simulink model "object_frame_impedance"  (R2025a)
(part 3 of 6)

  + (x1z + (-1) .* x3z) .^ 2) .^ (-1 / 2) .* (x1z + (-1) .* x3z) + ( ...
  (x2x + (-1) .* x4x) .^ 2 + (x2y + (-1) .* x4y) .^ 2 + (x2z + (-1)  ...
  .* x4z) .^ 2) .^ (-1 / 2) .* (x2z + (-1) .* x4z)) + (-1 / 2) .* (( ...
  ((-1) .* x1y + x3y) .* (x2x + (-1) .* x4x) + (x1x + (-1) .* x3x)  ...
  .* (x2y + (-1) .* x4y)) .^ 2 + ((x1z + (-1) .* x3z) .* (x2x + (-1) ...
   .* x4x) + (-1) .* (x1x + (-1) .* x3x) .* (x2z + (-1) .* x4z)) .^  ...
  2 + (((-1) .* x1z + x3z) .* (x2y + (-1) .* x4y) + (x1y + (-1) .*  ...
  x3y) .* (x2z + (-1) .* x4z)) .^ 2) .^ (-1 / 2) .* (((x1x + (-1) .* ...
   x3x) .* ((x1x + (-1) .* x3x) .^ 2 + (x1y + (-1) .* x3y) .^ 2 + ( ...
  x1z + (-1) .* x3z) .^ 2) .^ (-1 / 2) + (x2x + (-1) .* x4x) .* (( ...
  x2x + (-1) .* x4x) .^ 2 + (x2y + (-1) .* x4y) .^ 2 + (x2z + (-1)  ...
  .* x4z) .^ 2) .^ (-1 / 2)) .^ 2 + ((x1y + (-1) .* x3y) .* ((x1x +  ...
  (-1) .* x3x) .^ 2 + (x1y + (-1) .* x3y) .^ 2 + (x1z + (-1) .* x3z) ...
   .^ 2) .^ (-1 / 2) + (x2y + (-1) .* x4y) .* ((x2x + (-1) .* x4x)  ...
  .^ 2 + (x2y + (-1) .* x4y) .^ 2 + (x2z + (-1) .* x4z) .^ 2) .^ ( ...
  -1 / 2)) .^ 2 + (((x1x + (-1) .* x3x) .^ 2 + (x1y + (-1) .* x3y)  ...
  .^ 2 + (x1z + (-1) .* x3z) .^ 2) .^ (-1 / 2) .* (x1z + (-1) .*  ...
  x3z) + ((x2x + (-1) .* x4x) .^ 2 + (x2y + (-1) .* x4y) .^ 2 + ( ...
  x2z + (-1) .* x4z) .^ 2) .^ (-1 / 2) .* (x2z + (-1) .* x4z)) .^ 2) ...
   .^ (-3 / 2) .* ((x1z + (-1) .* x3z) .* (x2x + (-1) .* x4x) + (-1) ...
   .* (x1x + (-1) .* x3x) .* (x2z + (-1) .* x4z)) .* (2 .* ((x2x + ( ...
  -1) .* x4x) .^ 2 .* ((x2x + (-1) .* x4x) .^ 2 + (x2y + (-1) .*  ...
  x4y) .^ 2 + (x2z + (-1) .* x4z) .^ 2) .^ (-3 / 2) + (-1) .* ((x2x  ...
  + (-1) .* x4x) .^ 2 + (x2y + (-1) .* x4y) .^ 2 + (x2z + (-1) .*  ...
  x4z) .^ 2) .^ (-1 / 2)) .* ((x1x + (-1) .* x3x) .* ((x1x + (-1) .* ...
   x3x) .^ 2 + (x1y + (-1) .* x3y) .^ 2 + (x1z + (-1) .* x3z) .^ 2)  ...
  .^ (-1 / 2) + (x2x + (-1) .* x4x) .* ((x2x + (-1) .* x4x) .^ 2 + ( ...
  x2y + (-1) .* x4y) .^ 2 + (x2z + (-1) .* x4z) .^ 2) .^ (-1 / 2)) + ...
   2 .* (x2x + (-1) .* x4x) .* (x2y + (-1) .* x4y) .* ((x1y + (-1)  ...
  .* x3y) .* ((x1x + (-1) .* x3x) .^ 2 + (x1y + (-1) .* x3y) .^ 2 +  ...
  (x1z + (-1) .* x3z) .^ 2) .^ (-1 / 2) + (x2y + (-1) .* x4y) .* (( ...
  x2x + (-1) .* x4x) .^ 2 + (x2y + (-1) .* x4y) .^ 2 + (x2z + (-1)  ...
  .* x4z) .^ 2) .^ (-1 / 2)) .* ((x2x + (-1) .* x4x) .^ 2 + (x2y + ( ...
  -1) .* x4y) .^ 2 + (x2z + (-1) .* x4z) .^ 2) .^ (-3 / 2) + 2 .* ( ...
  x2x + (-1) .* x4x) .* (((x1x + (-1) .* x3x) .^ 2 + (x1y + (-1) .*  ...
  x3y) .^ 2 + (x1z + (-1) .* x3z) .^ 2) .^ (-1 / 2) .* (x1z + (-1)  ...
  .* x3z) + ((x2x + (-1) .* x4x) .^ 2 + (x2y + (-1) .* x4y) .^ 2 + ( ...
  x2z + (-1) .* x4z) .^ 2) .^ (-1 / 2) .* (x2z + (-1) .* x4z)) .* (( ...
  x2x + (-1) .* x4x) .^ 2 + (x2y + (-1) .* x4y) .^ 2 + (x2z + (-1)  ...
  .* x4z) .^ 2) .^ (-3 / 2) .* (x2z + (-1) .* x4z)) .* (((x1x + (-1) ...
   .* x3x) .^ 2 + (x1y + (-1) .* x3y) .^ 2 + (x1z + (-1) .* x3z) .^  ...
  2) .^ (-1 / 2) .* (x1z + (-1) .* x3z) + ((x2x + (-1) .* x4x) .^ 2  ...
  + (x2y + (-1) .* x4y) .^ 2 + (x2z + (-1) .* x4z) .^ 2) .^ (-1 / 2) ...
   .* (x2z + (-1) .* x4z)) + (-1) .* (x2x + (-1) .* x4x) .* (((-1)  ...
  .* x1y + x3y) .* (x2x + (-1) .* x4x) + (x1x + (-1) .* x3x) .* ( ...
  x2y + (-1) .* x4y)) .* (x2y + (-1) .* x4y) .* ((((-1) .* x1y +  ...
  x3y) .* (x2x + (-1) .* x4x) + (x1x + (-1) .* x3x) .* (x2y + (-1)  ...
  .* x4y)) .^ 2 + ((x1z + (-1) .* x3z) .* (x2x + (-1) .* x4x) + (-1) ...
   .* (x1x + (-1) .* x3x) .* (x2z + (-1) .* x4z)) .^ 2 + (((-1) .*  ...
  x1z + x3z) .* (x2y + (-1) .* x4y) + (x1y + (-1) .* x3y) .* (x2z +  ...
  (-1) .* x4z)) .^ 2) .^ (-1 / 2) .* (((x1x + (-1) .* x3x) .* ((x1x  ...
  + (-1) .* x3x) .^ 2 + (x1y + (-1) .* x3y) .^ 2 + (x1z + (-1) .*  ...
  x3z) .^ 2) .^ (-1 / 2) + (x2x + (-1) .* x4x) .* ((x2x + (-1) .*  ...
  x4x) .^ 2 + (x2y + (-1) .* x4y) .^ 2 + (x2z + (-1) .* x4z) .^ 2)  ...
  .^ (-1 / 2)) .^ 2 + ((x1y + (-1) .* x3y) .* ((x1x + (-1) .* x3x)  ...
  .^ 2 + (x1y + (-1) .* x3y) .^ 2 + (x1z + (-1) .* x3z) .^ 2) .^ ( ...
  -1 / 2) + (x2y + (-1) .* x4y) .* ((x2x + (-1) .* x4x) .^ 2 + (x2y  ...
  + (-1) .* x4y) .^ 2 + (x2z + (-1) .* x4z) .^ 2) .^ (-1 / 2)) .^ 2  ...
  + (((x1x + (-1) .* x3x) .^ 2 + (x1y + (-1) .* x3y) .^ 2 + (x1z + ( ...
  -1) .* x3z) .^ 2) .^ (-1 / 2) .* (x1z + (-1) .* x3z) + ((x2x + ( ...
  -1) .* x4x) .^ 2 + (x2y + (-1) .* x4y) .^ 2 + (x2z + (-1) .* x4z)  ...
  .^ 2) .^ (-1 / 2) .* (x2z + (-1) .* x4z)) .^ 2) .^ (-1 / 2) .* (( ...
  x2x + (-1) .* x4x) .^ 2 + (x2y + (-1) .* x4y) .^ 2 + (x2z + (-1)  ...
  .* x4z) .^ 2) .^ (-3 / 2) + (x2x + (-1) .* x4x) .* ((((-1) .* x1y  ...
  + x3y) .* (x2x + (-1) .* x4x) + (x1x + (-1) .* x3x) .* (x2y + (-1) ...
   .* x4y)) .^ 2 + ((x1z + (-1) .* x3z) .* (x2x + (-1) .* x4x) + ( ...
  -1) .* (x1x + (-1) .* x3x) .* (x2z + (-1) .* x4z)) .^ 2 + (((-1)  ...
  .* x1z + x3z) .* (x2y + (-1) .* x4y) + (x1y + (-1) .* x3y) .* ( ...
  x2z + (-1) .* x4z)) .^ 2) .^ (-1 / 2) .* (((x1x + (-1) .* x3x) .*  ...
  ((x1x + (-1) .* x3x) .^ 2 + (x1y + (-1) .* x3y) .^ 2 + (x1z + (-1) ...
   .* x3z) .^ 2) .^ (-1 / 2) + (x2x + (-1) .* x4x) .* ((x2x + (-1)  ...
  .* x4x) .^ 2 + (x2y + (-1) .* x4y) .^ 2 + (x2z + (-1) .* x4z) .^  ...
  2) .^ (-1 / 2)) .^ 2 + ((x1y + (-1) .* x3y) .* ((x1x + (-1) .*  ...
  x3x) .^ 2 + (x1y + (-1) .* x3y) .^ 2 + (x1z + (-1) .* x3z) .^ 2)  ...
  .^ (-1 / 2) + (x2y + (-1) .* x4y) .* ((x2x + (-1) .* x4x) .^ 2 + ( ...
  x2y + (-1) .* x4y) .^ 2 + (x2z + (-1) .* x4z) .^ 2) .^ (-1 / 2))  ...
  .^ 2 + (((x1x + (-1) .* x3x) .^ 2 + (x1y + (-1) .* x3y) .^ 2 + ( ...
  x1z + (-1) .* x3z) .^ 2) .^ (-1 / 2) .* (x1z + (-1) .* x3z) + (( ...
  x2x + (-1) .* x4x) .^ 2 + (x2y + (-1) .* x4y) .^ 2 + (x2z + (-1)  ...
  .* x4z) .^ 2) .^ (-1 / 2) .* (x2z + (-1) .* x4z)) .^ 2) .^ (-1 /  ...
  2) .* ((x1z + (-1) .* x3z) .* (x2x + (-1) .* x4x) + (-1) .* (x1x + ...
   (-1) .* x3x) .* (x2z + (-1) .* x4z)) .* ((x2x + (-1) .* x4x) .^  ...
  2 + (x2y + (-1) .* x4y) .^ 2 + (x2z + (-1) .* x4z) .^ 2) .^ (-3 /  ...
  2) .* (x2z + (-1) .* x4z),(-1) .* (((-1) .* x1y + x3y) .* (x2x + ( ...
  -1) .* x4x) + (x1x + (-1) .* x3x) .* (x2y + (-1) .* x4y)) .* (((( ...
  -1) .* x1y + x3y) .* (x2x + (-1) .* x4x) + (x1x + (-1) .* x3x) .*  ...
  (x2y + (-1) .* x4y)) .^ 2 + ((x1z + (-1) .* x3z) .* (x2x + (-1) .* ...
   x4x) + (-1) .* (x1x + (-1) .* x3x) .* (x2z + (-1) .* x4z)) .^ 2 + ...
   (((-1) .* x1z + x3z) .* (x2y + (-1) .* x4y) + (x1y + (-1) .* x3y) ...
   .* (x2z + (-1) .* x4z)) .^ 2) .^ (-1 / 2) .* (((x1x + (-1) .*  ...
  x3x) .* ((x1x + (-1) .* x3x) .^ 2 + (x1y + (-1) .* x3y) .^ 2 + ( ...
  x1z + (-1) .* x3z) .^ 2) .^ (-1 / 2) + (x2x + (-1) .* x4x) .* (( ...
  x2x + (-1) .* x4x) .^ 2 + (x2y + (-1) .* x4y) .^ 2 + (x2z + (-1)  ...
  .* x4z) .^ 2) .^ (-1 / 2)) .^ 2 + ((x1y + (-1) .* x3y) .* ((x1x +  ...
  (-1) .* x3x) .^ 2 + (x1y + (-1) .* x3y) .^ 2 + (x1z + (-1) .* x3z) ...
   .^ 2) .^ (-1 / 2) + (x2y + (-1) .* x4y) .* ((x2x + (-1) .* x4x)  ...
  .^ 2 + (x2y + (-1) .* x4y) .^ 2 + (x2z + (-1) .* x4z) .^ 2) .^ ( ...
  -1 / 2)) .^ 2 + (((x1x + (-1) .* x3x) .^ 2 + (x1y + (-1) .* x3y)  ...
  .^ 2 + (x1z + (-1) .* x3z) .^ 2) .^ (-1 / 2) .* (x1z + (-1) .*  ...
  x3z) + ((x2x + (-1) .* x4x) .^ 2 + (x2y + (-1) .* x4y) .^ 2 + ( ...
  x2z + (-1) .* x4z) .^ 2) .^ (-1 / 2) .* (x2z + (-1) .* x4z)) .^ 2) ...
   .^ (-1 / 2) .* ((x2y + (-1) .* x4y) .^ 2 .* ((x2x + (-1) .* x4x)  ...
  .^ 2 + (x2y + (-1) .* x4y) .^ 2 + (x2z + (-1) .* x4z) .^ 2) .^ ( ...
  -3 / 2) + (-1) .* ((x2x + (-1) .* x4x) .^ 2 + (x2y + (-1) .* x4y)  ...
  .^ 2 + (x2z + (-1) .* x4z) .^ 2) .^ (-1 / 2)) + (1 / 2) .* (((-1)  ...
  .* x1y + x3y) .* (x2x + (-1) .* x4x) + (x1x + (-1) .* x3x) .* ( ...
  x2y + (-1) .* x4y)) .* (2 .* ((-1) .* x1x + x3x) .* (((-1) .* x1y  ...
  + x3y) .* (x2x + (-1) .* x4x) + (x1x + (-1) .* x3x) .* (x2y + (-1) ...
   .* x4y)) + 2 .* (x1z + (-1) .* x3z) .* (((-1) .* x1z + x3z) .* ( ...
  x2y + (-1) .* x4y) + (x1y + (-1) .* x3y) .* (x2z + (-1) .* x4z)))  ...
  .* ((((-1) .* x1y + x3y) .* (x2x + (-1) .* x4x) + (x1x + (-1) .*  ...
  x3x) .* (x2y + (-1) .* x4y)) .^ 2 + ((x1z + (-1) .* x3z) .* (x2x + ...
   (-1) .* x4x) + (-1) .* (x1x + (-1) .* x3x) .* (x2z + (-1) .* x4z) ...
  ) .^ 2 + (((-1) .* x1z + x3z) .* (x2y + (-1) .* x4y) + (x1y + (-1) ...
   .* x3y) .* (x2z + (-1) .* x4z)) .^ 2) .^ (-3 / 2) .* (((x1x + ( ...
  -1) .* x3x) .* ((x1x + (-1) .* x3x) .^ 2 + (x1y + (-1) .* x3y) .^  ...
  2 + (x1z + (-1) .* x3z) .^ 2) .^ (-1 / 2) + (x2x + (-1) .* x4x) .* ...
   ((x2x + (-1) .* x4x) .^ 2 + (x2y + (-1) .* x4y) .^ 2 + (x2z + ( ...
  -1) .* x4z) .^ 2) .^ (-1 / 2)) .^ 2 + ((x1y + (-1) .* x3y) .* (( ...
  x1x + (-1) .* x3x) .^ 2 + (x1y + (-1) .* x3y) .^ 2 + (x1z + (-1)  ...
  .* x3z) .^ 2) .^ (-1 / 2) + (x2y + (-1) .* x4y) .* ((x2x + (-1) .* ...
   x4x) .^ 2 + (x2y + (-1) .* x4y) .^ 2 + (x2z + (-1) .* x4z) .^ 2)  ...
  .^ (-1 / 2)) .^ 2 + (((x1x + (-1) .* x3x) .^ 2 + (x1y + (-1) .*  ...
  x3y) .^ 2 + (x1z + (-1) .* x3z) .^ 2) .^ (-1 / 2) .* (x1z + (-1)  ...
  .* x3z) + ((x2x + (-1) .* x4x) .^ 2 + (x2y + (-1) .* x4y) .^ 2 + ( ...
  x2z + (-1) .* x4z) .^ 2) .^ (-1 / 2) .* (x2z + (-1) .* x4z)) .^ 2) ...
   .^ (-1 / 2) .* ((x1y + (-1) .* x3y) .* ((x1x + (-1) .* x3x) .^ 2  ...
  + (x1y + (-1) .* x3y) .^ 2 + (x1z + (-1) .* x3z) .^ 2) .^ (-1 / 2) ...
   + (x2y + (-1) .* x4y) .* ((x2x + (-1) .* x4x) .^ 2 + (x2y + (-1)  ...
  .* x4y) .^ 2 + (x2z + (-1) .* x4z) .^ 2) .^ (-1 / 2)) + (-1) .* (( ...
  -1) .* x1x + x3x) .* ((((-1) .* x1y + x3y) .* (x2x + (-1) .* x4x)  ...
  + (x1x + (-1) .* x3x) .* (x2y + (-1) .* x4y)) .^ 2 + ((x1z + (-1)  ...
  .* x3z) .* (x2x + (-1) .* x4x) + (-1) .* (x1x + (-1) .* x3x) .* ( ...
  x2z + (-1) .* x4z)) .^ 2 + (((-1) .* x1z + x3z) .* (x2y + (-1) .*  ...
  x4y) + (x1y + (-1) .* x3y) .* (x2z + (-1) .* x4z)) .^ 2) .^ (-1 /  ...
  2) .* (((x1x + (-1) .* x3x) .* ((x1x + (-1) .* x3x) .^ 2 + (x1y +  ...
  (-1) .* x3y) .^ 2 + (x1z + (-1) .* x3z) .^ 2) .^ (-1 / 2) + (x2x + ...
   (-1) .* x4x) .* ((x2x + (-1) .* x4x) .^ 2 + (x2y + (-1) .* x4y)  ...
  .^ 2 + (x2z + (-1) .* x4z) .^ 2) .^ (-1 / 2)) .^ 2 + ((x1y + (-1)  ...
  .* x3y) .* ((x1x + (-1) .* x3x) .^ 2 + (x1y + (-1) .* x3y) .^ 2 +  ...
  (x1z + (-1) .* x3z) .^ 2) .^ (-1 / 2) + (x2y + (-1) .* x4y) .* (( ...
  x2x + (-1) .* x4x) .^ 2 + (x2y + (-1) .* x4y) .^ 2 + (x2z + (-1)  ...
  .* x4z) .^ 2) .^ (-1 / 2)) .^ 2 + (((x1x + (-1) .* x3x) .^ 2 + ( ...
  x1y + (-1) .* x3y) .^ 2 + (x1z + (-1) .* x3z) .^ 2) .^ (-1 / 2) .* ...
   (x1z + (-1) .* x3z) + ((x2x + (-1) .* x4x) .^ 2 + (x2y + (-1) .*  ...
  x4y) .^ 2 + (x2z + (-1) .* x4z) .^ 2) .^ (-1 / 2) .* (x2z + (-1)  ...
  .* x4z)) .^ 2) .^ (-1 / 2) .* ((x1y + (-1) .* x3y) .* ((x1x + (-1) ...
   .* x3x) .^ 2 + (x1y + (-1) .* x3y) .^ 2 + (x1z + (-1) .* x3z) .^  ...
  2) .^ (-1 / 2) + (x2y + (-1) .* x4y) .* ((x2x + (-1) .* x4x) .^ 2  ...
  + (x2y + (-1) .* x4y) .^ 2 + (x2z + (-1) .* x4z) .^ 2) .^ (-1 / 2) ...
  ) + (1 / 2) .* (((-1) .* x1y + x3y) .* (x2x + (-1) .* x4x) + (x1x  ...
  + (-1) .* x3x) .* (x2y + (-1) .* x4y)) .* ((((-1) .* x1y + x3y) .* ...
   (x2x + (-1) .* x4x) + (x1x + (-1) .* x3x) .* (x2y + (-1) .* x4y)) ...
   .^ 2 + ((x1z + (-1) .* x3z) .* (x2x + (-1) .* x4x) + (-1) .* ( ...
  x1x + (-1) .* x3x) .* (x2z + (-1) .* x4z)) .^ 2 + (((-1) .* x1z +  ...
  x3z) .* (x2y + (-1) .* x4y) + (x1y + (-1) .* x3y) .* (x2z + (-1)  ...
  .* x4z)) .^ 2) .^ (-1 / 2) .* (((x1x + (-1) .* x3x) .* ((x1x + ( ...
  -1) .* x3x) .^ 2 + (x1y + (-1) .* x3y) .^ 2 + (x1z + (-1) .* x3z)  ...
  .^ 2) .^ (-1 / 2) + (x2x + (-1) .* x4x) .* ((x2x + (-1) .* x4x)  ...
  .^ 2 + (x2y + (-1) .* x4y) .^ 2 + (x2z + (-1) .* x4z) .^ 2) .^ ( ...
  -1 / 2)) .^ 2 + ((x1y + (-1) .* x3y) .* ((x1x + (-1) .* x3x) .^ 2  ...
  + (x1y + (-1) .* x3y) .^ 2 + (x1z + (-1) .* x3z) .^ 2) .^ (-1 / 2) ...
   + (x2y + (-1) .* x4y) .* ((x2x + (-1) .* x4x) .^ 2 + (x2y + (-1)  ...
  .* x4y) .^ 2 + (x2z + (-1) .* x4z) .^ 2) .^ (-1 / 2)) .^ 2 + ((( ...
  x1x + (-1) .* x3x) .^ 2 + (x1y + (-1) .* x3y) .^ 2 + (x1z + (-1)  ...
  .* x3z) .^ 2) .^ (-1 / 2) .* (x1z + (-1) .* x3z) + ((x2x + (-1) .* ...
   x4x) .^ 2 + (x2y + (-1) .* x4y) .^ 2 + (x2z + (-1) .* x4z) .^ 2)  ...
  .^ (-1 / 2) .* (x2z + (-1) .* x4z)) .^ 2) .^ (-3 / 2) .* ((x1y + ( ...
  -1) .* x3y) .* ((x1x + (-1) .* x3x) .^ 2 + (x1y + (-1) .* x3y) .^  ...
  2 + (x1z + (-1) .* x3z) .^ 2) .^ (-1 / 2) + (x2y + (-1) .* x4y) .* ...
   ((x2x + (-1) .* x4x) .^ 2 + (x2y + (-1) .* x4y) .^ 2 + (x2z + ( ...
  -1) .* x4z) .^ 2) .^ (-1 / 2)) .* (2 .* ((x2y + (-1) .* x4y) .^ 2  ...
  .* ((x2x + (-1) .* x4x) .^ 2 + (x2y + (-1) .* x4y) .^ 2 + (x2z + ( ...
  -1) .* x4z) .^ 2) .^ (-3 / 2) + (-1) .* ((x2x + (-1) .* x4x) .^ 2  ...
  + (x2y + (-1) .* x4y) .^ 2 + (x2z + (-1) .* x4z) .^ 2) .^ (-1 / 2) ...
  ) .* ((x1y + (-1) .* x3y) .* ((x1x + (-1) .* x3x) .^ 2 + (x1y + ( ...
  -1) .* x3y) .^ 2 + (x1z + (-1) .* x3z) .^ 2) .^ (-1 / 2) + (x2y +  ...
  (-1) .* x4y) .* ((x2x + (-1) .* x4x) .^ 2 + (x2y + (-1) .* x4y)  ...
  .^ 2 + (x2z + (-1) .* x4z) .^ 2) .^ (-1 / 2)) + 2 .* (x2x + (-1)  ...
  .* x4x) .* (x2y + (-1) .* x4y) .* ((x1x + (-1) .* x3x) .* ((x1x +  ...
  (-1) .* x3x) .^ 2 + (x1y + (-1) .* x3y) .^ 2 + (x1z + (-1) .* x3z) ...
   .^ 2) .^ (-1 / 2) + (x2x + (-1) .* x4x) .* ((x2x + (-1) .* x4x)  ...
  .^ 2 + (x2y + (-1) .* x4y) .^ 2 + (x2z + (-1) .* x4z) .^ 2) .^ ( ...
  -1 / 2)) .* ((x2x + (-1) .* x4x) .^ 2 + (x2y + (-1) .* x4y) .^ 2 + ...
   (x2z + (-1) .* x4z) .^ 2) .^ (-3 / 2) + 2 .* (x2y + (-1) .* x4y)  ...
  .* (((x1x + (-1) .* x3x) .^ 2 + (x1y + (-1) .* x3y) .^ 2 + (x1z +  ...
  (-1) .* x3z) .^ 2) .^ (-1 / 2) .* (x1z + (-1) .* x3z) + ((x2x + ( ...
  -1) .* x4x) .^ 2 + (x2y + (-1) .* x4y) .^ 2 + (x2z + (-1) .* x4z)  ...
  .^ 2) .^ (-1 / 2) .* (x2z + (-1) .* x4z)) .* ((x2x + (-1) .* x4x)  ...
  .^ 2 + (x2y + (-1) .* x4y) .^ 2 + (x2z + (-1) .* x4z) .^ 2) .^ ( ...
  -3 / 2) .* (x2z + (-1) .* x4z)) + (-1 / 2) .* (2 .* ((-1) .* x1x + ...
   x3x) .* (((-1) .* x1y + x3y) .* (x2x + (-1) .* x4x) + (x1x + (-1) ...
   .* x3x) .* (x2y + (-1) .* x4y)) + 2 .* (x1z + (-1) .* x3z) .* ((( ...
  -1) .* x1z + x3z) .* (x2y + (-1) .* x4y) + (x1y + (-1) .* x3y) .*  ...
  (x2z + (-1) .* x4z))) .* ((((-1) .* x1y + x3y) .* (x2x + (-1) .*  ...
  x4x) + (x1x + (-1) .* x3x) .* (x2y + (-1) .* x4y)) .^ 2 + ((x1z +  ...
  (-1) .* x3z) .* (x2x + (-1) .* x4x) + (-1) .* (x1x + (-1) .* x3x)  ...
  .* (x2z + (-1) .* x4z)) .^ 2 + (((-1) .* x1z + x3z) .* (x2y + (-1) ...
   .* x4y) + (x1y + (-1) .* x3y) .* (x2z + (-1) .* x4z)) .^ 2) .^ ( ...
  -3 / 2) .* (((x1x + (-1) .* x3x) .* ((x1x + (-1) .* x3x) .^ 2 + ( ...
  x1y + (-1) .* x3y) .^ 2 + (x1z + (-1) .* x3z) .^ 2) .^ (-1 / 2) +  ...
  (x2x + (-1) .* x4x) .* ((x2x + (-1) .* x4x) .^ 2 + (x2y + (-1) .*  ...
  x4y) .^ 2 + (x2z + (-1) .* x4z) .^ 2) .^ (-1 / 2)) .^ 2 + ((x1y +  ...
  (-1) .* x3y) .* ((x1x + (-1) .* x3x) .^ 2 + (x1y + (-1) .* x3y)  ...
  .^ 2 + (x1z + (-1) .* x3z) .^ 2) .^ (-1 / 2) + (x2y + (-1) .* x4y) ...
   .* ((x2x + (-1) .* x4x) .^ 2 + (x2y + (-1) .* x4y) .^ 2 + (x2z +  ...
  (-1) .* x4z) .^ 2) .^ (-1 / 2)) .^ 2 + (((x1x + (-1) .* x3x) .^ 2  ...
  + (x1y + (-1) .* x3y) .^ 2 + (x1z + (-1) .* x3z) .^ 2) .^ (-1 / 2) ...
   .* (x1z + (-1) .* x3z) + ((x2x + (-1) .* x4x) .^ 2 + (x2y + (-1)  ...
  .* x4y) .^ 2 + (x2z + (-1) .* x4z) .^ 2) .^ (-1 / 2) .* (x2z + ( ...
  -1) .* x4z)) .^ 2) .^ (-1 / 2) .* ((x1z + (-1) .* x3z) .* (x2x + ( ...
  -1) .* x4x) + (-1) .* (x1x + (-1) .* x3x) .* (x2z + (-1) .* x4z))  ...
  .* (((x1x + (-1) .* x3x) .^ 2 + (x1y + (-1) .* x3y) .^ 2 + (x1z +  ...
  (-1) .* x3z) .^ 2) .^ (-1 / 2) .* (x1z + (-1) .* x3z) + ((x2x + ( ...
  -1) .* x4x) .^ 2 + (x2y + (-1) .* x4y) .^ 2 + (x2z + (-1) .* x4z)  ...
  .^ 2) .^ (-1 / 2) .* (x2z + (-1) .* x4z)) + (-1 / 2) .* ((((-1) .* ...
   x1y + x3y) .* (x2x + (-1) .* x4x) + (x1x + (-1) .* x3x) .* (x2y + ...
   (-1) .* x4y)) .^ 2 + ((x1z + (-1) .* x3z) .* (x2x + (-1) .* x4x)  ...
  + (-1) .* (x1x + (-1) .* x3x) .* (x2z + (-1) .* x4z)) .^ 2 + ((( ...
  -1) .* x1z + x3z) .* (x2y + (-1) .* x4y) + (x1y + (-1) .* x3y) .*  ...
  (x2z + (-1) .* x4z)) .^ 2) .^ (-1 / 2) .* (((x1x + (-1) .* x3x) .* ...
   ((x1x + (-1) .* x3x) .^ 2 + (x1y + (-1) .* x3y) .^ 2 + (x1z + ( ...
  -1) .* x3z) .^ 2) .^ (-1 / 2) + (x2x + (-1) .* x4x) .* ((x2x + ( ...
  -1) .* x4x) .^ 2 + (x2y + (-1) .* x4y) .^ 2 + (x2z + (-1) .* x4z)  ...
  .^ 2) .^ (-1 / 2)) .^ 2 + ((x1y + (-1) .* x3y) .* ((x1x + (-1) .*  ...
  x3x) .^ 2 + (x1y + (-1) .* x3y) .^ 2 + (x1z + (-1) .* x3z) .^ 2)  ...
  .^ (-1 / 2) + (x2y + (-1) .* x4y) .* ((x2x + (-1) .* x4x) .^ 2 + ( ...
  x2y + (-1) .* x4y) .^ 2 + (x2z + (-1) .* x4z) .^ 2) .^ (-1 / 2))  ...
  .^ 2 + (((x1x + (-1) .* x3x) .^ 2 + (x1y + (-1) .* x3y) .^ 2 + ( ...
  x1z + (-1) .* x3z) .^ 2) .^ (-1 / 2) .* (x1z + (-1) .* x3z) + (( ...
  x2x + (-1) .* x4x) .^ 2 + (x2y + (-1) .* x4y) .^ 2 + (x2z + (-1)  ...
  .* x4z) .^ 2) .^ (-1 / 2) .* (x2z + (-1) .* x4z)) .^ 2) .^ (-3 /  ...
  2) .* ((x1z + (-1) .* x3z) .* (x2x + (-1) .* x4x) + (-1) .* (x1x + ...
   (-1) .* x3x) .* (x2z + (-1) .* x4z)) .* (2 .* ((x2y + (-1) .*  ...
  x4y) .^ 2 .* ((x2x + (-1) .* x4x) .^ 2 + (x2y + (-1) .* x4y) .^ 2  ...
  + (x2z + (-1) .* x4z) .^ 2) .^ (-3 / 2) + (-1) .* ((x2x + (-1) .*  ...
  x4x) .^ 2 + (x2y + (-1) .* x4y) .^ 2 + (x2z + (-1) .* x4z) .^ 2)  ...
  .^ (-1 / 2)) .* ((x1y + (-1) .* x3y) .* ((x1x + (-1) .* x3x) .^ 2  ...
  + (x1y + (-1) .* x3y) .^ 2 + (x1z + (-1) .* x3z) .^ 2) .^ (-1 / 2) ...
   + (x2y + (-1) .* x4y) .* ((x2x + (-1) .* x4x) .^ 2 + (x2y + (-1)  ...
  .* x4y) .^ 2 + (x2z + (-1) .* x4z) .^ 2) .^ (-1 / 2)) + 2 .* (x2x  ...
  + (-1) .* x4x) .* (x2y + (-1) .* x4y) .* ((x1x + (-1) .* x3x) .* ( ...
  (x1x + (-1) .* x3x) .^ 2 + (x1y + (-1) .* x3y) .^ 2 + (x1z + (-1)  ...
  .* x3z) .^ 2) .^ (-1 / 2) + (x2x + (-1) .* x4x) .* ((x2x + (-1) .* ...
   x4x) .^ 2 + (x2y + (-1) .* x4y) .^ 2 + (x2z + (-1) .* x4z) .^ 2)  ...
  .^ (-1 / 2)) .* ((x2x + (-1) .* x4x) .^ 2 + (x2y + (-1) .* x4y)  ...
  .^ 2 + (x2z + (-1) .* x4z) .^ 2) .^ (-3 / 2) + 2 .* (x2y + (-1) .* ...
   x4y) .* (((x1x + (-1) .* x3x) .^ 2 + (x1y + (-1) .* x3y) .^ 2 + ( ...
  x1z + (-1) .* x3z) .^ 2) .^ (-1 / 2) .* (x1z + (-1) .* x3z) + (( ...
  x2x + (-1) .* x4x) .^ 2 + (x2y + (-1) .* x4y) .^ 2 + (x2z + (-1)  ...
  .* x4z) .^ 2) .^ (-1 / 2) .* (x2z + (-1) .* x4z)) .* ((x2x + (-1)  ...
  .* x4x) .^ 2 + (x2y + (-1) .* x4y) .^ 2 + (x2z + (-1) .* x4z) .^  ...
  2) .^ (-3 / 2) .* (x2z + (-1) .* x4z)) .* (((x1x + (-1) .* x3x)  ...
  .^ 2 + (x1y + (-1) .* x3y) .^ 2 + (x1z + (-1) .* x3z) .^ 2) .^ ( ...
  -1 / 2) .* (x1z + (-1) .* x3z) + ((x2x + (-1) .* x4x) .^ 2 + (x2y  ...
  + (-1) .* x4y) .^ 2 + (x2z + (-1) .* x4z) .^ 2) .^ (-1 / 2) .* ( ...
  x2z + (-1) .* x4z)) + (x2y + (-1) .* x4y) .* ((((-1) .* x1y + x3y) ...
   .* (x2x + (-1) .* x4x) + (x1x + (-1) .* x3x) .* (x2y + (-1) .*  ...
  x4y)) .^ 2 + ((x1z + (-1) .* x3z) .* (x2x + (-1) .* x4x) + (-1) .* ...
   (x1x + (-1) .* x3x) .* (x2z + (-1) .* x4z)) .^ 2 + (((-1) .* x1z  ...
  + x3z) .* (x2y + (-1) .* x4y) + (x1y + (-1) .* x3y) .* (x2z + (-1) ...
   .* x4z)) .^ 2) .^ (-1 / 2) .* (((x1x + (-1) .* x3x) .* ((x1x + ( ...
  -1) .* x3x) .^ 2 + (x1y + (-1) .* x3y) .^ 2 + (x1z + (-1) .* x3z)  ...
  .^ 2) .^ (-1 / 2) + (x2x + (-1) .* x4x) .* ((x2x + (-1) .* x4x)  ...
  .^ 2 + (x2y + (-1) .* x4y) .^ 2 + (x2z + (-1) .* x4z) .^ 2) .^ ( ...
  -1 / 2)) .^ 2 + ((x1y + (-1) .* x3y) .* ((x1x + (-1) .* x3x) .^ 2  ...
  + (x1y + (-1) .* x3y) .^ 2 + (x1z + (-1) .* x3z) .^ 2) .^ (-1 / 2) ...
   + (x2y + (-1) .* x4y) .* ((x2x + (-1) .* x4x) .^ 2 + (x2y + (-1)  ...
  .* x4y) .^ 2 + (x2z + (-1) .* x4z) .^ 2) .^ (-1 / 2)) .^ 2 + ((( ...
  x1x + (-1) .* x3x) .^ 2 + (x1y + (-1) .* x3y) .^ 2 + (x1z + (-1)  ...
  .* x3z) .^ 2) .^ (-1 / 2) .* (x1z + (-1) .* x3z) + ((x2x + (-1) .* ...
   x4x) .^ 2 + (x2y + (-1) .* x4y) .^ 2 + (x2z + (-1) .* x4z) .^ 2)  ...
  .^ (-1 / 2) .* (x2z + (-1) .* x4z)) .^ 2) .^ (-1 / 2) .* ((x1z + ( ...
  -1) .* x3z) .* (x2x + (-1) .* x4x) + (-1) .* (x1x + (-1) .* x3x)  ...
  .* (x2z + (-1) .* x4z)) .* ((x2x + (-1) .* x4x) .^ 2 + (x2y + (-1) ...
   .* x4y) .^ 2 + (x2z + (-1) .* x4z) .^ 2) .^ (-3 / 2) .* (x2z + ( ...
  -1) .* x4z),(1 / 2) .* (((-1) .* x1y + x3y) .* (x2x + (-1) .* x4x) ...
   + (x1x + (-1) .* x3x) .* (x2y + (-1) .* x4y)) .* (2 .* (x1x + ( ...
  -1) .* x3x) .* ((x1z + (-1) .* x3z) .* (x2x + (-1) .* x4x) + (-1)  ...
  .* (x1x + (-1) .* x3x) .* (x2z + (-1) .* x4z)) + 2 .* ((-1) .*  ...
  x1y + x3y) .* (((-1) .* x1z + x3z) .* (x2y + (-1) .* x4y) + (x1y + ...
   (-1) .* x3y) .* (x2z + (-1) .* x4z))) .* ((((-1) .* x1y + x3y) .* ...
   (x2x + (-1) .* x4x) + (x1x + (-1) .* x3x) .* (x2y + (-1) .* x4y)) ...
   .^ 2 + ((x1z + (-1) .* x3z) .* (x2x + (-1) .* x4x) + (-1) .* ( ...
  x1x + (-1) .* x3x) .* (x2z + (-1) .* x4z)) .^ 2 + (((-1) .* x1z +  ...
  x3z) .* (x2y + (-1) .* x4y) + (x1y + (-1) .* x3y) .* (x2z + (-1)  ...
  .* x4z)) .^ 2) .^ (-3 / 2) .* (((x1x + (-1) .* x3x) .* ((x1x + ( ...
  -1) .* x3x) .^ 2 + (x1y + (-1) .* x3y) .^ 2 + (x1z + (-1) .* x3z)  ...
  .^ 2) .^ (-1 / 2) + (x2x + (-1) .* x4x) .* ((x2x + (-1) .* x4x)  ...
  .^ 2 + (x2y + (-1) .* x4y) .^ 2 + (x2z + (-1) .* x4z) .^ 2) .^ ( ...
  -1 / 2)) .^ 2 + ((x1y + (-1) .* x3y) .* ((x1x + (-1) .* x3x) .^ 2  ...
  + (x1y + (-1) .* x3y) .^ 2 + (x1z + (-1) .* x3z) .^ 2) .^ (-1 / 2) ...
   + (x2y + (-1) .* x4y) .* ((x2x + (-1) .* x4x) .^ 2 + (x2y + (-1)  ...
  .* x4y) .^ 2 + (x2z + (-1) .* x4z) .^ 2) .^ (-1 / 2)) .^ 2 + ((( ...
  x1x + (-1) .* x3x) .^ 2 + (x1y + (-1) .* x3y) .^ 2 + (x1z + (-1)  ...
  .* x3z) .^ 2) .^ (-1 / 2) .* (x1z + (-1) .* x3z) + ((x2x + (-1) .* ...
   x4x) .^ 2 + (x2y + (-1) .* x4y) .^ 2 + (x2z + (-1) .* x4z) .^ 2)  ...
  .^ (-1 / 2) .* (x2z + (-1) .* x4z)) .^ 2) .^ (-1 / 2) .* ((x1y + ( ...
  -1) .* x3y) .* ((x1x + (-1) .* x3x) .^ 2 + (x1y + (-1) .* x3y) .^  ...
  2 + (x1z + (-1) .* x3z) .^ 2) .^ (-1 / 2) + (x2y + (-1) .* x4y) .* ...
   ((x2x + (-1) .* x4x) .^ 2 + (x2y + (-1) .* x4y) .^ 2 + (x2z + ( ...
  -1) .* x4z) .^ 2) .^ (-1 / 2)) + (1 / 2) .* (((-1) .* x1y + x3y)  ...
  .* (x2x + (-1) .* x4x) + (x1x + (-1) .* x3x) .* (x2y + (-1) .*  ...
  x4y)) .* ((((-1) .* x1y + x3y) .* (x2x + (-1) .* x4x) + (x1x + ( ...
  -1) .* x3x) .* (x2y + (-1) .* x4y)) .^ 2 + ((x1z + (-1) .* x3z) .* ...
   (x2x + (-1) .* x4x) + (-1) .* (x1x + (-1) .* x3x) .* (x2z + (-1)  ...
  .* x4z)) .^ 2 + (((-1) .* x1z + x3z) .* (x2y + (-1) .* x4y) + ( ...
  x1y + (-1) .* x3y) .* (x2z + (-1) .* x4z)) .^ 2) .^ (-1 / 2) .* (( ...
  (x1x + (-1) .* x3x) .* ((x1x + (-1) .* x3x) .^ 2 + (x1y + (-1) .*  ...
  x3y) .^ 2 + (x1z + (-1) .* x3z) .^ 2) .^ (-1 / 2) + (x2x + (-1) .* ...
   x4x) .* ((x2x + (-1) .* x4x) .^ 2 + (x2y + (-1) .* x4y) .^ 2 + ( ...
  x2z + (-1) .* x4z) .^ 2) .^ (-1 / 2)) .^ 2 + ((x1y + (-1) .* x3y)  ...
  .* ((x1x + (-1) .* x3x) .^ 2 + (x1y + (-1) .* x3y) .^ 2 + (x1z + ( ...
  -1) .* x3z) .^ 2) .^ (-1 / 2) + (x2y + (-1) .* x4y) .* ((x2x + ( ...
  -1) .* x4x) .^ 2 + (x2y + (-1) .* x4y) .^ 2 + (x2z + (-1) .* x4z)  ...
  .^ 2) .^ (-1 / 2)) .^ 2 + (((x1x + (-1) .* x3x) .^ 2 + (x1y + (-1) ...
   .* x3y) .^ 2 + (x1z + (-1) .* x3z) .^ 2) .^ (-1 / 2) .* (x1z + ( ...
  -1) .* x3z) + ((x2x + (-1) .* x4x) .^ 2 + (x2y + (-1) .* x4y) .^  ...
  2 + (x2z + (-1) .* x4z) .^ 2) .^ (-1 / 2) .* (x2z + (-1) .* x4z))  ...
  .^ 2) .^ (-3 / 2) .* ((x1y + (-1) .* x3y) .* ((x1x + (-1) .* x3x)  ...
  .^ 2 + (x1y + (-1) .* x3y) .^ 2 + (x1z + (-1) .* x3z) .^ 2) .^ ( ...
  -1 / 2) + (x2y + (-1) .* x4y) .* ((x2x + (-1) .* x4x) .^ 2 + (x2y  ...
  + (-1) .* x4y) .^ 2 + (x2z + (-1) .* x4z) .^ 2) .^ (-1 / 2)) .* ( ...
  2 .* (((x1x + (-1) .* x3x) .^ 2 + (x1y + (-1) .* x3y) .^ 2 + (x1z  ...
  + (-1) .* x3z) .^ 2) .^ (-1 / 2) .* (x1z + (-1) .* x3z) + ((x2x +  ...
  (-1) .* x4x) .^ 2 + (x2y + (-1) .* x4y) .^ 2 + (x2z + (-1) .* x4z) ...
   .^ 2) .^ (-1 / 2) .* (x2z + (-1) .* x4z)) .* ((-1) .* ((x2x + ( ...
  -1) .* x4x) .^ 2 + (x2y + (-1) .* x4y) .^ 2 + (x2z + (-1) .* x4z)  ...
  .^ 2) .^ (-1 / 2) + ((x2x + (-1) .* x4x) .^ 2 + (x2y + (-1) .*  ...
  x4y) .^ 2 + (x2z + (-1) .* x4z) .^ 2) .^ (-3 / 2) .* (x2z + (-1)  ...
  .* x4z) .^ 2) + 2 .* (x2x + (-1) .* x4x) .* ((x1x + (-1) .* x3x)  ...
  .* ((x1x + (-1) .* x3x) .^ 2 + (x1y + (-1) .* x3y) .^ 2 + (x1z + ( ...
  -1) .* x3z) .^ 2) .^ (-1 / 2) + (x2x + (-1) .* x4x) .* ((x2x + ( ...
  -1) .* x4x) .^ 2 + (x2y + (-1) .* x4y) .^ 2 + (x2z + (-1) .* x4z)  ...
  .^ 2) .^ (-1 / 2)) .* ((x2x + (-1) .* x4x) .^ 2 + (x2y + (-1) .*  ...
  x4y) .^ 2 + (x2z + (-1) .* x4z) .^ 2) .^ (-3 / 2) .* (x2z + (-1)  ...
  .* x4z) + 2 .* (x2y + (-1) .* x4y) .* ((x1y + (-1) .* x3y) .* (( ...
  x1x + (-1) .* x3x) .^ 2 + (x1y + (-1) .* x3y) .^ 2 + (x1z + (-1)  ...
  .* x3z) .^ 2) .^ (-1 / 2) + (x2y + (-1) .* x4y) .* ((x2x + (-1) .* ...
   x4x) .^ 2 + (x2y + (-1) .* x4y) .^ 2 + (x2z + (-1) .* x4z) .^ 2)  ...
  .^ (-1 / 2)) .* ((x2x + (-1) .* x4x) .^ 2 + (x2y + (-1) .* x4y)  ...
  .^ 2 + (x2z + (-1) .* x4z) .^ 2) .^ (-3 / 2) .* (x2z + (-1) .*  ...
  x4z)) + (x1x + (-1) .* x3x) .* ((((-1) .* x1y + x3y) .* (x2x + ( ...
  -1) .* x4x) + (x1x + (-1) .* x3x) .* (x2y + (-1) .* x4y)) .^ 2 + ( ...
  (x1z + (-1) .* x3z) .* (x2x + (-1) .* x4x) + (-1) .* (x1x + (-1)  ...
  .* x3x) .* (x2z + (-1) .* x4z)) .^ 2 + (((-1) .* x1z + x3z) .* ( ...
  x2y + (-1) .* x4y) + (x1y + (-1) .* x3y) .* (x2z + (-1) .* x4z))  ...
  .^ 2) .^ (-1 / 2) .* (((x1x + (-1) .* x3x) .* ((x1x + (-1) .* x3x) ...
   .^ 2 + (x1y + (-1) .* x3y) .^ 2 + (x1z + (-1) .* x3z) .^ 2) .^ ( ...
  -1 / 2) + (x2x + (-1) .* x4x) .* ((x2x + (-1) .* x4x) .^ 2 + (x2y  ...
  + (-1) .* x4y) .^ 2 + (x2z + (-1) .* x4z) .^ 2) .^ (-1 / 2)) .^ 2  ...
  + ((x1y + (-1) .* x3y) .* ((x1x + (-1) .* x3x) .^ 2 + (x1y + (-1)  ...
  .* x3y) .^ 2 + (x1z + (-1) .* x3z) .^ 2) .^ (-1 / 2) + (x2y + (-1) ...
   .* x4y) .* ((x2x + (-1) .* x4x) .^ 2 + (x2y + (-1) .* x4y) .^ 2 + ...
   (x2z + (-1) .* x4z) .^ 2) .^ (-1 / 2)) .^ 2 + (((x1x + (-1) .*  ...
  x3x) .^ 2 + (x1y + (-1) .* x3y) .^ 2 + (x1z + (-1) .* x3z) .^ 2)  ...
  .^ (-1 / 2) .* (x1z + (-1) .* x3z) + ((x2x + (-1) .* x4x) .^ 2 + ( ...
  x2y + (-1) .* x4y) .^ 2 + (x2z + (-1) .* x4z) .^ 2) .^ (-1 / 2) .* ...
   (x2z + (-1) .* x4z)) .^ 2) .^ (-1 / 2) .* (((x1x + (-1) .* x3x)  ...
  .^ 2 + (x1y + (-1) .* x3y) .^ 2 + (x1z + (-1) .* x3z) .^ 2) .^ ( ...
  -1 / 2) .* (x1z + (-1) .* x3z) + ((x2x + (-1) .* x4x) .^ 2 + (x2y  ...
  + (-1) .* x4y) .^ 2 + (x2z + (-1) .* x4z) .^ 2) .^ (-1 / 2) .* ( ...
  x2z + (-1) .* x4z)) + (-1 / 2) .* (2 .* (x1x + (-1) .* x3x) .* (( ...
  x1z + (-1) .* x3z) .* (x2x + (-1) .* x4x) + (-1) .* (x1x + (-1) .* ...
   x3x) .* (x2z + (-1) .* x4z)) + 2 .* ((-1) .* x1y + x3y) .* (((-1) ...
   .* x1z + x3z) .* (x2y + (-1) .* x4y) + (x1y + (-1) .* x3y) .* ( ...
  x2z + (-1) .* x4z))) .* ((((-1) .* x1y + x3y) .* (x2x + (-1) .*  ...
  x4x) + (x1x + (-1) .* x3x) .* (x2y + (-1) .* x4y)) .^ 2 + ((x1z +  ...
  (-1) .* x3z) .* (x2x + (-1) .* x4x) + (-1) .* (x1x + (-1) .* x3x)  ...
  .* (x2z + (-1) .* x4z)) .^ 2 + (((-1) .* x1z + x3z) .* (x2y + (-1) ...
   .* x4y) + (x1y + (-1) .* x3y) .* (x2z + (-1) .* x4z)) .^ 2) .^ ( ...
  -3 / 2) .* (((x1x + (-1) .* x3x) .* ((x1x + (-1) .* x3x) .^ 2 + ( ...
  x1y + (-1) .* x3y) .^ 2 + (x1z + (-1) .* x3z) .^ 2) .^ (-1 / 2) +  ...
  (x2x + (-1) .* x4x) .* ((x2x + (-1) .* x4x) .^ 2 + (x2y + (-1) .*  ...
  x4y) .^ 2 + (x2z + (-1) .* x4z) .^ 2) .^ (-1 / 2)) .^ 2 + ((x1y +  ...
  (-1) .* x3y) .* ((x1x + (-1) .* x3x) .^ 2 + (x1y + (-1) .* x3y)  ...
  .^ 2 + (x1z + (-1) .* x3z) .^ 2) .^ (-1 / 2) + (x2y + (-1) .* x4y) ...
   .* ((x2x + (-1) .* x4x) .^ 2 + (x2y + (-1) .* x4y) .^ 2 + (x2z +  ...
  (-1) .* x4z) .^ 2) .^ (-1 / 2)) .^ 2 + (((x1x + (-1) .* x3x) .^ 2  ...
  + (x1y + (-1) .* x3y) .^ 2 + (x1z + (-1) .* x3z) .^ 2) .^ (-1 / 2) ...
   .* (x1z + (-1) .* x3z) + ((x2x + (-1) .* x4x) .^ 2 + (x2y + (-1)  ...
  .* x4y) .^ 2 + (x2z + (-1) .* x4z) .^ 2) .^ (-1 / 2) .* (x2z + ( ...
  -1) .* x4z)) .^ 2) .^ (-1 / 2) .* ((x1z + (-1) .* x3z) .* (x2x + ( ...
  -1) .* x4x) + (-1) .* (x1x + (-1) .* x3x) .* (x2z + (-1) .* x4z))  ...
  .* (((x1x + (-1) .* x3x) .^ 2 + (x1y + (-1) .* x3y) .^ 2 + (x1z +  ...
  (-1) .* x3z) .^ 2) .^ (-1 / 2) .* (x1z + (-1) .* x3z) + ((x2x + ( ...
  -1) .* x4x) .^ 2 + (x2y + (-1) .* x4y) .^ 2 + (x2z + (-1) .* x4z)  ...
  .^ 2) .^ (-1 / 2) .* (x2z + (-1) .* x4z)) + (-1 / 2) .* ((((-1) .* ...
   x1y + x3y) .* (x2x + (-1) .* x4x) + (x1x + (-1) .* x3x) .* (x2y + ...
   (-1) .* x4y)) .^ 2 + ((x1z + (-1) .* x3z) .* (x2x + (-1) .* x4x)  ...
  + (-1) .* (x1x + (-1) .* x3x) .* (x2z + (-1) .* x4z)) .^ 2 + ((( ...
  -1) .* x1z + x3z) .* (x2y + (-1) .* x4y) + (x1y + (-1) .* x3y) .*  ...
  (x2z + (-1) .* x4z)) .^ 2) .^ (-1 / 2) .* (((x1x + (-1) .* x3x) .* ...
   ((x1x + (-1) .* x3x) .^ 2 + (x1y + (-1) .* x3y) .^ 2 + (x1z + ( ...
  -1) .* x3z) .^ 2) .^ (-1 / 2) + (x2x + (-1) .* x4x) .* ((x2x + ( ...
  -1) .* x4x) .^ 2 + (x2y + (-1) .* x4y) .^ 2 + (x2z + (-1) .* x4z)  ...
  .^ 2) .^ (-1 / 2)) .^ 2 + ((x1y + (-1) .* x3y) .* ((x1x + (-1) .*  ...
  x3x) .^ 2 + (x1y + (-1) .* x3y) .^ 2 + (x1z + (-1) .* x3z) .^ 2)  ...
  .^ (-1 / 2) + (x2y + (-1) .* x4y) .* ((x2x + (-1) .* x4x) .^ 2 + ( ...
  x2y + (-1) .* x4y) .^ 2 + (x2z + (-1) .* x4z) .^ 2) .^ (-1 / 2))  ...
  .^ 2 + (((x1x + (-1) .* x3x) .^ 2 + (x1y + (-1) .* x3y) .^ 2 + ( ...
  x1z + (-1) .* x3z) .^ 2) .^ (-1 / 2) .* (x1z + (-1) .* x3z) + (( ...
  x2x + (-1) .* x4x) .^ 2 + (x2y + (-1) .* x4y) .^ 2 + (x2z + (-1)  ...
  .* x4z) .^ 2) .^ (-1 / 2) .* (x2z + (-1) .* x4z)) .^ 2) .^ (-3 /  ...
  2) .* ((x1z + (-1) .* x3z) .* (x2x + (-1) .* x4x) + (-1) .* (x1x + ...
   (-1) .* x3x) .* (x2z + (-1) .* x4z)) .* (2 .* (((x1x + (-1) .*  ...
  x3x) .^ 2 + (x1y + (-1) .* x3y) .^ 2 + (x1z + (-1) .* x3z) .^ 2)  ...
  .^ (-1 / 2) .* (x1z + (-1) .* x3z) + ((x2x + (-1) .* x4x) .^ 2 + ( ...
  x2y + (-1) .* x4y) .^ 2 + (x2z + (-1) .* x4z) .^ 2) .^ (-1 / 2) .* ...
   (x2z + (-1) .* x4z)) .* ((-1) .* ((x2x + (-1) .* x4x) .^ 2 + ( ...
  x2y + (-1) .* x4y) .^ 2 + (x2z + (-1) .* x4z) .^ 2) .^ (-1 / 2) +  ...
  ((x2x + (-1) .* x4x) .^ 2 + (x2y + (-1) .* x4y) .^ 2 + (x2z + (-1) ...
   .* x4z) .^ 2) .^ (-3 / 2) .* (x2z + (-1) .* x4z) .^ 2) + 2 .* ( ...
  x2x + (-1) .* x4x) .* ((x1x + (-1) .* x3x) .* ((x1x + (-1) .* x3x) ...
   .^ 2 + (x1y + (-1) .* x3y) .^ 2 + (x1z + (-1) .* x3z) .^ 2) .^ ( ...
  -1 / 2) + (x2x + (-1) .* x4x) .* ((x2x + (-1) .* x4x) .^ 2 + (x2y  ...
  + (-1) .* x4y) .^ 2 + (x2z + (-1) .* x4z) .^ 2) .^ (-1 / 2)) .* (( ...
  x2x + (-1) .* x4x) .^ 2 + (x2y + (-1) .* x4y) .^ 2 + (x2z + (-1)  ...
  .* x4z) .^ 2) .^ (-3 / 2) .* (x2z + (-1) .* x4z) + 2 .* (x2y + ( ...
  -1) .* x4y) .* ((x1y + (-1) .* x3y) .* ((x1x + (-1) .* x3x) .^ 2 + ...
   (x1y + (-1) .* x3y) .^ 2 + (x1z + (-1) .* x3z) .^ 2) .^ (-1 / 2)  ...
  + (x2y + (-1) .* x4y) .* ((x2x + (-1) .* x4x) .^ 2 + (x2y + (-1)  ...
  .* x4y) .^ 2 + (x2z + (-1) .* x4z) .^ 2) .^ (-1 / 2)) .* ((x2x + ( ...
  -1) .* x4x) .^ 2 + (x2y + (-1) .* x4y) .^ 2 + (x2z + (-1) .* x4z)  ...
  .^ 2) .^ (-3 / 2) .* (x2z + (-1) .* x4z)) .* (((x1x + (-1) .* x3x) ...
   .^ 2 + (x1y + (-1) .* x3y) .^ 2 + (x1z + (-1) .* x3z) .^ 2) .^ ( ...
  -1 / 2) .* (x1z + (-1) .* x3z) + ((x2x + (-1) .* x4x) .^ 2 + (x2y  ...
  + (-1) .* x4y) .^ 2 + (x2z + (-1) .* x4z) .^ 2) .^ (-1 / 2) .* ( ...
  x2z + (-1) .* x4z)) + ((((-1) .* x1y + x3y) .* (x2x + (-1) .* x4x) ...
   + (x1x + (-1) .* x3x) .* (x2y + (-1) .* x4y)) .^ 2 + ((x1z + (-1) ...
   .* x3z) .* (x2x + (-1) .* x4x) + (-1) .* (x1x + (-1) .* x3x) .* ( ...
  x2z + (-1) .* x4z)) .^ 2 + (((-1) .* x1z + x3z) .* (x2y + (-1) .*  ...
  x4y) + (x1y + (-1) .* x3y) .* (x2z + (-1) .* x4z)) .^ 2) .^ (-1 /  ...
  2) .* (((x1x + (-1) .* x3x) .* ((x1x + (-1) .* x3x) .^ 2 + (x1y +  ...
  (-1) .* x3y) .^ 2 + (x1z + (-1) .* x3z) .^ 2) .^ (-1 / 2) + (x2x + ...
   (-1) .* x4x) .* ((x2x + (-1) .* x4x) .^ 2 + (x2y + (-1) .* x4y)  ...
  .^ 2 + (x2z + (-1) .* x4z) .^ 2) .^ (-1 / 2)) .^ 2 + ((x1y + (-1)  ...
  .* x3y) .* ((x1x + (-1) .* x3x) .^ 2 + (x1y + (-1) .* x3y) .^ 2 +  ...
  (x1z + (-1) .* x3z) .^ 2) .^ (-1 / 2) + (x2y + (-1) .* x4y) .* (( ...
  x2x + (-1) .* x4x) .^ 2 + (x2y + (-1) .* x4y) .^ 2 + (x2z + (-1)  ...
  .* x4z) .^ 2) .^ (-1 / 2)) .^ 2 + (((x1x + (-1) .* x3x) .^ 2 + ( ...
  x1y + (-1) .* x3y) .^ 2 + (x1z + (-1) .* x3z) .^ 2) .^ (-1 / 2) .* ...
   (x1z + (-1) .* x3z) + ((x2x + (-1) .* x4x) .^ 2 + (x2y + (-1) .*  ...
  x4y) .^ 2 + (x2z + (-1) .* x4z) .^ 2) .^ (-1 / 2) .* (x2z + (-1)  ...
  .* x4z)) .^ 2) .^ (-1 / 2) .* ((x1z + (-1) .* x3z) .* (x2x + (-1)  ...
  .* x4x) + (-1) .* (x1x + (-1) .* x3x) .* (x2z + (-1) .* x4z)) .* ( ...
  (-1) .* ((x2x + (-1) .* x4x) .^ 2 + (x2y + (-1) .* x4y) .^ 2 + ( ...
  x2z + (-1) .* x4z) .^ 2) .^ (-1 / 2) + ((x2x + (-1) .* x4x) .^ 2 + ...
   (x2y + (-1) .* x4y) .^ 2 + (x2z + (-1) .* x4z) .^ 2) .^ (-3 / 2)  ...
  .* (x2z + (-1) .* x4z) .^ 2) + (-1) .* (((-1) .* x1y + x3y) .* ( ...
  x2x + (-1) .* x4x) + (x1x + (-1) .* x3x) .* (x2y + (-1) .* x4y))  ...
  .* (x2y + (-1) .* x4y) .* ((((-1) .* x1y + x3y) .* (x2x + (-1) .*  ...
  x4x) + (x1x + (-1) .* x3x) .* (x2y + (-1) .* x4y)) .^ 2 + ((x1z +  ...
  (-1) .* x3z) .* (x2x + (-1) .* x4x) + (-1) .* (x1x + (-1) .* x3x)  ...
  .* (x2z + (-1) .* x4z)) .^ 2 + (((-1) .* x1z + x3z) .* (x2y + (-1) ...
   .* x4y) + (x1y + (-1) .* x3y) .* (x2z + (-1) .* x4z)) .^ 2) .^ ( ...
  -1 / 2) .* (((x1x + (-1) .* x3x) .* ((x1x + (-1) .* x3x) .^ 2 + ( ...
  x1y + (-1) .* x3y) .^ 2 + (x1z + (-1) .* x3z) .^ 2) .^ (-1 / 2) +  ...
  (x2x + (-1) .* x4x) .* ((x2x + (-1) .* x4x) .^ 2 + (x2y + (-1) .*  ...
  x4y) .^ 2 + (x2z + (-1) .* x4z) .^ 2) .^ (-1 / 2)) .^ 2 + ((x1y +  ...
  (-1) .* x3y) .* ((x1x + (-1) .* x3x) .^ 2 + (x1y + (-1) .* x3y)  ...
  .^ 2 + (x1z + (-1) .* x3z) .^ 2) .^ (-1 / 2) + (x2y + (-1) .* x4y) ...
   .* ((x2x + (-1) .* x4x) .^ 2 + (x2y + (-1) .* x4y) .^ 2 + (x2z +  ...
  (-1) .* x4z) .^ 2) .^ (-1 / 2)) .^ 2 + (((x1x + (-1) .* x3x) .^ 2  ...
  + (x1y + (-1) .* x3y) .^ 2 + (x1z + (-1) .* x3z) .^ 2) .^ (-1 / 2) ...
   .* (x1z + (-1) .* x3z) + ((x2x + (-1) .* x4x) .^ 2 + (x2y + (-1)  ...
  .* x4y) .^ 2 + (x2z + (-1) .* x4z) .^ 2) .^ (-1 / 2) .* (x2z + ( ...
  -1) .* x4z)) .^ 2) .^ (-1 / 2) .* ((x2x + (-1) .* x4x) .^ 2 + ( ...
  x2y + (-1) .* x4y) .^ 2 + (x2z + (-1) .* x4z) .^ 2) .^ (-3 / 2) .* ...
   (x2z + (-1) .* x4z);((-1) .* (x1x + (-1) .* x3x) .^ 2 .* ((x1x +  ...
  (-1) .* x3x) .^ 2 + (x1y + (-1) .* x3y) .^ 2 + (x1z + (-1) .* x3z) ...
   .^ 2) .^ (-3 / 2) + ((x1x + (-1) .* x3x) .^ 2 + (x1y + (-1) .*  ...
  x3y) .^ 2 + (x1z + (-1) .* x3z) .^ 2) .^ (-1 / 2)) .* (((-1) .*  ...
  x1y + x3y) .* (x2x + (-1) .* x4x) + (x1x + (-1) .* x3x) .* (x2y +  ...
  (-1) .* x4y)) .* ((((-1) .* x1y + x3y) .* (x2x + (-1) .* x4x) + ( ...
  x1x + (-1) .* x3x) .* (x2y + (-1) .* x4y)) .^ 2 + ((x1z + (-1) .*  ...
  x3z) .* (x2x + (-1) .* x4x) + (-1) .* (x1x + (-1) .* x3x) .* (x2z  ...
  + (-1) .* x4z)) .^ 2 + (((-1) .* x1z + x3z) .* (x2y + (-1) .* x4y) ...
   + (x1y + (-1) .* x3y) .* (x2z + (-1) .* x4z)) .^ 2) .^ (-1 / 2)  ...
  .* (((x1x + (-1) .* x3x) .* ((x1x + (-1) .* x3x) .^ 2 + (x1y + ( ...
  -1) .* x3y) .^ 2 + (x1z + (-1) .* x3z) .^ 2) .^ (-1 / 2) + (x2x +  ...
  (-1) .* x4x) .* ((x2x + (-1) .* x4x) .^ 2 + (x2y + (-1) .* x4y)  ...
  .^ 2 + (x2z + (-1) .* x4z) .^ 2) .^ (-1 / 2)) .^ 2 + ((x1y + (-1)  ...
  .* x3y) .* ((x1x + (-1) .* x3x) .^ 2 + (x1y + (-1) .* x3y) .^ 2 +  ...
  (x1z + (-1) .* x3z) .^ 2) .^ (-1 / 2) + (x2y + (-1) .* x4y) .* (( ...
  x2x + (-1) .* x4x) .^ 2 + (x2y + (-1) .* x4y) .^ 2 + (x2z + (-1)  ...
  .* x4z) .^ 2) .^ (-1 / 2)) .^ 2 + (((x1x + (-1) .* x3x) .^ 2 + ( ...
  x1y + (-1) .* x3y) .^ 2 + (x1z + (-1) .* x3z) .^ 2) .^ (-1 / 2) .* ...
   (x1z + (-1) .* x3z) + ((x2x + (-1) .* x4x) .^ 2 + (x2y + (-1) .*  ...
  x4y) .^ 2 + (x2z + (-1) .* x4z) .^ 2) .^ (-1 / 2) .* (x2z + (-1)  ...
  .* x4z)) .^ 2) .^ (-1 / 2) + (-1 / 2) .* (((-1) .* x1y + x3y) .* ( ...
  x2x + (-1) .* x4x) + (x1x + (-1) .* x3x) .* (x2y + (-1) .* x4y))  ...
  .* ((((-1) .* x1y + x3y) .* (x2x + (-1) .* x4x) + (x1x + (-1) .*  ...
  x3x) .* (x2y + (-1) .* x4y)) .^ 2 + ((x1z + (-1) .* x3z) .* (x2x + ...
   (-1) .* x4x) + (-1) .* (x1x + (-1) .* x3x) .* (x2z + (-1) .* x4z) ...
  ) .^ 2 + (((-1) .* x1z + x3z) .* (x2y + (-1) .* x4y) + (x1y + (-1) ...
   .* x3y) .* (x2z + (-1) .* x4z)) .^ 2) .^ (-1 / 2) .* (2 .* ((-1)  ...
  .* (x1x + (-1) .* x3x) .^ 2 .* ((x1x + (-1) .* x3x) .^ 2 + (x1y +  ...
  (-1) .* x3y) .^ 2 + (x1z + (-1) .* x3z) .^ 2) .^ (-3 / 2) + ((x1x  ...
  + (-1) .* x3x) .^ 2 + (x1y + (-1) .* x3y) .^ 2 + (x1z + (-1) .*  ...
  x3z) .^ 2) .^ (-1 / 2)) .* ((x1x + (-1) .* x3x) .* ((x1x + (-1) .* ...
   x3x) .^ 2 + (x1y + (-1) .* x3y) .^ 2 + (x1z + (-1) .* x3z) .^ 2)  ...
  .^ (-1 / 2) + (x2x + (-1) .* x4x) .* ((x2x + (-1) .* x4x) .^ 2 + ( ...
  x2y + (-1) .* x4y) .^ 2 + (x2z + (-1) .* x4z) .^ 2) .^ (-1 / 2)) + ...
   (-2) .* (x1x + (-1) .* x3x) .* (x1y + (-1) .* x3y) .* ((x1x + ( ...
  -1) .* x3x) .^ 2 + (x1y + (-1) .* x3y) .^ 2 + (x1z + (-1) .* x3z)  ...
  .^ 2) .^ (-3 / 2) .* ((x1y + (-1) .* x3y) .* ((x1x + (-1) .* x3x)  ...
  .^ 2 + (x1y + (-1) .* x3y) .^ 2 + (x1z + (-1) .* x3z) .^ 2) .^ ( ...
  -1 / 2) + (x2y + (-1) .* x4y) .* ((x2x + (-1) .* x4x) .^ 2 + (x2y  ...
  + (-1) .* x4y) .^ 2 + (x2z + (-1) .* x4z) .^ 2) .^ (-1 / 2)) + ( ...
  -2) .* (x1x + (-1) .* x3x) .* ((x1x + (-1) .* x3x) .^ 2 + (x1y + ( ...
  -1) .* x3y) .^ 2 + (x1z + (-1) .* x3z) .^ 2) .^ (-3 / 2) .* (x1z + ...
   (-1) .* x3z) .* (((x1x + (-1) .* x3x) .^ 2 + (x1y + (-1) .* x3y)  ...
  .^ 2 + (x1z + (-1) .* x3z) .^ 2) .^ (-1 / 2) .* (x1z + (-1) .*  ...
  x3z) + ((x2x + (-1) .* x4x) .^ 2 + (x2y + (-1) .* x4y) .^ 2 + ( ...
  x2z + (-1) .* x4z) .^ 2) .^ (-1 / 2) .* (x2z + (-1) .* x4z))) .* ( ...
  ((x1x + (-1) .* x3x) .* ((x1x + (-1) .* x3x) .^ 2 + (x1y + (-1) .* ...
   x3y) .^ 2 + (x1z + (-1) .* x3z) .^ 2) .^ (-1 / 2) + (x2x + (-1)  ...
  .* x4x) .* ((x2x + (-1) .* x4x) .^ 2 + (x2y + (-1) .* x4y) .^ 2 +  ...
  (x2z + (-1) .* x4z) .^ 2) .^ (-1 / 2)) .^ 2 + ((x1y + (-1) .* x3y) ...
   .* ((x1x + (-1) .* x3x) .^ 2 + (x1y + (-1) .* x3y) .^ 2 + (x1z +  ...
  (-1) .* x3z) .^ 2) .^ (-1 / 2) + (x2y + (-1) .* x4y) .* ((x2x + ( ...
  -1) .* x4x) .^ 2 + (x2y + (-1) .* x4y) .^ 2 + (x2z + (-1) .* x4z)  ...
  .^ 2) .^ (-1 / 2)) .^ 2 + (((x1x + (-1) .* x3x) .^ 2 + (x1y + (-1) ...
   .* x3y) .^ 2 + (x1z + (-1) .* x3z) .^ 2) .^ (-1 / 2) .* (x1z + ( ...
  -1) .* x3z) + ((x2x + (-1) .* x4x) .^ 2 + (x2y + (-1) .* x4y) .^  ...
  2 + (x2z + (-1) .* x4z) .^ 2) .^ (-1 / 2) .* (x2z + (-1) .* x4z))  ...
  .^ 2) .^ (-3 / 2) .* ((x1x + (-1) .* x3x) .* ((x1x + (-1) .* x3x)  ...
  .^ 2 + (x1y + (-1) .* x3y) .^ 2 + (x1z + (-1) .* x3z) .^ 2) .^ ( ...
  -1 / 2) + (x2x + (-1) .* x4x) .* ((x2x + (-1) .* x4x) .^ 2 + (x2y  ...
  + (-1) .* x4y) .^ 2 + (x2z + (-1) .* x4z) .^ 2) .^ (-1 / 2)) + ( ...
  x2y + (-1) .* x4y) .* ((((-1) .* x1y + x3y) .* (x2x + (-1) .* x4x) ...
   + (x1x + (-1) .* x3x) .* (x2y + (-1) .* x4y)) .^ 2 + ((x1z + (-1) ...
   .* x3z) .* (x2x + (-1) .* x4x) + (-1) .* (x1x + (-1) .* x3x) .* ( ...
  x2z + (-1) .* x4z)) .^ 2 + (((-1) .* x1z + x3z) .* (x2y + (-1) .*  ...
  x4y) + (x1y + (-1) .* x3y) .* (x2z + (-1) .* x4z)) .^ 2) .^ (-1 /  ...
  2) .* (((x1x + (-1) .* x3x) .* ((x1x + (-1) .* x3x) .^ 2 + (x1y +  ...
  (-1) .* x3y) .^ 2 + (x1z + (-1) .* x3z) .^ 2) .^ (-1 / 2) + (x2x + ...
   (-1) .* x4x) .* ((x2x + (-1) .* x4x) .^ 2 + (x2y + (-1) .* x4y)  ...
  .^ 2 + (x2z + (-1) .* x4z) .^ 2) .^ (-1 / 2)) .^ 2 + ((x1y + (-1)  ...
  .* x3y) .* ((x1x + (-1) .* x3x) .^ 2 + (x1y + (-1) .* x3y) .^ 2 +  ...
  (x1z + (-1) .* x3z) .^ 2) .^ (-1 / 2) + (x2y + (-1) .* x4y) .* (( ...
  x2x + (-1) .* x4x) .^ 2 + (x2y + (-1) .* x4y) .^ 2 + (x2z + (-1)  ...
  .* x4z) .^ 2) .^ (-1 / 2)) .^ 2 + (((x1x + (-1) .* x3x) .^ 2 + ( ...
  x1y + (-1) .* x3y) .^ 2 + (x1z + (-1) .* x3z) .^ 2) .^ (-1 / 2) .* ...
   (x1z + (-1) .* x3z) + ((x2x + (-1) .* x4x) .^ 2 + (x2y + (-1) .*  ...
  x4y) .^ 2 + (x2z + (-1) .* x4z) .^ 2) .^ (-1 / 2) .* (x2z + (-1)  ...
  .* x4z)) .^ 2) .^ (-1 / 2) .* ((x1x + (-1) .* x3x) .* ((x1x + (-1) ...
   .* x3x) .^ 2 + (x1y + (-1) .* x3y) .^ 2 + (x1z + (-1) .* x3z) .^  ...
  2) .^ (-1 / 2) + (x2x + (-1) .* x4x) .* ((x2x + (-1) .* x4x) .^ 2  ...
  + (x2y + (-1) .* x4y) .^ 2 + (x2z + (-1) .* x4z) .^ 2) .^ (-1 / 2) ...
  ) + (x1x + (-1) .* x3x) .* ((x1x + (-1) .* x3x) .^ 2 + (x1y + (-1) ...
   .* x3y) .^ 2 + (x1z + (-1) .* x3z) .^ 2) .^ (-3 / 2) .* (x1z + ( ...
  -1) .* x3z) .* ((((-1) .* x1y + x3y) .* (x2x + (-1) .* x4x) + ( ...
  x1x + (-1) .* x3x) .* (x2y + (-1) .* x4y)) .^ 2 + ((x1z + (-1) .*  ...
  x3z) .* (x2x + (-1) .* x4x) + (-1) .* (x1x + (-1) .* x3x) .* (x2z  ...
  + (-1) .* x4z)) .^ 2 + (((-1) .* x1z + x3z) .* (x2y + (-1) .* x4y) ...
   + (x1y + (-1) .* x3y) .* (x2z + (-1) .* x4z)) .^ 2) .^ (-1 / 2)  ...
  .* (((x1x + (-1) .* x3x) .* ((x1x + (-1) .* x3x) .^ 2 + (x1y + ( ...
  -1) .* x3y) .^ 2 + (x1z + (-1) .* x3z) .^ 2) .^ (-1 / 2) + (x2x +  ...
  (-1) .* x4x) .* ((x2x + (-1) .* x4x) .^ 2 + (x2y + (-1) .* x4y)  ...
  .^ 2 + (x2z + (-1) .* x4z) .^ 2) .^ (-1 / 2)) .^ 2 + ((x1y + (-1)  ...
  .* x3y) .* ((x1x + (-1) .* x3x) .^ 2 + (x1y + (-1) .* x3y) .^ 2 +  ...
  (x1z + (-1) .* x3z) .^ 2) .^ (-1 / 2) + (x2y + (-1) .* x4y) .* (( ...
  x2x + (-1) .* x4x) .^ 2 + (x2y + (-1) .* x4y) .^ 2 + (x2z + (-1)  ...
  .* x4z) .^ 2) .^ (-1 / 2)) .^ 2 + (((x1x + (-1) .* x3x) .^ 2 + ( ...
  x1y + (-1) .* x3y) .^ 2 + (x1z + (-1) .* x3z) .^ 2) .^ (-1 / 2) .* ...
   (x1z + (-1) .* x3z) + ((x2x + (-1) .* x4x) .^ 2 + (x2y + (-1) .*  ...
  x4y) .^ 2 + (x2z + (-1) .* x4z) .^ 2) .^ (-1 / 2) .* (x2z + (-1)  ...
  .* x4z)) .^ 2) .^ (-1 / 2) .* (((-1) .* x1z + x3z) .* (x2y + (-1)  ...
  .* x4y) + (x1y + (-1) .* x3y) .* (x2z + (-1) .* x4z)) + (1 / 2) .* ...
   ((((-1) .* x1y + x3y) .* (x2x + (-1) .* x4x) + (x1x + (-1) .*  ...
  x3x) .* (x2y + (-1) .* x4y)) .^ 2 + ((x1z + (-1) .* x3z) .* (x2x + ...
   (-1) .* x4x) + (-1) .* (x1x + (-1) .* x3x) .* (x2z + (-1) .* x4z) ...
  ) .^ 2 + (((-1) .* x1z + x3z) .* (x2y + (-1) .* x4y) + (x1y + (-1) ...
   .* x3y) .* (x2z + (-1) .* x4z)) .^ 2) .^ (-1 / 2) .* (2 .* ((-1)  ...
  .* (x1x + (-1) .* x3x) .^ 2 .* ((x1x + (-1) .* x3x) .^ 2 + (x1y +  ...
  (-1) .* x3y) .^ 2 + (x1z + (-1) .* x3z) .^ 2) .^ (-3 / 2) + ((x1x  ...
  + (-1) .* x3x) .^ 2 + (x1y + (-1) .* x3y) .^ 2 + (x1z + (-1) .*  ...
  x3z) .^ 2) .^ (-1 / 2)) .* ((x1x + (-1) .* x3x) .* ((x1x + (-1) .* ...
   x3x) .^ 2 + (x1y + (-1) .* x3y) .^ 2 + (x1z + (-1) .* x3z) .^ 2)  ...
  .^ (-1 / 2) + (x2x + (-1) .* x4x) .* ((x2x + (-1) .* x4x) .^ 2 + ( ...
  x2y + (-1) .* x4y) .^ 2 + (x2z + (-1) .* x4z) .^ 2) .^ (-1 / 2)) + ...
   (-2) .* (x1x + (-1) .* x3x) .* (x1y + (-1) .* x3y) .* ((x1x + ( ...
  -1) .* x3x) .^ 2 + (x1y + (-1) .* x3y) .^ 2 + (x1z + (-1) .* x3z)  ...
  .^ 2) .^ (-3 / 2) .* ((x1y + (-1) .* x3y) .* ((x1x + (-1) .* x3x)  ...
  .^ 2 + (x1y + (-1) .* x3y) .^ 2 + (x1z + (-1) .* x3z) .^ 2) .^ ( ...
  -1 / 2) + (x2y + (-1) .* x4y) .* ((x2x + (-1) .* x4x) .^ 2 + (x2y  ...
  + (-1) .* x4y) .^ 2 + (x2z + (-1) .* x4z) .^ 2) .^ (-1 / 2)) + ( ...
  -2) .* (x1x + (-1) .* x3x) .* ((x1x + (-1) .* x3x) .^ 2 + (x1y + ( ...
  -1) .* x3y) .^ 2 + (x1z + (-1) .* x3z) .^ 2) .^ (-3 / 2) .* (x1z + ...
   (-1) .* x3z) .* (((x1x + (-1) .* x3x) .^ 2 + (x1y + (-1) .* x3y)  ...
  .^ 2 + (x1z + (-1) .* x3z) .^ 2) .^ (-1 / 2) .* (x1z + (-1) .*  ...
  x3z) + ((x2x + (-1) .* x4x) .^ 2 + (x2y + (-1) .* x4y) .^ 2 + ( ...
  x2z + (-1) .* x4z) .^ 2) .^ (-1 / 2) .* (x2z + (-1) .* x4z))) .* ( ...
  ((x1x + (-1) .* x3x) .* ((x1x + (-1) .* x3x) .^ 2 + (x1y + (-1) .* ...
   x3y) .^ 2 + (x1z + (-1) .* x3z) .^ 2) .^ (-1 / 2) + (x2x + (-1)  ...
  .* x4x) .* ((x2x + (-1) .* x4x) .^ 2 + (x2y + (-1) .* x4y) .^ 2 +  ...
  (x2z + (-1) .* x4z) .^ 2) .^ (-1 / 2)) .^ 2 + ((x1y + (-1) .* x3y) ...
   .* ((x1x + (-1) .* x3x) .^ 2 + (x1y + (-1) .* x3y) .^ 2 + (x1z +  ...
  (-1) .* x3z) .^ 2) .^ (-1 / 2) + (x2y + (-1) .* x4y) .* ((x2x + ( ...
  -1) .* x4x) .^ 2 + (x2y + (-1) .* x4y) .^ 2 + (x2z + (-1) .* x4z)  ...
  .^ 2) .^ (-1 / 2)) .^ 2 + (((x1x + (-1) .* x3x) .^ 2 + (x1y + (-1) ...
   .* x3y) .^ 2 + (x1z + (-1) .* x3z) .^ 2) .^ (-1 / 2) .* (x1z + ( ...
  -1) .* x3z) + ((x2x + (-1) .* x4x) .^ 2 + (x2y + (-1) .* x4y) .^  ...
  2 + (x2z + (-1) .* x4z) .^ 2) .^ (-1 / 2) .* (x2z + (-1) .* x4z))  ...
  .^ 2) .^ (-3 / 2) .* (((-1) .* x1z + x3z) .* (x2y + (-1) .* x4y) + ...
   (x1y + (-1) .* x3y) .* (x2z + (-1) .* x4z)) .* (((x1x + (-1) .*  ...
  x3x) .^ 2 + (x1y + (-1) .* x3y) .^ 2 + (x1z + (-1) .* x3z) .^ 2)  ...
  .^ (-1 / 2) .* (x1z + (-1) .* x3z) + ((x2x + (-1) .* x4x) .^ 2 + ( ...
  x2y + (-1) .* x4y) .^ 2 + (x2z + (-1) .* x4z) .^ 2) .^ (-1 / 2) .* ...
   (x2z + (-1) .* x4z)) + (-1 / 2) .* (((-1) .* x1y + x3y) .* (x2x + ...
   (-1) .* x4x) + (x1x + (-1) .* x3x) .* (x2y + (-1) .* x4y)) .* ((( ...
  (-1) .* x1y + x3y) .* (x2x + (-1) .* x4x) + (x1x + (-1) .* x3x) .* ...
   (x2y + (-1) .* x4y)) .^ 2 + ((x1z + (-1) .* x3z) .* (x2x + (-1)  ...
  .* x4x) + (-1) .* (x1x + (-1) .* x3x) .* (x2z + (-1) .* x4z)) .^  ...
  2 + (((-1) .* x1z + x3z) .* (x2y + (-1) .* x4y) + (x1y + (-1) .*  ...
  x3y) .* (x2z + (-1) .* x4z)) .^ 2) .^ (-3 / 2) .* (((x1x + (-1) .* ...
   x3x) .* ((x1x + (-1) .* x3x) .^ 2 + (x1y + (-1) .* x3y) .^ 2 + ( ...
  x1z + (-1) .* x3z) .^ 2) .^ (-1 / 2) + (x2x + (-1) .* x4x) .* (( ...
  x2x + (-1) .* x4x) .^ 2 + (x2y + (-1) .* x4y) .^ 2 + (x2z + (-1)  ...
  .* x4z) .^ 2) .^ (-1 / 2)) .^ 2 + ((x1y + (-1) .* x3y) .* ((x1x +  ...
  (-1) .* x3x) .^ 2 + (x1y + (-1) .* x3y) .^ 2 + (x1z + (-1) .* x3z) ...
   .^ 2) .^ (-1 / 2) + (x2y + (-1) .* x4y) .* ((x2x + (-1) .* x4x)  ...
  .^ 2 + (x2y + (-1) .* x4y) .^ 2 + (x2z + (-1) .* x4z) .^ 2) .^ ( ...
  -1 / 2)) .^ 2 + (((x1x + (-1) .* x3x) .^ 2 + (x1y + (-1) .* x3y)  ...
  .^ 2 + (x1z + (-1) .* x3z) .^ 2) .^ (-1 / 2) .* (x1z + (-1) .*  ...
  x3z) + ((x2x + (-1) .* x4x) .^ 2 + (x2y + (-1) .* x4y) .^ 2 + ( ...
  x2z + (-1) .* x4z) .^ 2) .^ (-1 / 2) .* (x2z + (-1) .* x4z)) .^ 2) ...
   .^ (-1 / 2) .* ((x1x + (-1) .* x3x) .* ((x1x + (-1) .* x3x) .^ 2  ...
  + (x1y + (-1) .* x3y) .^ 2 + (x1z + (-1) .* x3z) .^ 2) .^ (-1 / 2) ...
   + (x2x + (-1) .* x4x) .* ((x2x + (-1) .* x4x) .^ 2 + (x2y + (-1)  ...
  .* x4y) .^ 2 + (x2z + (-1) .* x4z) .^ 2) .^ (-1 / 2)) .* (2 .* ((( ...
  -1) .* x1y + x3y) .* (x2x + (-1) .* x4x) + (x1x + (-1) .* x3x) .*  ...
  (x2y + (-1) .* x4y)) .* (x2y + (-1) .* x4y) + 2 .* ((x1z + (-1) .* ...
   x3z) .* (x2x + (-1) .* x4x) + (-1) .* (x1x + (-1) .* x3x) .* ( ...
  x2z + (-1) .* x4z)) .* ((-1) .* x2z + x4z)) + (1 / 2) .* ((((-1)  ...
  .* x1y + x3y) .* (x2x + (-1) .* x4x) + (x1x + (-1) .* x3x) .* ( ...
  x2y + (-1) .* x4y)) .^ 2 + ((x1z + (-1) .* x3z) .* (x2x + (-1) .*  ...
  x4x) + (-1) .* (x1x + (-1) .* x3x) .* (x2z + (-1) .* x4z)) .^ 2 +  ...
  (((-1) .* x1z + x3z) .* (x2y + (-1) .* x4y) + (x1y + (-1) .* x3y)  ...
  .* (x2z + (-1) .* x4z)) .^ 2) .^ (-3 / 2) .* (((x1x + (-1) .* x3x) ...
   .* ((x1x + (-1) .* x3x) .^ 2 + (x1y + (-1) .* x3y) .^ 2 + (x1z +  ...
  (-1) .* x3z) .^ 2) .^ (-1 / 2) + (x2x + (-1) .* x4x) .* ((x2x + ( ...
  -1) .* x4x) .^ 2 + (x2y + (-1) .* x4y) .^ 2 + (x2z + (-1) .* x4z)  ...
  .^ 2) .^ (-1 / 2)) .^ 2 + ((x1y + (-1) .* x3y) .* ((x1x + (-1) .*  ...
  x3x) .^ 2 + (x1y + (-1) .* x3y) .^ 2 + (x1z + (-1) .* x3z) .^ 2)  ...
  .^ (-1 / 2) + (x2y + (-1) .* x4y) .* ((x2x + (-1) .* x4x) .^ 2 + ( ...
  x2y + (-1) .* x4y) .^ 2 + (x2z + (-1) .* x4z) .^ 2) .^ (-1 / 2))  ...
  .^ 2 + (((x1x + (-1) .* x3x) .^ 2 + (x1y + (-1) .* x3y) .^ 2 + ( ...
  x1z + (-1) .* x3z) .^ 2) .^ (-1 / 2) .* (x1z + (-1) .* x3z) + (( ...
  x2x + (-1) .* x4x) .^ 2 + (x2y + (-1) .* x4y) .^ 2 + (x2z + (-1)  ...
  .* x4z) .^ 2) .^ (-1 / 2) .* (x2z + (-1) .* x4z)) .^ 2) .^ (-1 /  ...
  2) .* (((-1) .* x1z + x3z) .* (x2y + (-1) .* x4y) + (x1y + (-1) .* ...
   x3y) .* (x2z + (-1) .* x4z)) .* (((x1x + (-1) .* x3x) .^ 2 + ( ...
  x1y + (-1) .* x3y) .^ 2 + (x1z + (-1) .* x3z) .^ 2) .^ (-1 / 2) .* ...
   (x1z + (-1) .* x3z) + ((x2x + (-1) .* x4x) .^ 2 + (x2y + (-1) .*  ...
  x4y) .^ 2 + (x2z + (-1) .* x4z) .^ 2) .^ (-1 / 2) .* (x2z + (-1)  ...
  .* x4z)) .* (2 .* (((-1) .* x1y + x3y) .* (x2x + (-1) .* x4x) + ( ...
  x1x + (-1) .* x3x) .* (x2y + (-1) .* x4y)) .* (x2y + (-1) .* x4y)  ...
  + 2 .* ((x1z + (-1) .* x3z) .* (x2x + (-1) .* x4x) + (-1) .* (x1x  ...
  + (-1) .* x3x) .* (x2z + (-1) .* x4z)) .* ((-1) .* x2z + x4z)),( ...
  -1) .* (x1x + (-1) .* x3x) .* (x1y + (-1) .* x3y) .* ((x1x + (-1)  ...
  .* x3x) .^ 2 + (x1y + (-1) .* x3y) .^ 2 + (x1z + (-1) .* x3z) .^  ...
  2) .^ (-3 / 2) .* (((-1) .* x1y + x3y) .* (x2x + (-1) .* x4x) + ( ...
  x1x + (-1) .* x3x) .* (x2y + (-1) .* x4y)) .* ((((-1) .* x1y +  ...
  x3y) .* (x2x + (-1) .* x4x) + (x1x + (-1) .* x3x) .* (x2y + (-1)  ...
  .* x4y)) .^ 2 + ((x1z + (-1) .* x3z) .* (x2x + (-1) .* x4x) + (-1) ...
   .* (x1x + (-1) .* x3x) .* (x2z + (-1) .* x4z)) .^ 2 + (((-1) .*  ...
  x1z + x3z) .* (x2y + (-1) .* x4y) + (x1y + (-1) .* x3y) .* (x2z +  ...
  (-1) .* x4z)) .^ 2) .^ (-1 / 2) .* (((x1x + (-1) .* x3x) .* ((x1x  ...
  + (-1) .* x3x) .^ 2 + (x1y + (-1) .* x3y) .^ 2 + (x1z + (-1) .*  ...
  x3z) .^ 2) .^ (-1 / 2) + (x2x + (-1) .* x4x) .* ((x2x + (-1) .*  ...
  x4x) .^ 2 + (x2y + (-1) .* x4y) .^ 2 + (x2z + (-1) .* x4z) .^ 2)  ...
  .^ (-1 / 2)) .^ 2 + ((x1y + (-1) .* x3y) .* ((x1x + (-1) .* x3x)  ...
  .^ 2 + (x1y + (-1) .* x3y) .^ 2 + (x1z + (-1) .* x3z) .^ 2) .^ ( ...
  -1 / 2) + (x2y + (-1) .* x4y) .* ((x2x + (-1) .* x4x) .^ 2 + (x2y  ...
  + (-1) .* x4y) .^ 2 + (x2z + (-1) .* x4z) .^ 2) .^ (-1 / 2)) .^ 2  ...
  + (((x1x + (-1) .* x3x) .^ 2 + (x1y + (-1) .* x3y) .^ 2 + (x1z + ( ...
  -1) .* x3z) .^ 2) .^ (-1 / 2) .* (x1z + (-1) .* x3z) + ((x2x + ( ...
  -1) .* x4x) .^ 2 + (x2y + (-1) .* x4y) .^ 2 + (x2z + (-1) .* x4z)  ...
  .^ 2) .^ (-1 / 2) .* (x2z + (-1) .* x4z)) .^ 2) .^ (-1 / 2) + (-1  ...
  / 2) .* (((-1) .* x1y + x3y) .* (x2x + (-1) .* x4x) + (x1x + (-1)  ...
  .* x3x) .* (x2y + (-1) .* x4y)) .* ((((-1) .* x1y + x3y) .* (x2x + ...
   (-1) .* x4x) + (x1x + (-1) .* x3x) .* (x2y + (-1) .* x4y)) .^ 2 + ...
   ((x1z + (-1) .* x3z) .* (x2x + (-1) .* x4x) + (-1) .* (x1x + (-1) ...
   .* x3x) .* (x2z + (-1) .* x4z)) .^ 2 + (((-1) .* x1z + x3z) .* ( ...
  x2y + (-1) .* x4y) + (x1y + (-1) .* x3y) .* (x2z + (-1) .* x4z))  ...
  .^ 2) .^ (-1 / 2) .* ((-2) .* (x1x + (-1) .* x3x) .* (x1y + (-1)  ...
  .* x3y) .* ((x1x + (-1) .* x3x) .^ 2 + (x1y + (-1) .* x3y) .^ 2 +  ...
  (x1z + (-1) .* x3z) .^ 2) .^ (-3 / 2) .* ((x1x + (-1) .* x3x) .* ( ...
  (x1x + (-1) .* x3x) .^ 2 + (x1y + (-1) .* x3y) .^ 2 + (x1z + (-1)  ...
  .* x3z) .^ 2) .^ (-1 / 2) + (x2x + (-1) .* x4x) .* ((x2x + (-1) .* ...
   x4x) .^ 2 + (x2y + (-1) .* x4y) .^ 2 + (x2z + (-1) .* x4z) .^ 2)  ...
  .^ (-1 / 2)) + 2 .* ((-1) .* (x1y + (-1) .* x3y) .^ 2 .* ((x1x + ( ...
  -1) .* x3x) .^ 2 + (x1y + (-1) .* x3y) .^ 2 + (x1z + (-1) .* x3z)  ...
  .^ 2) .^ (-3 / 2) + ((x1x + (-1) .* x3x) .^ 2 + (x1y + (-1) .*  ...
  x3y) .^ 2 + (x1z + (-1) .* x3z) .^ 2) .^ (-1 / 2)) .* ((x1y + (-1) ...
   .* x3y) .* ((x1x + (-1) .* x3x) .^ 2 + (x1y + (-1) .* x3y) .^ 2 + ...
   (x1z + (-1) .* x3z) .^ 2) .^ (-1 / 2) + (x2y + (-1) .* x4y) .* (( ...
  x2x + (-1) .* x4x) .^ 2 + (x2y + (-1) .* x4y) .^ 2 + (x2z + (-1)  ...
  .* x4z) .^ 2) .^ (-1 / 2)) + (-2) .* (x1y + (-1) .* x3y) .* ((x1x  ...
  + (-1) .* x3x) .^ 2 + (x1y + (-1) .* x3y) .^ 2 + (x1z + (-1) .*  ...
  x3z) .^ 2) .^ (-3 / 2) .* (x1z + (-1) .* x3z) .* (((x1x + (-1) .*  ...
  x3x) .^ 2 + (x1y + (-1) .* x3y) .^ 2 + (x1z + (-1) .* x3z) .^ 2)  ...
  .^ (-1 / 2) .* (x1z + (-1) .* x3z) + ((x2x + (-1) .* x4x) .^ 2 + ( ...
  x2y + (-1) .* x4y) .^ 2 + (x2z + (-1) .* x4z) .^ 2) .^ (-1 / 2) .* ...
   (x2z + (-1) .* x4z))) .* (((x1x + (-1) .* x3x) .* ((x1x + (-1) .* ...
   x3x) .^ 2 + (x1y + (-1) .* x3y) .^ 2 + (x1z + (-1) .* x3z) .^ 2)  ...
  .^ (-1 / 2) + (x2x + (-1) .* x4x) .* ((x2x + (-1) .* x4x) .^ 2 + ( ...
  x2y + (-1) .* x4y) .^ 2 + (x2z + (-1) .* x4z) .^ 2) .^ (-1 / 2))  ...
  .^ 2 + ((x1y + (-1) .* x3y) .* ((x1x + (-1) .* x3x) .^ 2 + (x1y +  ...
  (-1) .* x3y) .^ 2 + (x1z + (-1) .* x3z) .^ 2) .^ (-1 / 2) + (x2y + ...
   (-1) .* x4y) .* ((x2x + (-1) .* x4x) .^ 2 + (x2y + (-1) .* x4y)  ...
  .^ 2 + (x2z + (-1) .* x4z) .^ 2) .^ (-1 / 2)) .^ 2 + (((x1x + (-1) ...
   .* x3x) .^ 2 + (x1y + (-1) .* x3y) .^ 2 + (x1z + (-1) .* x3z) .^  ...
  2) .^ (-1 / 2) .* (x1z + (-1) .* x3z) + ((x2x + (-1) .* x4x) .^ 2  ...
  + (x2y + (-1) .* x4y) .^ 2 + (x2z + (-1) .* x4z) .^ 2) .^ (-1 / 2) ...
   .* (x2z + (-1) .* x4z)) .^ 2) .^ (-3 / 2) .* ((x1x + (-1) .* x3x) ...
   .* ((x1x + (-1) .* x3x) .^ 2 + (x1y + (-1) .* x3y) .^ 2 + (x1z +  ...
  (-1) .* x3z) .^ 2) .^ (-1 / 2) + (x2x + (-1) .* x4x) .* ((x2x + ( ...
  -1) .* x4x) .^ 2 + (x2y + (-1) .* x4y) .^ 2 + (x2z + (-1) .* x4z)  ...
  .^ 2) .^ (-1 / 2)) + ((-1) .* x2x + x4x) .* ((((-1) .* x1y + x3y)  ...
  .* (x2x + (-1) .* x4x) + (x1x + (-1) .* x3x) .* (x2y + (-1) .*  ...
  x4y)) .^ 2 + ((x1z + (-1) .* x3z) .* (x2x + (-1) .* x4x) + (-1) .* ...
   (x1x + (-1) .* x3x) .* (x2z + (-1) .* x4z)) .^ 2 + (((-1) .* x1z  ...
  + x3z) .* (x2y + (-1) .* x4y) + (x1y + (-1) .* x3y) .* (x2z + (-1) ...
   .* x4z)) .^ 2) .^ (-1 / 2) .* (((x1x + (-1) .* x3x) .* ((x1x + ( ...
  -1) .* x3x) .^ 2 + (x1y + (-1) .* x3y) .^ 2 + (x1z + (-1) .* x3z)  ...
  .^ 2) .^ (-1 / 2) + (x2x + (-1) .* x4x) .* ((x2x + (-1) .* x4x)  ...
  .^ 2 + (x2y + (-1) .* x4y) .^ 2 + (x2z + (-1) .* x4z) .^ 2) .^ ( ...
  -1 / 2)) .^ 2 + ((x1y + (-1) .* x3y) .* ((x1x + (-1) .* x3x) .^ 2  ...
  + (x1y + (-1) .* x3y) .^ 2 + (x1z + (-1) .* x3z) .^ 2) .^ (-1 / 2) ...
   + (x2y + (-1) .* x4y) .* ((x2x + (-1) .* x4x) .^ 2 + (x2y + (-1)  ...
  .* x4y) .^ 2 + (x2z + (-1) .* x4z) .^ 2) .^ (-1 / 2)) .^ 2 + ((( ...
  x1x + (-1) .* x3x) .^ 2 + (x1y + (-1) .* x3y) .^ 2 + (x1z + (-1)  ...
  .* x3z) .^ 2) .^ (-1 / 2) .* (x1z + (-1) .* x3z) + ((x2x + (-1) .* ...
   x4x) .^ 2 + (x2y + (-1) .* x4y) .^ 2 + (x2z + (-1) .* x4z) .^ 2)  ...
  .^ (-1 / 2) .* (x2z + (-1) .* x4z)) .^ 2) .^ (-1 / 2) .* ((x1x + ( ...
  -1) .* x3x) .* ((x1x + (-1) .* x3x) .^ 2 + (x1y + (-1) .* x3y) .^  ...
  2 + (x1z + (-1) .* x3z) .^ 2) .^ (-1 / 2) + (x2x + (-1) .* x4x) .* ...
   ((x2x + (-1) .* x4x) .^ 2 + (x2y + (-1) .* x4y) .^ 2 + (x2z + ( ...
  -1) .* x4z) .^ 2) .^ (-1 / 2)) + (x1y + (-1) .* x3y) .* ((x1x + ( ...
  -1) .* x3x) .^ 2 + (x1y + (-1) .* x3y) .^ 2 + (x1z + (-1) .* x3z)  ...
  .^ 2) .^ (-3 / 2) .* (x1z + (-1) .* x3z) .* ((((-1) .* x1y + x3y)  ...
  .* (x2x + (-1) .* x4x) + (x1x + (-1) .* x3x) .* (x2y + (-1) .*  ...
  x4y)) .^ 2 + ((x1z + (-1) .* x3z) .* (x2x + (-1) .* x4x) + (-1) .* ...
   (x1x + (-1) .* x3x) .* (x2z + (-1) .* x4z)) .^ 2 + (((-1) .* x1z  ...
  + x3z) .* (x2y + (-1) .* x4y) + (x1y + (-1) .* x3y) .* (x2z + (-1) ...
   .* x4z)) .^ 2) .^ (-1 / 2) .* (((x1x + (-1) .* x3x) .* ((x1x + ( ...
  -1) .* x3x) .^ 2 + (x1y + (-1) .* x3y) .^ 2 + (x1z + (-1) .* x3z)  ...
  .^ 2) .^ (-1 / 2) + (x2x + (-1) .* x4x) .* ((x2x + (-1) .* x4x)  ...
  .^ 2 + (x2y + (-1) .* x4y) .^ 2 + (x2z + (-1) .* x4z) .^ 2) .^ ( ...
  -1 / 2)) .^ 2 + ((x1y + (-1) .* x3y) .* ((x1x + (-1) .* x3x) .^ 2  ...
  + (x1y + (-1) .* x3y) .^ 2 + (x1z + (-1) .* x3z) .^ 2) .^ (-1 / 2) ...
   + (x2y + (-1) .* x4y) .* ((x2x + (-1) .* x4x) .^ 2 + (x2y + (-1)  ...
  .* x4y) .^ 2 + (x2z + (-1) .* x4z) .^ 2) .^ (-1 / 2)) .^ 2 + ((( ...
  x1x + (-1) .* x3x) .^ 2 + (x1y + (-1) .* x3y) .^ 2 + (x1z + (-1)  ...
  .* x3z) .^ 2) .^ (-1 / 2) .* (x1z + (-1) .* x3z) + ((x2x + (-1) .* ...
   x4x) .^ 2 + (x2y + (-1) .* x4y) .^ 2 + (x2z + (-1) .* x4z) .^ 2)  ...
  .^ (-1 / 2) .* (x2z + (-1) .* x4z)) .^ 2) .^ (-1 / 2) .* (((-1) .* ...
   x1z + x3z) .* (x2y + (-1) .* x4y) + (x1y + (-1) .* x3y) .* (x2z + ...
   (-1) .* x4z)) + (-1 / 2) .* (((-1) .* x1y + x3y) .* (x2x + (-1)  ...
  .* x4x) + (x1x + (-1) .* x3x) .* (x2y + (-1) .* x4y)) .* ((((-1)  ...
  .* x1y + x3y) .* (x2x + (-1) .* x4x) + (x1x + (-1) .* x3x) .* ( ...
  x2y + (-1) .* x4y)) .^ 2 + ((x1z + (-1) .* x3z) .* (x2x + (-1) .*  ...
  x4x) + (-1) .* (x1x + (-1) .* x3x) .* (x2z + (-1) .* x4z)) .^ 2 +  ...
  (((-1) .* x1z + x3z) .* (x2y + (-1) .* x4y) + (x1y + (-1) .* x3y)  ...
  .* (x2z + (-1) .* x4z)) .^ 2) .^ (-3 / 2) .* (((x1x + (-1) .* x3x) ...
   .* ((x1x + (-1) .* x3x) .^ 2 + (x1y + (-1) .* x3y) .^ 2 + (x1z +  ...
  (-1) .* x3z) .^ 2) .^ (-1 / 2) + (x2x + (-1) .* x4x) .* ((x2x + ( ...
  -1) .* x4x) .^ 2 + (x2y + (-1) .* x4y) .^ 2 + (x2z + (-1) .* x4z)  ...
  .^ 2) .^ (-1 / 2)) .^ 2 + ((x1y + (-1) .* x3y) .* ((x1x + (-1) .*  ...
  x3x) .^ 2 + (x1y + (-1) .* x3y) .^ 2 + (x1z + (-1) .* x3z) .^ 2)  ...
  .^ (-1 / 2) + (x2y + (-1) .* x4y) .* ((x2x + (-1) .* x4x) .^ 2 + ( ...
  x2y + (-1) .* x4y) .^ 2 + (x2z + (-1) .* x4z) .^ 2) .^ (-1 / 2))  ...
  .^ 2 + (((x1x + (-1) .* x3x) .^ 2 + (x1y + (-1) .* x3y) .^ 2 + ( ...
  x1z + (-1) .* x3z) .^ 2) .^ (-1 / 2) .* (x1z + (-1) .* x3z) + (( ...
  x2x + (-1) .* x4x) .^ 2 + (x2y + (-1) .* x4y) .^ 2 + (x2z + (-1)  ...
  .* x4z) .^ 2) .^ (-1 / 2) .* (x2z + (-1) .* x4z)) .^ 2) .^ (-1 /  ...
  2) .* ((x1x + (-1) .* x3x) .* ((x1x + (-1) .* x3x) .^ 2 + (x1y + ( ...
  -1) .* x3y) .^ 2 + (x1z + (-1) .* x3z) .^ 2) .^ (-1 / 2) + (x2x +  ...
  (-1) .* x4x) .* ((x2x + (-1) .* x4x) .^ 2 + (x2y + (-1) .* x4y)  ...
  .^ 2 + (x2z + (-1) .* x4z) .^ 2) .^ (-1 / 2)) .* (2 .* ((-1) .*  ...
  x2x + x4x) .* (((-1) .* x1y + x3y) .* (x2x + (-1) .* x4x) + (x1x + ...
   (-1) .* x3x) .* (x2y + (-1) .* x4y)) + 2 .* (((-1) .* x1z + x3z)  ...
  .* (x2y + (-1) .* x4y) + (x1y + (-1) .* x3y) .* (x2z + (-1) .*  ...
  x4z)) .* (x2z + (-1) .* x4z)) + (1 / 2) .* ((((-1) .* x1y + x3y)  ...
  .* (x2x + (-1) .* x4x) + (x1x + (-1) .* x3x) .* (x2y + (-1) .*  ...
  x4y)) .^ 2 + ((x1z + (-1) .* x3z) .* (x2x + (-1) .* x4x) + (-1) .* ...
   (x1x + (-1) .* x3x) .* (x2z + (-1) .* x4z)) .^ 2 + (((-1) .* x1z  ...
  + x3z) .* (x2y + (-1) .* x4y) + (x1y + (-1) .* x3y) .* (x2z + (-1) ...
   .* x4z)) .^ 2) .^ (-1 / 2) .* ((-2) .* (x1x + (-1) .* x3x) .* ( ...
  x1y + (-1) .* x3y) .* ((x1x + (-1) .* x3x) .^ 2 + (x1y + (-1) .*  ...
  x3y) .^ 2 + (x1z + (-1) .* x3z) .^ 2) .^ (-3 / 2) .* ((x1x + (-1)  ...
  .* x3x) .* ((x1x + (-1) .* x3x) .^ 2 + (x1y + (-1) .* x3y) .^ 2 +  ...
  (x1z + (-1) .* x3z) .^ 2) .^ (-1 / 2) + (x2x + (-1) .* x4x) .* (( ...
  x2x + (-1) .* x4x) .^ 2 + (x2y + (-1) .* x4y) .^ 2 + (x2z + (-1)  ...
  .* x4z) .^ 2) .^ (-1 / 2)) + 2 .* ((-1) .* (x1y + (-1) .* x3y) .^  ...
  2 .* ((x1x + (-1) .* x3x) .^ 2 + (x1y + (-1) .* x3y) .^ 2 + (x1z + ...
   (-1) .* x3z) .^ 2) .^ (-3 / 2) + ((x1x + (-1) .* x3x) .^ 2 + ( ...
  x1y + (-1) .* x3y) .^ 2 + (x1z + (-1) .* x3z) .^ 2) .^ (-1 / 2))  ...
  .* ((x1y + (-1) .* x3y) .* ((x1x + (-1) .* x3x) .^ 2 + (x1y + (-1) ...
   .* x3y) .^ 2 + (x1z + (-1) .* x3z) .^ 2) .^ (-1 / 2) + (x2y + ( ...
  -1) .* x4y) .* ((x2x + (-1) .* x4x) .^ 2 + (x2y + (-1) .* x4y) .^  ...
  2 + (x2z + (-1) .* x4z) .^ 2) .^ (-1 / 2)) + (-2) .* (x1y + (-1)  ...
  .* x3y) .* ((x1x + (-1) .* x3x) .^ 2 + (x1y + (-1) .* x3y) .^ 2 +  ...
  (x1z + (-1) .* x3z) .^ 2) .^ (-3 / 2) .* (x1z + (-1) .* x3z) .* (( ...
  (x1x + (-1) .* x3x) .^ 2 + (x1y + (-1) .* x3y) .^ 2 + (x1z + (-1)  ...
  .* x3z) .^ 2) .^ (-1 / 2) .* (x1z + (-1) .* x3z) + ((x2x + (-1) .* ...
   x4x) .^ 2 + (x2y + (-1) .* x4y) .^ 2 + (x2z + (-1) .* x4z) .^ 2)  ...
  .^ (-1 / 2) .* (x2z + (-1) .* x4z))) .* (((x1x + (-1) .* x3x) .* ( ...
  (x1x + (-1) .* x3x) .^ 2 + (x1y + (-1) .* x3y) .^ 2 + (x1z + (-1)  ...
  .* x3z) .^ 2) .^ (-1 / 2) + (x2x + (-1) .* x4x) .* ((x2x + (-1) .* ...
   x4x) .^ 2 + (x2y + (-1) .* x4y) .^ 2 + (x2z + (-1) .* x4z) .^ 2)  ...
  .^ (-1 / 2)) .^ 2 + ((x1y + (-1) .* x3y) .* ((x1x + (-1) .* x3x)  ...
  .^ 2 + (x1y + (-1) .* x3y) .^ 2 + (x1z + (-1) .* x3z) .^ 2) .^ ( ...
  -1 / 2) + (x2y + (-1) .* x4y) .* ((x2x + (-1) .* x4x) .^ 2 + (x2y  ...
  + (-1) .* x4y) .^ 2 + (x2z + (-1) .* x4z) .^ 2) .^ (-1 / 2)) .^ 2  ...
  + (((x1x + (-1) .* x3x) .^ 2 + (x1y + (-1) .* x3y) .^ 2 + (x1z + ( ...
  -1) .* x3z) .^ 2) .^ (-1 / 2) .* (x1z + (-1) .* x3z) + ((x2x + ( ...
  -1) .* x4x) .^ 2 + (x2y + (-1) .* x4y) .^ 2 + (x2z + (-1) .* x4z)  ...
  .^ 2) .^ (-1 / 2) .* (x2z + (-1) .* x4z)) .^ 2) .^ (-3 / 2) .* ((( ...
  -1) .* x1z + x3z) .* (x2y + (-1) .* x4y) + (x1y + (-1) .* x3y) .*  ...
  (x2z + (-1) .* x4z)) .* (((x1x + (-1) .* x3x) .^ 2 + (x1y + (-1)  ...
  .* x3y) .^ 2 + (x1z + (-1) .* x3z) .^ 2) .^ (-1 / 2) .* (x1z + ( ...
  -1) .* x3z) + ((x2x + (-1) .* x4x) .^ 2 + (x2y + (-1) .* x4y) .^  ...
  2 + (x2z + (-1) .* x4z) .^ 2) .^ (-1 / 2) .* (x2z + (-1) .* x4z))  ...
  + (1 / 2) .* ((((-1) .* x1y + x3y) .* (x2x + (-1) .* x4x) + (x1x + ...
   (-1) .* x3x) .* (x2y + (-1) .* x4y)) .^ 2 + ((x1z + (-1) .* x3z)  ...
  .* (x2x + (-1) .* x4x) + (-1) .* (x1x + (-1) .* x3x) .* (x2z + ( ...
  -1) .* x4z)) .^ 2 + (((-1) .* x1z + x3z) .* (x2y + (-1) .* x4y) +  ...
  (x1y + (-1) .* x3y) .* (x2z + (-1) .* x4z)) .^ 2) .^ (-3 / 2) .* ( ...
  ((x1x + (-1) .* x3x) .* ((x1x + (-1) .* x3x) .^ 2 + (x1y + (-1) .* ...
   x3y) .^ 2 + (x1z + (-1) .* x3z) .^ 2) .^ (-1 / 2) + (x2x + (-1)  ...
  .* x4x) .* ((x2x + (-1) .* x4x) .^ 2 + (x2y + (-1) .* x4y) .^ 2 +  ...
  (x2z + (-1) .* x4z) .^ 2) .^ (-1 / 2)) .^ 2 + ((x1y + (-1) .* x3y) ...
   .* ((x1x + (-1) .* x3x) .^ 2 + (x1y + (-1) .* x3y) .^ 2 + (x1z +  ...
  (-1) .* x3z) .^ 2) .^ (-1 / 2) + (x2y + (-1) .* x4y) .* ((x2x + ( ...
  -1) .* x4x) .^ 2 + (x2y + (-1) .* x4y) .^ 2 + (x2z + (-1) .* x4z)  ...
  .^ 2) .^ (-1 / 2)) .^ 2 + (((x1x + (-1) .* x3x) .^ 2 + (x1y + (-1) ...
   .* x3y) .^ 2 + (x1z + (-1) .* x3z) .^ 2) .^ (-1 / 2) .* (x1z + ( ...
  -1) .* x3z) + ((x2x + (-1) .* x4x) .^ 2 + (x2y + (-1) .* x4y) .^  ...
  2 + (x2z + (-1) .* x4z) .^ 2) .^ (-1 / 2) .* (x2z + (-1) .* x4z))  ...
  .^ 2) .^ (-1 / 2) .* (((-1) .* x1z + x3z) .* (x2y + (-1) .* x4y) + ...
   (x1y + (-1) .* x3y) .* (x2z + (-1) .* x4z)) .* (2 .* ((-1) .*  ...
  x2x + x4x) .* (((-1) .* x1y + x3y) .* (x2x + (-1) .* x4x) + (x1x + ...
   (-1) .* x3x) .* (x2y + (-1) .* x4y)) + 2 .* (((-1) .* x1z + x3z)  ...
  .* (x2y + (-1) .* x4y) + (x1y + (-1) .* x3y) .* (x2z + (-1) .*  ...
  x4z)) .* (x2z + (-1) .* x4z)) .* (((x1x + (-1) .* x3x) .^ 2 + ( ...
  x1y + (-1) .* x3y) .^ 2 + (x1z + (-1) .* x3z) .^ 2) .^ (-1 / 2) .* ...
   (x1z + (-1) .* x3z) + ((x2x + (-1) .* x4x) .^ 2 + (x2y + (-1) .*  ...
  x4y) .^ 2 + (x2z + (-1) .* x4z) .^ 2) .^ (-1 / 2) .* (x2z + (-1)  ...
  .* x4z)) + (-1) .* ((((-1) .* x1y + x3y) .* (x2x + (-1) .* x4x) +  ...
  (x1x + (-1) .* x3x) .* (x2y + (-1) .* x4y)) .^ 2 + ((x1z + (-1) .* ...
   x3z) .* (x2x + (-1) .* x4x) + (-1) .* (x1x + (-1) .* x3x) .* ( ...
  x2z + (-1) .* x4z)) .^ 2 + (((-1) .* x1z + x3z) .* (x2y + (-1) .*  ...
  x4y) + (x1y + (-1) .* x3y) .* (x2z + (-1) .* x4z)) .^ 2) .^ (-1 /  ...
  2) .* (((x1x + (-1) .* x3x) .* ((x1x + (-1) .* x3x) .^ 2 + (x1y +  ...
  (-1) .* x3y) .^ 2 + (x1z + (-1) .* x3z) .^ 2) .^ (-1 / 2) + (x2x + ...
   (-1) .* x4x) .* ((x2x + (-1) .* x4x) .^ 2 + (x2y + (-1) .* x4y)  ...
  .^ 2 + (x2z + (-1) .* x4z) .^ 2) .^ (-1 / 2)) .^ 2 + ((x1y + (-1)  ...
  .* x3y) .* ((x1x + (-1) .* x3x) .^ 2 + (x1y + (-1) .* x3y) .^ 2 +  ...
  (x1z + (-1) .* x3z) .^ 2) .^ (-1 / 2) + (x2y + (-1) .* x4y) .* (( ...
  x2x + (-1) .* x4x) .^ 2 + (x2y + (-1) .* x4y) .^ 2 + (x2z + (-1)  ...
  .* x4z) .^ 2) .^ (-1 / 2)) .^ 2 + (((x1x + (-1) .* x3x) .^ 2 + ( ...
  x1y + (-1) .* x3y) .^ 2 + (x1z + (-1) .* x3z) .^ 2) .^ (-1 / 2) .* ...
   (x1z + (-1) .* x3z) + ((x2x + (-1) .* x4x) .^ 2 + (x2y + (-1) .*  ...
  x4y) .^ 2 + (x2z + (-1) .* x4z) .^ 2) .^ (-1 / 2) .* (x2z + (-1)  ...
  .* x4z)) .^ 2) .^ (-1 / 2) .* (((x1x + (-1) .* x3x) .^ 2 + (x1y +  ...
  (-1) .* x3y) .^ 2 + (x1z + (-1) .* x3z) .^ 2) .^ (-1 / 2) .* (x1z  ...
  + (-1) .* x3z) + ((x2x + (-1) .* x4x) .^ 2 + (x2y + (-1) .* x4y)  ...
  .^ 2 + (x2z + (-1) .* x4z) .^ 2) .^ (-1 / 2) .* (x2z + (-1) .*  ...
  x4z)) .* (x2z + (-1) .* x4z),(-1) .* (x1x + (-1) .* x3x) .* ((x1x  ...
  + (-1) .* x3x) .^ 2 + (x1y + (-1) .* x3y) .^ 2 + (x1z + (-1) .*  ...
  x3z) .^ 2) .^ (-3 / 2) .* (x1z + (-1) .* x3z) .* (((-1) .* x1y +  ...
  x3y) .* (x2x + (-1) .* x4x) + (x1x + (-1) .* x3x) .* (x2y + (-1)  ...
  .* x4y)) .* ((((-1) .* x1y + x3y) .* (x2x + (-1) .* x4x) + (x1x +  ...
  (-1) .* x3x) .* (x2y + (-1) .* x4y)) .^ 2 + ((x1z + (-1) .* x3z)  ...
  .* (x2x + (-1) .* x4x) + (-1) .* (x1x + (-1) .* x3x) .* (x2z + ( ...
  -1) .* x4z)) .^ 2 + (((-1) .* x1z + x3z) .* (x2y + (-1) .* x4y) +  ...
  (x1y + (-1) .* x3y) .* (x2z + (-1) .* x4z)) .^ 2) .^ (-1 / 2) .* ( ...
  ((x1x + (-1) .* x3x) .* ((x1x + (-1) .* x3x) .^ 2 + (x1y + (-1) .* ...
   x3y) .^ 2 + (x1z + (-1) .* x3z) .^ 2) .^ (-1 / 2) + (x2x + (-1)  ...
  .* x4x) .* ((x2x + (-1) .* x4x) .^ 2 + (x2y + (-1) .* x4y) .^ 2 +  ...
  (x2z + (-1) .* x4z) .^ 2) .^ (-1 / 2)) .^ 2 + ((x1y + (-1) .* x3y) ...
   .* ((x1x + (-1) .* x3x) .^ 2 + (x1y + (-1) .* x3y) .^ 2 + (x1z +  ...
  (-1) .* x3z) .^ 2) .^ (-1 / 2) + (x2y + (-1) .* x4y) .* ((x2x + ( ...
  -1) .* x4x) .^ 2 + (x2y + (-1) .* x4y) .^ 2 + (x2z + (-1) .* x4z)  ...
  .^ 2) .^ (-1 / 2)) .^ 2 + (((x1x + (-1) .* x3x) .^ 2 + (x1y + (-1) ...
   .* x3y) .^ 2 + (x1z + (-1) .* x3z) .^ 2) .^ (-1 / 2) .* (x1z + ( ...
  -1) .* x3z) + ((x2x + (-1) .* x4x) .^ 2 + (x2y + (-1) .* x4y) .^  ...
  2 + (x2z + (-1) .* x4z) .^ 2) .^ (-1 / 2) .* (x2z + (-1) .* x4z))  ...
  .^ 2) .^ (-1 / 2) + (-1 / 2) .* (((-1) .* x1y + x3y) .* (x2x + ( ...
  -1) .* x4x) + (x1x + (-1) .* x3x) .* (x2y + (-1) .* x4y)) .* (((( ...
  -1) .* x1y + x3y) .* (x2x + (-1) .* x4x) + (x1x + (-1) .* x3x) .*  ...
  (x2y + (-1) .* x4y)) .^ 2 + ((x1z + (-1) .* x3z) .* (x2x + (-1) .* ...
   x4x) + (-1) .* (x1x + (-1) .* x3x) .* (x2z + (-1) .* x4z)) .^ 2 + ...
   (((-1) .* x1z + x3z) .* (x2y + (-1) .* x4y) + (x1y + (-1) .* x3y) ...
   .* (x2z + (-1) .* x4z)) .^ 2) .^ (-1 / 2) .* ((-2) .* (x1x + (-1) ...
   .* x3x) .* ((x1x + (-1) .* x3x) .^ 2 + (x1y + (-1) .* x3y) .^ 2 + ...
   (x1z + (-1) .* x3z) .^ 2) .^ (-3 / 2) .* (x1z + (-1) .* x3z) .* ( ...
  (x1x + (-1) .* x3x) .* ((x1x + (-1) .* x3x) .^ 2 + (x1y + (-1) .*  ...
  x3y) .^ 2 + (x1z + (-1) .* x3z) .^ 2) .^ (-1 / 2) + (x2x + (-1) .* ...
   x4x) .* ((x2x + (-1) .* x4x) .^ 2 + (x2y + (-1) .* x4y) .^ 2 + ( ...
  x2z + (-1) .* x4z) .^ 2) .^ (-1 / 2)) + (-2) .* (x1y + (-1) .*  ...
  x3y) .* ((x1x + (-1) .* x3x) .^ 2 + (x1y + (-1) .* x3y) .^ 2 + ( ...
  x1z + (-1) .* x3z) .^ 2) .^ (-3 / 2) .* (x1z + (-1) .* x3z) .* (( ...
  x1y + (-1) .* x3y) .* ((x1x + (-1) .* x3x) .^ 2 + (x1y + (-1) .*  ...
  x3y) .^ 2 + (x1z + (-1) .* x3z) .^ 2) .^ (-1 / 2) + (x2y + (-1) .* ...
   x4y) .* ((x2x + (-1) .* x4x) .^ 2 + (x2y + (-1) .* x4y) .^ 2 + ( ...
  x2z + (-1) .* x4z) .^ 2) .^ (-1 / 2)) + 2 .* (((x1x + (-1) .* x3x) ...
   .^ 2 + (x1y + (-1) .* x3y) .^ 2 + (x1z + (-1) .* x3z) .^ 2) .^ ( ...
  -1 / 2) + (-1) .* ((x1x + (-1) .* x3x) .^ 2 + (x1y + (-1) .* x3y)  ...
  .^ 2 + (x1z + (-1) .* x3z) .^ 2) .^ (-3 / 2) .* (x1z + (-1) .*  ...
  x3z) .^ 2) .* (((x1x + (-1) .* x3x) .^ 2 + (x1y + (-1) .* x3y) .^  ...
  2 + (x1z + (-1) .* x3z) .^ 2) .^ (-1 / 2) .* (x1z + (-1) .* x3z) + ...
   ((x2x + (-1) .* x4x) .^ 2 + (x2y + (-1) .* x4y) .^ 2 + (x2z + ( ...
  -1) .* x4z) .^ 2) .^ (-1 / 2) .* (x2z + (-1) .* x4z))) .* (((x1x + ...
   (-1) .* x3x) .* ((x1x + (-1) .* x3x) .^ 2 + (x1y + (-1) .* x3y)  ...
  .^ 2 + (x1z + (-1) .* x3z) .^ 2) .^ (-1 / 2) + (x2x + (-1) .* x4x) ...
   .* ((x2x + (-1) .* x4x) .^ 2 + (x2y + (-1) .* x4y) .^ 2 + (x2z +  ...
  (-1) .* x4z) .^ 2) .^ (-1 / 2)) .^ 2 + ((x1y + (-1) .* x3y) .* (( ...
  x1x + (-1) .* x3x) .^ 2 + (x1y + (-1) .* x3y) .^ 2 + (x1z + (-1)  ...
  .* x3z) .^ 2) .^ (-1 / 2) + (x2y + (-1) .* x4y) .* ((x2x + (-1) .* ...
   x4x) .^ 2 + (x2y + (-1) .* x4y) .^ 2 + (x2z + (-1) .* x4z) .^ 2)  ...
  .^ (-1 / 2)) .^ 2 + (((x1x + (-1) .* x3x) .^ 2 + (x1y + (-1) .*  ...
  x3y) .^ 2 + (x1z + (-1) .* x3z) .^ 2) .^ (-1 / 2) .* (x1z + (-1)  ...
  .* x3z) + ((x2x + (-1) .* x4x) .^ 2 + (x2y + (-1) .* x4y) .^ 2 + ( ...
  x2z + (-1) .* x4z) .^ 2) .^ (-1 / 2) .* (x2z + (-1) .* x4z)) .^ 2) ...
   .^ (-3 / 2) .* ((x1x + (-1) .* x3x) .* ((x1x + (-1) .* x3x) .^ 2  ...
  + (x1y + (-1) .* x3y) .^ 2 + (x1z + (-1) .* x3z) .^ 2) .^ (-1 / 2) ...
   + (x2x + (-1) .* x4x) .* ((x2x + (-1) .* x4x) .^ 2 + (x2y + (-1)  ...
  .* x4y) .^ 2 + (x2z + (-1) .* x4z) .^ 2) .^ (-1 / 2)) + (-1 / 2)  ...
  .* (((-1) .* x1y + x3y) .* (x2x + (-1) .* x4x) + (x1x + (-1) .*  ...
  x3x) .* (x2y + (-1) .* x4y)) .* (2 .* (x2x + (-1) .* x4x) .* (( ...
  x1z + (-1) .* x3z) .* (x2x + (-1) .* x4x) + (-1) .* (x1x + (-1) .* ...
   x3x) .* (x2z + (-1) .* x4z)) + 2 .* ((-1) .* x2y + x4y) .* (((-1) ...
   .* x1z + x3z) .* (x2y + (-1) .* x4y) + (x1y + (-1) .* x3y) .* ( ...
  x2z + (-1) .* x4z))) .* ((((-1) .* x1y + x3y) .* (x2x + (-1) .*  ...
  x4x) + (x1x + (-1) .* x3x) .* (x2y + (-1) .* x4y)) .^ 2 + ((x1z +  ...
  (-1) .* x3z) .* (x2x + (-1) .* x4x) + (-1) .* (x1x + (-1) .* x3x)  ...
  .* (x2z + (-1) .* x4z)) .^ 2 + (((-1) .* x1z + x3z) .* (x2y + (-1) ...
   .* x4y) + (x1y + (-1) .* x3y) .* (x2z + (-1) .* x4z)) .^ 2) .^ ( ...
  -3 / 2) .* (((x1x + (-1) .* x3x) .* ((x1x + (-1) .* x3x) .^ 2 + ( ...
  x1y + (-1) .* x3y) .^ 2 + (x1z + (-1) .* x3z) .^ 2) .^ (-1 / 2) +  ...
  (x2x + (-1) .* x4x) .* ((x2x + (-1) .* x4x) .^ 2 + (x2y + (-1) .*  ...
  x4y) .^ 2 + (x2z + (-1) .* x4z) .^ 2) .^ (-1 / 2)) .^ 2 + ((x1y +  ...
  (-1) .* x3y) .* ((x1x + (-1) .* x3x) .^ 2 + (x1y + (-1) .* x3y)  ...
  .^ 2 + (x1z + (-1) .* x3z) .^ 2) .^ (-1 / 2) + (x2y + (-1) .* x4y) ...
   .* ((x2x + (-1) .* x4x) .^ 2 + (x2y + (-1) .* x4y) .^ 2 + (x2z +  ...
  (-1) .* x4z) .^ 2) .^ (-1 / 2)) .^ 2 + (((x1x + (-1) .* x3x) .^ 2  ...
  + (x1y + (-1) .* x3y) .^ 2 + (x1z + (-1) .* x3z) .^ 2) .^ (-1 / 2) ...
   .* (x1z + (-1) .* x3z) + ((x2x + (-1) .* x4x) .^ 2 + (x2y + (-1)  ...
  .* x4y) .^ 2 + (x2z + (-1) .* x4z) .^ 2) .^ (-1 / 2) .* (x2z + ( ...
  -1) .* x4z)) .^ 2) .^ (-1 / 2) .* ((x1x + (-1) .* x3x) .* ((x1x +  ...
  (-1) .* x3x) .^ 2 + (x1y + (-1) .* x3y) .^ 2 + (x1z + (-1) .* x3z) ...
   .^ 2) .^ (-1 / 2) + (x2x + (-1) .* x4x) .* ((x2x + (-1) .* x4x)  ...
  .^ 2 + (x2y + (-1) .* x4y) .^ 2 + (x2z + (-1) .* x4z) .^ 2) .^ ( ...
  -1 / 2)) + (-1) .* (((x1x + (-1) .* x3x) .^ 2 + (x1y + (-1) .*  ...
  x3y) .^ 2 + (x1z + (-1) .* x3z) .^ 2) .^ (-1 / 2) + (-1) .* ((x1x  ...
  + (-1) .* x3x) .^ 2 + (x1y + (-1) .* x3y) .^ 2 + (x1z + (-1) .*  ...
  x3z) .^ 2) .^ (-3 / 2) .* (x1z + (-1) .* x3z) .^ 2) .* ((((-1) .*  ...
  x1y + x3y) .* (x2x + (-1) .* x4x) + (x1x + (-1) .* x3x) .* (x2y +  ...
  (-1) .* x4y)) .^ 2 + ((x1z + (-1) .* x3z) .* (x2x + (-1) .* x4x) + ...
   (-1) .* (x1x + (-1) .* x3x) .* (x2z + (-1) .* x4z)) .^ 2 + (((-1) ...
   .* x1z + x3z) .* (x2y + (-1) .* x4y) + (x1y + (-1) .* x3y) .* ( ...
  x2z + (-1) .* x4z)) .^ 2) .^ (-1 / 2) .* (((x1x + (-1) .* x3x) .*  ...
  ((x1x + (-1) .* x3x) .^ 2 + (x1y + (-1) .* x3y) .^ 2 + (x1z + (-1) ...
   .* x3z) .^ 2) .^ (-1 / 2) + (x2x + (-1) .* x4x) .* ((x2x + (-1)  ...
  .* x4x) .^ 2 + (x2y + (-1) .* x4y) .^ 2 + (x2z + (-1) .* x4z) .^  ...
  2) .^ (-1 / 2)) .^ 2 + ((x1y + (-1) .* x3y) .* ((x1x + (-1) .*  ...
  x3x) .^ 2 + (x1y + (-1) .* x3y) .^ 2 + (x1z + (-1) .* x3z) .^ 2)  ...
  .^ (-1 / 2) + (x2y + (-1) .* x4y) .* ((x2x + (-1) .* x4x) .^ 2 + ( ...
  x2y + (-1) .* x4y) .^ 2 + (x2z + (-1) .* x4z) .^ 2) .^ (-1 / 2))  ...
  .^ 2 + (((x1x + (-1) .* x3x) .^ 2 + (x1y + (-1) .* x3y) .^ 2 + ( ...
  x1z + (-1) .* x3z) .^ 2) .^ (-1 / 2) .* (x1z + (-1) .* x3z) + (( ...
  x2x + (-1) .* x4x) .^ 2 + (x2y + (-1) .* x4y) .^ 2 + (x2z + (-1)  ...
  .* x4z) .^ 2) .^ (-1 / 2) .* (x2z + (-1) .* x4z)) .^ 2) .^ (-1 /  ...
  2) .* (((-1) .* x1z + x3z) .* (x2y + (-1) .* x4y) + (x1y + (-1) .* ...
   x3y) .* (x2z + (-1) .* x4z)) + (-1) .* ((-1) .* x2y + x4y) .* ((( ...
  (-1) .* x1y + x3y) .* (x2x + (-1) .* x4x) + (x1x + (-1) .* x3x) .* ...
   (x2y + (-1) .* x4y)) .^ 2 + ((x1z + (-1) .* x3z) .* (x2x + (-1)  ...
  .* x4x) + (-1) .* (x1x + (-1) .* x3x) .* (x2z + (-1) .* x4z)) .^  ...
  2 + (((-1) .* x1z + x3z) .* (x2y + (-1) .* x4y) + (x1y + (-1) .*  ...
  x3y) .* (x2z + (-1) .* x4z)) .^ 2) .^ (-1 / 2) .* (((x1x + (-1) .* ...
   x3x) .* ((x1x + (-1) .* x3x) .^ 2 + (x1y + (-1) .* x3y) .^ 2 + ( ...
  x1z + (-1) .* x3z) .^ 2) .^ (-1 / 2) + (x2x + (-1) .* x4x) .* (( ...
  x2x + (-1) .* x4x) .^ 2 + (x2y + (-1) .* x4y) .^ 2 + (x2z + (-1)  ...
  .* x4z) .^ 2) .^ (-1 / 2)) .^ 2 + ((x1y + (-1) .* x3y) .* ((x1x +  ...
  (-1) .* x3x) .^ 2 + (x1y + (-1) .* x3y) .^ 2 + (x1z + (-1) .* x3z) ...
   .^ 2) .^ (-1 / 2) + (x2y + (-1) .* x4y) .* ((x2x + (-1) .* x4x)  ...
  .^ 2 + (x2y + (-1) .* x4y) .^ 2 + (x2z + (-1) .* x4z) .^ 2) .^ ( ...
  -1 / 2)) .^ 2 + (((x1x + (-1) .* x3x) .^ 2 + (x1y + (-1) .* x3y)  ...
  .^ 2 + (x1z + (-1) .* x3z) .^ 2) .^ (-1 / 2) .* (x1z + (-1) .*  ...
  x3z) + ((x2x + (-1) .* x4x) .^ 2 + (x2y + (-1) .* x4y) .^ 2 + ( ...
  x2z + (-1) .* x4z) .^ 2) .^ (-1 / 2) .* (x2z + (-1) .* x4z)) .^ 2) ...
   .^ (-1 / 2) .* (((x1x + (-1) .* x3x) .^ 2 + (x1y + (-1) .* x3y)  ...
  .^ 2 + (x1z + (-1) .* x3z) .^ 2) .^ (-1 / 2) .* (x1z + (-1) .*  ...
  x3z) + ((x2x + (-1) .* x4x) .^ 2 + (x2y + (-1) .* x4y) .^ 2 + ( ...
  x2z + (-1) .* x4z) .^ 2) .^ (-1 / 2) .* (x2z + (-1) .* x4z)) + (1  ...
  / 2) .* ((((-1) .* x1y + x3y) .* (x2x + (-1) .* x4x) + (x1x + (-1) ...
   .* x3x) .* (x2y + (-1) .* x4y)) .^ 2 + ((x1z + (-1) .* x3z) .* ( ...
  x2x + (-1) .* x4x) + (-1) .* (x1x + (-1) .* x3x) .* (x2z + (-1) .* ...
   x4z)) .^ 2 + (((-1) .* x1z + x3z) .* (x2y + (-1) .* x4y) + (x1y + ...
   (-1) .* x3y) .* (x2z + (-1) .* x4z)) .^ 2) .^ (-1 / 2) .* ((-2)  ...
  .* (x1x + (-1) .* x3x) .* ((x1x + (-1) .* x3x) .^ 2 + (x1y + (-1)  ...
  .* x3y) .^ 2 + (x1z + (-1) .* x3z) .^ 2) .^ (-3 / 2) .* (x1z + ( ...
  -1) .* x3z) .* ((x1x + (-1) .* x3x) .* ((x1x + (-1) .* x3x) .^ 2 + ...
   (x1y + (-1) .* x3y) .^ 2 + (x1z + (-1) .* x3z) .^ 2) .^ (-1 / 2)  ...
  + (x2x + (-1) .* x4x) .* ((x2x + (-1) .* x4x) .^ 2 + (x2y + (-1)  ...
  .* x4y) .^ 2 + (x2z + (-1) .* x4z) .^ 2) .^ (-1 / 2)) + (-2) .* ( ...
  x1y + (-1) .* x3y) .* ((x1x + (-1) .* x3x) .^ 2 + (x1y + (-1) .*  ...
  x3y) .^ 2 + (x1z + (-1) .* x3z) .^ 2) .^ (-3 / 2) .* (x1z + (-1)  ...
  .* x3z) .* ((x1y + (-1) .* x3y) .* ((x1x + (-1) .* x3x) .^ 2 + ( ...
  x1y + (-1) .* x3y) .^ 2 + (x1z + (-1) .* x3z) .^ 2) .^ (-1 / 2) +  ...
  (x2y + (-1) .* x4y) .* ((x2x + (-1) .* x4x) .^ 2 + (x2y + (-1) .*  ...
  x4y) .^ 2 + (x2z + (-1) .* x4z) .^ 2) .^ (-1 / 2)) + 2 .* (((x1x + ...
   (-1) .* x3x) .^ 2 + (x1y + (-1) .* x3y) .^ 2 + (x1z + (-1) .*  ...
  x3z) .^ 2) .^ (-1 / 2) + (-1) .* ((x1x + (-1) .* x3x) .^ 2 + (x1y  ...
  + (-1) .* x3y) .^ 2 + (x1z + (-1) .* x3z) .^ 2) .^ (-3 / 2) .* ( ...
  x1z + (-1) .* x3z) .^ 2) .* (((x1x + (-1) .* x3x) .^ 2 + (x1y + ( ...
  -1) .* x3y) .^ 2 + (x1z + (-1) .* x3z) .^ 2) .^ (-1 / 2) .* (x1z + ...
   (-1) .* x3z) + ((x2x + (-1) .* x4x) .^ 2 + (x2y + (-1) .* x4y)  ...
  .^ 2 + (x2z + (-1) .* x4z) .^ 2) .^ (-1 / 2) .* (x2z + (-1) .*  ...
  x4z))) .* (((x1x + (-1) .* x3x) .* ((x1x + (-1) .* x3x) .^ 2 + ( ...
  x1y + (-1) .* x3y) .^ 2 + (x1z + (-1) .* x3z) .^ 2) .^ (-1 / 2) +  ...
  (x2x + (-1) .* x4x) .* ((x2x + (-1) .* x4x) .^ 2 + (x2y + (-1) .*  ...
  x4y) .^ 2 + (x2z + (-1) .* x4z) .^ 2) .^ (-1 / 2)) .^ 2 + ((x1y +  ...
  (-1) .* x3y) .* ((x1x + (-1) .* x3x) .^ 2 + (x1y + (-1) .* x3y)  ...
  .^ 2 + (x1z + (-1) .* x3z) .^ 2) .^ (-1 / 2) + (x2y + (-1) .* x4y) ...
   .* ((x2x + (-1) .* x4x) .^ 2 + (x2y + (-1) .* x4y) .^ 2 + (x2z +  ...
  (-1) .* x4z) .^ 2) .^ (-1 / 2)) .^ 2 + (((x1x + (-1) .* x3x) .^ 2  ...
  + (x1y + (-1) .* x3y) .^ 2 + (x1z + (-1) .* x3z) .^ 2) .^ (-1 / 2) ...
   .* (x1z + (-1) .* x3z) + ((x2x + (-1) .* x4x) .^ 2 + (x2y + (-1)  ...
  .* x4y) .^ 2 + (x2z + (-1) .* x4z) .^ 2) .^ (-1 / 2) .* (x2z + ( ...
  -1) .* x4z)) .^ 2) .^ (-3 / 2) .* (((-1) .* x1z + x3z) .* (x2y + ( ...
  -1) .* x4y) + (x1y + (-1) .* x3y) .* (x2z + (-1) .* x4z)) .* ((( ...
  x1x + (-1) .* x3x) .^ 2 + (x1y + (-1) .* x3y) .^ 2 + (x1z + (-1)  ...
  .* x3z) .^ 2) .^ (-1 / 2) .* (x1z + (-1) .* x3z) + ((x2x + (-1) .* ...
   x4x) .^ 2 + (x2y + (-1) .* x4y) .^ 2 + (x2z + (-1) .* x4z) .^ 2)  ...
  .^ (-1 / 2) .* (x2z + (-1) .* x4z)) + (1 / 2) .* (2 .* (x2x + (-1) ...
   .* x4x) .* ((x1z + (-1) .* x3z) .* (x2x + (-1) .* x4x) + (-1) .*  ...
  (x1x + (-1) .* x3x) .* (x2z + (-1) .* x4z)) + 2 .* ((-1) .* x2y +  ...
  x4y) .* (((-1) .* x1z + x3z) .* (x2y + (-1) .* x4y) + (x1y + (-1)  ...
  .* x3y) .* (x2z + (-1) .* x4z))) .* ((((-1) .* x1y + x3y) .* (x2x  ...
  + (-1) .* x4x) + (x1x + (-1) .* x3x) .* (x2y + (-1) .* x4y)) .^ 2  ...
  + ((x1z + (-1) .* x3z) .* (x2x + (-1) .* x4x) + (-1) .* (x1x + ( ...
  -1) .* x3x) .* (x2z + (-1) .* x4z)) .^ 2 + (((-1) .* x1z + x3z) .* ...
   (x2y + (-1) .* x4y) + (x1y + (-1) .* x3y) .* (x2z + (-1) .* x4z)) ...
   .^ 2) .^ (-3 / 2) .* (((x1x + (-1) .* x3x) .* ((x1x + (-1) .*  ...
  x3x) .^ 2 + (x1y + (-1) .* x3y) .^ 2 + (x1z + (-1) .* x3z) .^ 2)  ...
  .^ (-1 / 2) + (x2x + (-1) .* x4x) .* ((x2x + (-1) .* x4x) .^ 2 + ( ...
  x2y + (-1) .* x4y) .^ 2 + (x2z + (-1) .* x4z) .^ 2) .^ (-1 / 2))  ...
  .^ 2 + ((x1y + (-1) .* x3y) .* ((x1x + (-1) .* x3x) .^ 2 + (x1y +  ...
  (-1) .* x3y) .^ 2 + (x1z + (-1) .* x3z) .^ 2) .^ (-1 / 2) + (x2y + ...
   (-1) .* x4y) .* ((x2x + (-1) .* x4x) .^ 2 + (x2y + (-1) .* x4y)  ...
  .^ 2 + (x2z + (-1) .* x4z) .^ 2) .^ (-1 / 2)) .^ 2 + (((x1x + (-1) ...
   .* x3x) .^ 2 + (x1y + (-1) .* x3y) .^ 2 + (x1z + (-1) .* x3z) .^  ...
  2) .^ (-1 / 2) .* (x1z + (-1) .* x3z) + ((x2x + (-1) .* x4x) .^ 2  ...
  + (x2y + (-1) .* x4y) .^ 2 + (x2z + (-1) .* x4z) .^ 2) .^ (-1 / 2) ...
   .* (x2z + (-1) .* x4z)) .^ 2) .^ (-1 / 2) .* (((-1) .* x1z + x3z) ...
   .* (x2y + (-1) .* x4y) + (x1y + (-1) .* x3y) .* (x2z + (-1) .*  ...
  x4z)) .* (((x1x + (-1) .* x3x) .^ 2 + (x1y + (-1) .* x3y) .^ 2 + ( ...
  x1z + (-1) .* x3z) .^ 2) .^ (-1 / 2) .* (x1z + (-1) .* x3z) + (( ...
  x2x + (-1) .* x4x) .^ 2 + (x2y + (-1) .* x4y) .^ 2 + (x2z + (-1)  ...
  .* x4z) .^ 2) .^ (-1 / 2) .* (x2z + (-1) .* x4z)),(((-1) .* x1y +  ...
  x3y) .* (x2x + (-1) .* x4x) + (x1x + (-1) .* x3x) .* (x2y + (-1)  ...
  .* x4y)) .* ((((-1) .* x1y + x3y) .* (x2x + (-1) .* x4x) + (x1x +  ...
  (-1) .* x3x) .* (x2y + (-1) .* x4y)) .^ 2 + ((x1z + (-1) .* x3z)  ...
  .* (x2x + (-1) .* x4x) + (-1) .* (x1x + (-1) .* x3x) .* (x2z + ( ...
  -1) .* x4z)) .^ 2 + (((-1) .* x1z + x3z) .* (x2y + (-1) .* x4y) +  ...
  (x1y + (-1) .* x3y) .* (x2z + (-1) .* x4z)) .^ 2) .^ (-1 / 2) .* ( ...
  ((x1x + (-1) .* x3x) .* ((x1x + (-1) .* x3x) .^ 2 + (x1y + (-1) .* ...
   x3y) .^ 2 + (x1z + (-1) .* x3z) .^ 2) .^ (-1 / 2) + (x2x + (-1)  ...
  .* x4x) .* ((x2x + (-1) .* x4x) .^ 2 + (x2y + (-1) .* x4y) .^ 2 +  ...
  (x2z + (-1) .* x4z) .^ 2) .^ (-1 / 2)) .^ 2 + ((x1y + (-1) .* x3y) ...
   .* ((x1x + (-1) .* x3x) .^ 2 + (x1y + (-1) .* x3y) .^ 2 + (x1z +  ...
  (-1) .* x3z) .^ 2) .^ (-1 / 2) + (x2y + (-1) .* x4y) .* ((x2x + ( ...
  -1) .* x4x) .^ 2 + (x2y + (-1) .* x4y) .^ 2 + (x2z + (-1) .* x4z)  ...
  .^ 2) .^ (-1 / 2)) .^ 2 + (((x1x + (-1) .* x3x) .^ 2 + (x1y + (-1) ...
   .* x3y) .^ 2 + (x1z + (-1) .* x3z) .^ 2) .^ (-1 / 2) .* (x1z + ( ...
  -1) .* x3z) + ((x2x + (-1) .* x4x) .^ 2 + (x2y + (-1) .* x4y) .^  ...
  2 + (x2z + (-1) .* x4z) .^ 2) .^ (-1 / 2) .* (x2z + (-1) .* x4z))  ...
  .^ 2) .^ (-1 / 2) .* ((-1) .* (x2x + (-1) .* x4x) .^ 2 .* ((x2x +  ...
  (-1) .* x4x) .^ 2 + (x2y + (-1) .* x4y) .^ 2 + (x2z + (-1) .* x4z) ...
   .^ 2) .^ (-3 / 2) + ((x2x + (-1) .* x4x) .^ 2 + (x2y + (-1) .*  ...
  x4y) .^ 2 + (x2z + (-1) .* x4z) .^ 2) .^ (-1 / 2)) + (-1 / 2) .* ( ...
  ((-1) .* x1y + x3y) .* (x2x + (-1) .* x4x) + (x1x + (-1) .* x3x)  ...
  .* (x2y + (-1) .* x4y)) .* (2 .* ((-1) .* x1y + x3y) .* (((-1) .*  ...
  x1y + x3y) .* (x2x + (-1) .* x4x) + (x1x + (-1) .* x3x) .* (x2y +  ...
  (-1) .* x4y)) + 2 .* (x1z + (-1) .* x3z) .* ((x1z + (-1) .* x3z)  ...
  .* (x2x + (-1) .* x4x) + (-1) .* (x1x + (-1) .* x3x) .* (x2z + ( ...
  -1) .* x4z))) .* ((((-1) .* x1y + x3y) .* (x2x + (-1) .* x4x) + ( ...
  x1x + (-1) .* x3x) .* (x2y + (-1) .* x4y)) .^ 2 + ((x1z + (-1) .*  ...
  x3z) .* (x2x + (-1) .* x4x) + (-1) .* (x1x + (-1) .* x3x) .* (x2z  ...
  + (-1) .* x4z)) .^ 2 + (((-1) .* x1z + x3z) .* (x2y + (-1) .* x4y) ...
   + (x1y + (-1) .* x3y) .* (x2z + (-1) .* x4z)) .^ 2) .^ (-3 / 2)  ...
  .* (((x1x + (-1) .* x3x) .* ((x1x + (-1) .* x3x) .^ 2 + (x1y + ( ...
  -1) .* x3y) .^ 2 + (x1z + (-1) .* x3z) .^ 2) .^ (-1 / 2) + (x2x +  ...
  (-1) .* x4x) .* ((x2x + (-1) .* x4x) .^ 2 + (x2y + (-1) .* x4y)  ...
  .^ 2 + (x2z + (-1) .* x4z) .^ 2) .^ (-1 / 2)) .^ 2 + ((x1y + (-1)  ...
  .* x3y) .* ((x1x + (-1) .* x3x) .^ 2 + (x1y + (-1) .* x3y) .^ 2 +  ...
  (x1z + (-1) .* x3z) .^ 2) .^ (-1 / 2) + (x2y + (-1) .* x4y) .* (( ...
  x2x + (-1) .* x4x) .^ 2 + (x2y + (-1) .* x4y) .^ 2 + (x2z + (-1)  ...
  .* x4z) .^ 2) .^ (-1 / 2)) .^ 2 + (((x1x + (-1) .* x3x) .^ 2 + ( ...
  x1y + (-1) .* x3y) .^ 2 + (x1z + (-1) .* x3z) .^ 2) .^ (-1 / 2) .* ...
   (x1z + (-1) .* x3z) + ((x2x + (-1) .* x4x) .^ 2 + (x2y + (-1) .*  ...
  x4y) .^ 2 + (x2z + (-1) .* x4z) .^ 2) .^ (-1 / 2) .* (x2z + (-1)  ...
  .* x4z)) .^ 2) .^ (-1 / 2) .* ((x1x + (-1) .* x3x) .* ((x1x + (-1) ...
   .* x3x) .^ 2 + (x1y + (-1) .* x3y) .^ 2 + (x1z + (-1) .* x3z) .^  ...
  2) .^ (-1 / 2) + (x2x + (-1) .* x4x) .* ((x2x + (-1) .* x4x) .^ 2  ...
  + (x2y + (-1) .* x4y) .^ 2 + (x2z + (-1) .* x4z) .^ 2) .^ (-1 / 2) ...
  ) + ((-1) .* x1y + x3y) .* ((((-1) .* x1y + x3y) .* (x2x + (-1) .* ...
   x4x) + (x1x + (-1) .* x3x) .* (x2y + (-1) .* x4y)) .^ 2 + ((x1z + ...
   (-1) .* x3z) .* (x2x + (-1) .* x4x) + (-1) .* (x1x + (-1) .* x3x) ...
   .* (x2z + (-1) .* x4z)) .^ 2 + (((-1) .* x1z + x3z) .* (x2y + ( ...
  -1) .* x4y) + (x1y + (-1) .* x3y) .* (x2z + (-1) .* x4z)) .^ 2)  ...
  .^ (-1 / 2) .* (((x1x + (-1) .* x3x) .* ((x1x + (-1) .* x3x) .^ 2  ...
  + (x1y + (-1) .* x3y) .^ 2 + (x1z + (-1) .* x3z) .^ 2) .^ (-1 / 2) ...
   + (x2x + (-1) .* x4x) .* ((x2x + (-1) .* x4x) .^ 2 + (x2y + (-1)  ...
  .* x4y) .^ 2 + (x2z + (-1) .* x4z) .^ 2) .^ (-1 / 2)) .^ 2 + (( ...
  x1y + (-1) .* x3y) .* ((x1x + (-1) .* x3x) .^ 2 + (x1y + (-1) .*  ...
  x3y) .^ 2 + (x1z + (-1) .* x3z) .^ 2) .^ (-1 / 2) + (x2y + (-1) .* ...
   x4y) .* ((x2x + (-1) .* x4x) .^ 2 + (x2y + (-1) .* x4y) .^ 2 + ( ...
  x2z + (-1) .* x4z) .^ 2) .^ (-1 / 2)) .^ 2 + (((x1x + (-1) .* x3x) ...
   .^ 2 + (x1y + (-1) .* x3y) .^ 2 + (x1z + (-1) .* x3z) .^ 2) .^ ( ...
  -1 / 2) .* (x1z + (-1) .* x3z) + ((x2x + (-1) .* x4x) .^ 2 + (x2y  ...
  + (-1) .* x4y) .^ 2 + (x2z + (-1) .* x4z) .^ 2) .^ (-1 / 2) .* ( ...
  x2z + (-1) .* x4z)) .^ 2) .^ (-1 / 2) .* ((x1x + (-1) .* x3x) .* ( ...
  (x1x + (-1) .* x3x) .^ 2 + (x1y + (-1) .* x3y) .^ 2 + (x1z + (-1)  ...
  .* x3z) .^ 2) .^ (-1 / 2) + (x2x + (-1) .* x4x) .* ((x2x + (-1) .* ...
   x4x) .^ 2 + (x2y + (-1) .* x4y) .^ 2 + (x2z + (-1) .* x4z) .^ 2)  ...
  .^ (-1 / 2)) + (-1 / 2) .* (((-1) .* x1y + x3y) .* (x2x + (-1) .*  ...
  x4x) + (x1x + (-1) .* x3x) .* (x2y + (-1) .* x4y)) .* ((((-1) .*  ...
  x1y + x3y) .* (x2x + (-1) .* x4x) + (x1x + (-1) .* x3x) .* (x2y +  ...
  (-1) .* x4y)) .^ 2 + ((x1z + (-1) .* x3z) .* (x2x + (-1) .* x4x) + ...
   (-1) .* (x1x + (-1) .* x3x) .* (x2z + (-1) .* x4z)) .^ 2 + (((-1) ...
   .* x1z + x3z) .* (x2y + (-1) .* x4y) + (x1y + (-1) .* x3y) .* ( ...
  x2z + (-1) .* x4z)) .^ 2) .^ (-1 / 2) .* (((x1x + (-1) .* x3x) .*  ...
  ((x1x + (-1) .* x3x) .^ 2 + (x1y + (-1) .* x3y) .^ 2 + (x1z + (-1) ...
   .* x3z) .^ 2) .^ (-1 / 2) + (x2x + (-1) .* x4x) .* ((x2x + (-1)  ...
  .* x4x) .^ 2 + (x2y + (-1) .* x4y) .^ 2 + (x2z + (-1) .* x4z) .^  ...
  2) .^ (-1 / 2)) .^ 2 + ((x1y + (-1) .* x3y) .* ((x1x + (-1) .*  ...
  x3x) .^ 2 + (x1y + (-1) .* x3y) .^ 2 + (x1z + (-1) .* x3z) .^ 2)  ...
  .^ (-1 / 2) + (x2y + (-1) .* x4y) .* ((x2x + (-1) .* x4x) .^ 2 + ( ...
  x2y + (-1) .* x4y) .^ 2 + (x2z + (-1) .* x4z) .^ 2) .^ (-1 / 2))  ...
  .^ 2 + (((x1x + (-1) .* x3x) .^ 2 + (x1y + (-1) .* x3y) .^ 2 + ( ...
  x1z + (-1) .* x3z) .^ 2) .^ (-1 / 2) .* (x1z + (-1) .* x3z) + (( ...
  x2x + (-1) .* x4x) .^ 2 + (x2y + (-1) .* x4y) .^ 2 + (x2z + (-1)  ...
  .* x4z) .^ 2) .^ (-1 / 2) .* (x2z + (-1) .* x4z)) .^ 2) .^ (-3 /  ...
  2) .* ((x1x + (-1) .* x3x) .* ((x1x + (-1) .* x3x) .^ 2 + (x1y + ( ...
  -1) .* x3y) .^ 2 + (x1z + (-1) .* x3z) .^ 2) .^ (-1 / 2) + (x2x +  ...
  (-1) .* x4x) .* ((x2x + (-1) .* x4x) .^ 2 + (x2y + (-1) .* x4y)  ...
  .^ 2 + (x2z + (-1) .* x4z) .^ 2) .^ (-1 / 2)) .* (2 .* ((-1) .* ( ...
  x2x + (-1) .* x4x) .^ 2 .* ((x2x + (-1) .* x4x) .^ 2 + (x2y + (-1) ...
   .* x4y) .^ 2 + (x2z + (-1) .* x4z) .^ 2) .^ (-3 / 2) + ((x2x + ( ...
  -1) .* x4x) .^ 2 + (x2y + (-1) .* x4y) .^ 2 + (x2z + (-1) .* x4z)  ...
  .^ 2) .^ (-1 / 2)) .* ((x1x + (-1) .* x3x) .* ((x1x + (-1) .* x3x) ...
   .^ 2 + (x1y + (-1) .* x3y) .^ 2 + (x1z + (-1) .* x3z) .^ 2) .^ ( ...
  -1 / 2) + (x2x + (-1) .* x4x) .* ((x2x + (-1) .* x4x) .^ 2 + (x2y  ...
  + (-1) .* x4y) .^ 2 + (x2z + (-1) .* x4z) .^ 2) .^ (-1 / 2)) + ( ...
  -2) .* (x2x + (-1) .* x4x) .* (x2y + (-1) .* x4y) .* ((x1y + (-1)  ...
  .* x3y) .* ((x1x + (-1) .* x3x) .^ 2 + (x1y + (-1) .* x3y) .^ 2 +  ...
  (x1z + (-1) .* x3z) .^ 2) .^ (-1 / 2) + (x2y + (-1) .* x4y) .* (( ...
  x2x + (-1) .* x4x) .^ 2 + (x2y + (-1) .* x4y) .^ 2 + (x2z + (-1)  ...
  .* x4z) .^ 2) .^ (-1 / 2)) .* ((x2x + (-1) .* x4x) .^ 2 + (x2y + ( ...
  -1) .* x4y) .^ 2 + (x2z + (-1) .* x4z) .^ 2) .^ (-3 / 2) + (-2) .* ...
   (x2x + (-1) .* x4x) .* (((x1x + (-1) .* x3x) .^ 2 + (x1y + (-1)  ...
  .* x3y) .^ 2 + (x1z + (-1) .* x3z) .^ 2) .^ (-1 / 2) .* (x1z + ( ...
  -1) .* x3z) + ((x2x + (-1) .* x4x) .^ 2 + (x2y + (-1) .* x4y) .^  ...
  2 + (x2z + (-1) .* x4z) .^ 2) .^ (-1 / 2) .* (x2z + (-1) .* x4z))  ...
  .* ((x2x + (-1) .* x4x) .^ 2 + (x2y + (-1) .* x4y) .^ 2 + (x2z + ( ...
  -1) .* x4z) .^ 2) .^ (-3 / 2) .* (x2z + (-1) .* x4z)) + (1 / 2) .* ...
   (2 .* ((-1) .* x1y + x3y) .* (((-1) .* x1y + x3y) .* (x2x + (-1)  ...
  .* x4x) + (x1x + (-1) .* x3x) .* (x2y + (-1) .* x4y)) + 2 .* (x1z  ...
  + (-1) .* x3z) .* ((x1z + (-1) .* x3z) .* (x2x + (-1) .* x4x) + ( ...
  -1) .* (x1x + (-1) .* x3x) .* (x2z + (-1) .* x4z))) .* ((((-1) .*  ...
  x1y + x3y) .* (x2x + (-1) .* x4x) + (x1x + (-1) .* x3x) .* (x2y +  ...
  (-1) .* x4y)) .^ 2 + ((x1z + (-1) .* x3z) .* (x2x + (-1) .* x4x) + ...
   (-1) .* (x1x + (-1) .* x3x) .* (x2z + (-1) .* x4z)) .^ 2 + (((-1) ...
   .* x1z + x3z) .* (x2y + (-1) .* x4y) + (x1y + (-1) .* x3y) .* ( ...
  x2z + (-1) .* x4z)) .^ 2) .^ (-3 / 2) .* (((x1x + (-1) .* x3x) .*  ...
  ((x1x + (-1) .* x3x) .^ 2 + (x1y + (-1) .* x3y) .^ 2 + (x1z + (-1) ...
   .* x3z) .^ 2) .^ (-1 / 2) + (x2x + (-1) .* x4x) .* ((x2x + (-1)  ...
  .* x4x) .^ 2 + (x2y + (-1) .* x4y) .^ 2 + (x2z + (-1) .* x4z) .^  ...
  2) .^ (-1 / 2)) .^ 2 + ((x1y + (-1) .* x3y) .* ((x1x + (-1) .*  ...
  x3x) .^ 2 + (x1y + (-1) .* x3y) .^ 2 + (x1z + (-1) .* x3z) .^ 2)  ...
  .^ (-1 / 2) + (x2y + (-1) .* x4y) .* ((x2x + (-1) .* x4x) .^ 2 + ( ...
  x2y + (-1) .* x4y) .^ 2 + (x2z + (-1) .* x4z) .^ 2) .^ (-1 / 2))  ...
  .^ 2 + (((x1x + (-1) .* x3x) .^ 2 + (x1y + (-1) .* x3y) .^ 2 + ( ...
  x1z + (-1) .* x3z) .^ 2) .^ (-1 / 2) .* (x1z + (-1) .* x3z) + (( ...
  x2x + (-1) .* x4x) .^ 2 + (x2y + (-1) .* x4y) .^ 2 + (x2z + (-1)  ...
  .* x4z) .^ 2) .^ (-1 / 2) .* (x2z + (-1) .* x4z)) .^ 2) .^ (-1 /  ...
  2) .* (((-1) .* x1z + x3z) .* (x2y + (-1) .* x4y) + (x1y + (-1) .* ...
   x3y) .* (x2z + (-1) .* x4z)) .* (((x1x + (-1) .* x3x) .^ 2 + ( ...
  x1y + (-1) .* x3y) .^ 2 + (x1z + (-1) .* x3z) .^ 2) .^ (-1 / 2) .* ...
   (x1z + (-1) .* x3z) + ((x2x + (-1) .* x4x) .^ 2 + (x2y + (-1) .*  ...
  x4y) .^ 2 + (x2z + (-1) .* x4z) .^ 2) .^ (-1 / 2) .* (x2z + (-1)  ...
  .* x4z)) + (1 / 2) .* ((((-1) .* x1y + x3y) .* (x2x + (-1) .* x4x) ...
   + (x1x + (-1) .* x3x) .* (x2y + (-1) .* x4y)) .^ 2 + ((x1z + (-1) ...
   .* x3z) .* (x2x + (-1) .* x4x) + (-1) .* (x1x + (-1) .* x3x) .* ( ...
  x2z + (-1) .* x4z)) .^ 2 + (((-1) .* x1z + x3z) .* (x2y + (-1) .*  ...
  x4y) + (x1y + (-1) .* x3y) .* (x2z + (-1) .* x4z)) .^ 2) .^ (-1 /  ...
  2) .* (((x1x + (-1) .* x3x) .* ((x1x + (-1) .* x3x) .^ 2 + (x1y +  ...
  (-1) .* x3y) .^ 2 + (x1z + (-1) .* x3z) .^ 2) .^ (-1 / 2) + (x2x + ...
   (-1) .* x4x) .* ((x2x + (-1) .* x4x) .^ 2 + (x2y + (-1) .* x4y)  ...
  .^ 2 + (x2z + (-1) .* x4z) .^ 2) .^ (-1 / 2)) .^ 2 + ((x1y + (-1)  ...
  .* x3y) .* ((x1x + (-1) .* x3x) .^ 2 + (x1y + (-1) .* x3y) .^ 2 +  ...
  (x1z + (-1) .* x3z) .^ 2) .^ (-1 / 2) + (x2y + (-1) .* x4y) .* (( ...
  x2x + (-1) .* x4x) .^ 2 + (x2y + (-1) .* x4y) .^ 2 + (x2z + (-1)  ...
  .* x4z) .^ 2) .^ (-1 / 2)) .^ 2 + (((x1x + (-1) .* x3x) .^ 2 + ( ...
  x1y + (-1) .* x3y) .^ 2 + (x1z + (-1) .* x3z) .^ 2) .^ (-1 / 2) .* ...
   (x1z + (-1) .* x3z) + ((x2x + (-1) .* x4x) .^ 2 + (x2y + (-1) .*  ...
  x4y) .^ 2 + (x2z + (-1) .* x4z) .^ 2) .^ (-1 / 2) .* (x2z + (-1)  ...
  .* x4z)) .^ 2) .^ (-3 / 2) .* (((-1) .* x1z + x3z) .* (x2y + (-1)  ...
  .* x4y) + (x1y + (-1) .* x3y) .* (x2z + (-1) .* x4z)) .* (2 .* (( ...
  -1) .* (x2x + (-1) .* x4x) .^ 2 .* ((x2x + (-1) .* x4x) .^ 2 + ( ...
  x2y + (-1) .* x4y) .^ 2 + (x2z + (-1) .* x4z) .^ 2) .^ (-3 / 2) +  ...
  ((x2x + (-1) .* x4x) .^ 2 + (x2y + (-1) .* x4y) .^ 2 + (x2z + (-1) ...
   .* x4z) .^ 2) .^ (-1 / 2)) .* ((x1x + (-1) .* x3x) .* ((x1x + ( ...
  -1) .* x3x) .^ 2 + (x1y + (-1) .* x3y) .^ 2 + (x1z + (-1) .* x3z)  ...
  .^ 2) .^ (-1 / 2) + (x2x + (-1) .* x4x) .* ((x2x + (-1) .* x4x)  ...
  .^ 2 + (x2y + (-1) .* x4y) .^ 2 + (x2z + (-1) .* x4z) .^ 2) .^ ( ...
  -1 / 2)) + (-2) .* (x2x + (-1) .* x4x) .* (x2y + (-1) .* x4y) .* ( ...
  (x1y + (-1) .* x3y) .* ((x1x + (-1) .* x3x) .^ 2 + (x1y + (-1) .*  ...
  x3y) .^ 2 + (x1z + (-1) .* x3z) .^ 2) .^ (-1 / 2) + (x2y + (-1) .* ...
   x4y) .* ((x2x + (-1) .* x4x) .^ 2 + (x2y + (-1) .* x4y) .^ 2 + ( ...
  x2z + (-1) .* x4z) .^ 2) .^ (-1 / 2)) .* ((x2x + (-1) .* x4x) .^  ...
  2 + (x2y + (-1) .* x4y) .^ 2 + (x2z + (-1) .* x4z) .^ 2) .^ (-3 /  ...
  2) + (-2) .* (x2x + (-1) .* x4x) .* (((x1x + (-1) .* x3x) .^ 2 + ( ...
  x1y + (-1) .* x3y) .^ 2 + (x1z + (-1) .* x3z) .^ 2) .^ (-1 / 2) .* ...
   (x1z + (-1) .* x3z) + ((x2x + (-1) .* x4x) .^ 2 + (x2y + (-1) .*  ...
  x4y) .^ 2 + (x2z + (-1) .* x4z) .^ 2) .^ (-1 / 2) .* (x2z + (-1)  ...
  .* x4z)) .* ((x2x + (-1) .* x4x) .^ 2 + (x2y + (-1) .* x4y) .^ 2 + ...
   (x2z + (-1) .* x4z) .^ 2) .^ (-3 / 2) .* (x2z + (-1) .* x4z)) .*  ...
  (((x1x + (-1) .* x3x) .^ 2 + (x1y + (-1) .* x3y) .^ 2 + (x1z + ( ...
  -1) .* x3z) .^ 2) .^ (-1 / 2) .* (x1z + (-1) .* x3z) + ((x2x + ( ...
  -1) .* x4x) .^ 2 + (x2y + (-1) .* x4y) .^ 2 + (x2z + (-1) .* x4z)  ...
  .^ 2) .^ (-1 / 2) .* (x2z + (-1) .* x4z)) + (x2x + (-1) .* x4x) .* ...
   ((((-1) .* x1y + x3y) .* (x2x + (-1) .* x4x) + (x1x + (-1) .*  ...
  x3x) .* (x2y + (-1) .* x4y)) .^ 2 + ((x1z + (-1) .* x3z) .* (x2x + ...
   (-1) .* x4x) + (-1) .* (x1x + (-1) .* x3x) .* (x2z + (-1) .* x4z) ...
  ) .^ 2 + (((-1) .* x1z + x3z) .* (x2y + (-1) .* x4y) + (x1y + (-1) ...
   .* x3y) .* (x2z + (-1) .* x4z)) .^ 2) .^ (-1 / 2) .* (((x1x + ( ...
  -1) .* x3x) .* ((x1x + (-1) .* x3x) .^ 2 + (x1y + (-1) .* x3y) .^  ...
  2 + (x1z + (-1) .* x3z) .^ 2) .^ (-1 / 2) + (x2x + (-1) .* x4x) .* ...
   ((x2x + (-1) .* x4x) .^ 2 + (x2y + (-1) .* x4y) .^ 2 + (x2z + ( ...
  -1) .* x4z) .^ 2) .^ (-1 / 2)) .^ 2 + ((x1y + (-1) .* x3y) .* (( ...
  x1x + (-1) .* x3x) .^ 2 + (x1y + (-1) .* x3y) .^ 2 + (x1z + (-1)  ...
  .* x3z) .^ 2) .^ (-1 / 2) + (x2y + (-1) .* x4y) .* ((x2x + (-1) .* ...
   x4x) .^ 2 + (x2y + (-1) .* x4y) .^ 2 + (x2z + (-1) .* x4z) .^ 2)  ...
  .^ (-1 / 2)) .^ 2 + (((x1x + (-1) .* x3x) .^ 2 + (x1y + (-1) .*  ...
  x3y) .^ 2 + (x1z + (-1) .* x3z) .^ 2) .^ (-1 / 2) .* (x1z + (-1)  ...
  .* x3z) + ((x2x + (-1) .* x4x) .^ 2 + (x2y + (-1) .* x4y) .^ 2 + ( ...
  x2z + (-1) .* x4z) .^ 2) .^ (-1 / 2) .* (x2z + (-1) .* x4z)) .^ 2) ...
   .^ (-1 / 2) .* (((-1) .* x1z + x3z) .* (x2y + (-1) .* x4y) + ( ...
  x1y + (-1) .* x3y) .* (x2z + (-1) .* x4z)) .* ((x2x + (-1) .* x4x) ...
   .^ 2 + (x2y + (-1) .* x4y) .^ 2 + (x2z + (-1) .* x4z) .^ 2) .^ ( ...
  -3 / 2) .* (x2z + (-1) .* x4z),(-1 / 2) .* (((-1) .* x1y + x3y) .* ...
   (x2x + (-1) .* x4x) + (x1x + (-1) .* x3x) .* (x2y + (-1) .* x4y)) ...
   .* (2 .* (x1x + (-1) .* x3x) .* (((-1) .* x1y + x3y) .* (x2x + ( ...
  -1) .* x4x) + (x1x + (-1) .* x3x) .* (x2y + (-1) .* x4y)) + 2 .* ( ...
  (-1) .* x1z + x3z) .* (((-1) .* x1z + x3z) .* (x2y + (-1) .* x4y)  ...
  + (x1y + (-1) .* x3y) .* (x2z + (-1) .* x4z))) .* ((((-1) .* x1y + ...
   x3y) .* (x2x + (-1) .* x4x) + (x1x + (-1) .* x3x) .* (x2y + (-1)  ...
  .* x4y)) .^ 2 + ((x1z + (-1) .* x3z) .* (x2x + (-1) .* x4x) + (-1) ...
   .* (x1x + (-1) .* x3x) .* (x2z + (-1) .* x4z)) .^ 2 + (((-1) .*  ...
  x1z + x3z) .* (x2y + (-1) .* x4y) + (x1y + (-1) .* x3y) .* (x2z +  ...
  (-1) .* x4z)) .^ 2) .^ (-3 / 2) .* (((x1x + (-1) .* x3x) .* ((x1x  ...
  + (-1) .* x3x) .^ 2 + (x1y + (-1) .* x3y) .^ 2 + (x1z + (-1) .*  ...
  x3z) .^ 2) .^ (-1 / 2) + (x2x + (-1) .* x4x) .* ((x2x + (-1) .*  ...
  x4x) .^ 2 + (x2y + (-1) .* x4y) .^ 2 + (x2z + (-1) .* x4z) .^ 2)  ...
  .^ (-1 / 2)) .^ 2 + ((x1y + (-1) .* x3y) .* ((x1x + (-1) .* x3x)  ...
  .^ 2 + (x1y + (-1) .* x3y) .^ 2 + (x1z + (-1) .* x3z) .^ 2) .^ ( ...
  -1 / 2) + (x2y + (-1) .* x4y) .* ((x2x + (-1) .* x4x) .^ 2 + (x2y  ...
  + (-1) .* x4y) .^ 2 + (x2z + (-1) .* x4z) .^ 2) .^ (-1 / 2)) .^ 2  ...
  + (((x1x + (-1) .* x3x) .^ 2 + (x1y + (-1) .* x3y) .^ 2 + (x1z + ( ...
  -1) .* x3z) .^ 2) .^ (-1 / 2) .* (x1z + (-1) .* x3z) + ((x2x + ( ...
  -1) .* x4x) .^ 2 + (x2y + (-1) .* x4y) .^ 2 + (x2z + (-1) .* x4z)  ...
  .^ 2) .^ (-1 / 2) .* (x2z + (-1) .* x4z)) .^ 2) .^ (-1 / 2) .* (( ...
  x1x + (-1) .* x3x) .* ((x1x + (-1) .* x3x) .^ 2 + (x1y + (-1) .*  ...
  x3y) .^ 2 + (x1z + (-1) .* x3z) .^ 2) .^ (-1 / 2) + (x2x + (-1) .* ...
   x4x) .* ((x2x + (-1) .* x4x) .^ 2 + (x2y + (-1) .* x4y) .^ 2 + ( ...
  x2z + (-1) .* x4z) .^ 2) .^ (-1 / 2)) + (x1x + (-1) .* x3x) .* ((( ...
  (-1) .* x1y + x3y) .* (x2x + (-1) .* x4x) + (x1x + (-1) .* x3x) .* ...
   (x2y + (-1) .* x4y)) .^ 2 + ((x1z + (-1) .* x3z) .* (x2x + (-1)  ...
  .* x4x) + (-1) .* (x1x + (-1) .* x3x) .* (x2z + (-1) .* x4z)) .^  ...
  2 + (((-1) .* x1z + x3z) .* (x2y + (-1) .* x4y) + (x1y + (-1) .*  ...
  x3y) .* (x2z + (-1) .* x4z)) .^ 2) .^ (-1 / 2) .* (((x1x + (-1) .* ...
   x3x) .* ((x1x + (-1) .* x3x) .^ 2 + (x1y + (-1) .* x3y) .^ 2 + ( ...
  x1z + (-1) .* x3z) .^ 2) .^ (-1 / 2) + (x2x + (-1) .* x4x) .* (( ...
  x2x + (-1) .* x4x) .^ 2 + (x2y + (-1) .* x4y) .^ 2 + (x2z + (-1)  ...
  .* x4z) .^ 2) .^ (-1 / 2)) .^ 2 + ((x1y + (-1) .* x3y) .* ((x1x +  ...
  (-1) .* x3x) .^ 2 + (x1y + (-1) .* x3y) .^ 2 + (x1z + (-1) .* x3z) ...
   .^ 2) .^ (-1 / 2) + (x2y + (-1) .* x4y) .* ((x2x + (-1) .* x4x)  ...
  .^ 2 + (x2y + (-1) .* x4y) .^ 2 + (x2z + (-1) .* x4z) .^ 2) .^ ( ...
  -1 / 2)) .^ 2 + (((x1x + (-1) .* x3x) .^ 2 + (x1y + (-1) .* x3y)  ...
  .^ 2 + (x1z + (-1) .* x3z) .^ 2) .^ (-1 / 2) .* (x1z + (-1) .*  ...
  x3z) + ((x2x + (-1) .* x4x) .^ 2 + (x2y + (-1) .* x4y) .^ 2 + ( ...
  x2z + (-1) .* x4z) .^ 2) .^ (-1 / 2) .* (x2z + (-1) .* x4z)) .^ 2) ...
   .^ (-1 / 2) .* ((x1x + (-1) .* x3x) .* ((x1x + (-1) .* x3x) .^ 2  ...
  + (x1y + (-1) .* x3y) .^ 2 + (x1z + (-1) .* x3z) .^ 2) .^ (-1 / 2) ...
   + (x2x + (-1) .* x4x) .* ((x2x + (-1) .* x4x) .^ 2 + (x2y + (-1)  ...
  .* x4y) .^ 2 + (x2z + (-1) .* x4z) .^ 2) .^ (-1 / 2)) + (-1 / 2)  ...
  .* (((-1) .* x1y + x3y) .* (x2x + (-1) .* x4x) + (x1x + (-1) .*  ...
  x3x) .* (x2y + (-1) .* x4y)) .* ((((-1) .* x1y + x3y) .* (x2x + ( ...
  -1) .* x4x) + (x1x + (-1) .* x3x) .* (x2y + (-1) .* x4y)) .^ 2 + ( ...
  (x1z + (-1) .* x3z) .* (x2x + (-1) .* x4x) + (-1) .* (x1x + (-1)  ...
  .* x3x) .* (x2z + (-1) .* x4z)) .^ 2 + (((-1) .* x1z + x3z) .* ( ...
  x2y + (-1) .* x4y) + (x1y + (-1) .* x3y) .* (x2z + (-1) .* x4z))  ...
  .^ 2) .^ (-1 / 2) .* (((x1x + (-1) .* x3x) .* ((x1x + (-1) .* x3x) ...
   .^ 2 + (x1y + (-1) .* x3y) .^ 2 + (x1z + (-1) .* x3z) .^ 2) .^ ( ...
  -1 / 2) + (x2x + (-1) .* x4x) .* ((x2x + (-1) .* x4x) .^ 2 + (x2y  ...
  + (-1) .* x4y) .^ 2 + (x2z + (-1) .* x4z) .^ 2) .^ (-1 / 2)) .^ 2  ...
  + ((x1y + (-1) .* x3y) .* ((x1x + (-1) .* x3x) .^ 2 + (x1y + (-1)  ...
  .* x3y) .^ 2 + (x1z + (-1) .* x3z) .^ 2) .^ (-1 / 2) + (x2y + (-1) ...
   .* x4y) .* ((x2x + (-1) .* x4x) .^ 2 + (x2y + (-1) .* x4y) .^ 2 + ...
   (x2z + (-1) .* x4z) .^ 2) .^ (-1 / 2)) .^ 2 + (((x1x + (-1) .*  ...
  x3x) .^ 2 + (x1y + (-1) .* x3y) .^ 2 + (x1z + (-1) .* x3z) .^ 2)  ...
  .^ (-1 / 2) .* (x1z + (-1) .* x3z) + ((x2x + (-1) .* x4x) .^ 2 + ( ...
  x2y + (-1) .* x4y) .^ 2 + (x2z + (-1) .* x4z) .^ 2) .^ (-1 / 2) .* ...
   (x2z + (-1) .* x4z)) .^ 2) .^ (-3 / 2) .* ((x1x + (-1) .* x3x) .* ...
   ((x1x + (-1) .* x3x) .^ 2 + (x1y + (-1) .* x3y) .^ 2 + (x1z + ( ...
  -1) .* x3z) .^ 2) .^ (-1 / 2) + (x2x + (-1) .* x4x) .* ((x2x + ( ...
  -1) .* x4x) .^ 2 + (x2y + (-1) .* x4y) .^ 2 + (x2z + (-1) .* x4z)  ...
  .^ 2) .^ (-1 / 2)) .* (2 .* ((-1) .* (x2y + (-1) .* x4y) .^ 2 .* ( ...
  (x2x + (-1) .* x4x) .^ 2 + (x2y + (-1) .* x4y) .^ 2 + (x2z + (-1)  ...
  .* x4z) .^ 2) .^ (-3 / 2) + ((x2x + (-1) .* x4x) .^ 2 + (x2y + ( ...
  -1) .* x4y) .^ 2 + (x2z + (-1) .* x4z) .^ 2) .^ (-1 / 2)) .* (( ...
  x1y + (-1) .* x3y) .* ((x1x + (-1) .* x3x) .^ 2 + (x1y + (-1) .*  ...
  x3y) .^ 2 + (x1z + (-1) .* x3z) .^ 2) .^ (-1 / 2) + (x2y + (-1) .* ...
   x4y) .* ((x2x + (-1) .* x4x) .^ 2 + (x2y + (-1) .* x4y) .^ 2 + ( ...
  x2z + (-1) .* x4z) .^ 2) .^ (-1 / 2)) + (-2) .* (x2x + (-1) .*  ...
  x4x) .* (x2y + (-1) .* x4y) .* ((x1x + (-1) .* x3x) .* ((x1x + ( ...
  -1) .* x3x) .^ 2 + (x1y + (-1) .* x3y) .^ 2 + (x1z + (-1) .* x3z)  ...
  .^ 2) .^ (-1 / 2) + (x2x + (-1) .* x4x) .* ((x2x + (-1) .* x4x)  ...
  .^ 2 + (x2y + (-1) .* x4y) .^ 2 + (x2z + (-1) .* x4z) .^ 2) .^ ( ...
  -1 / 2)) .* ((x2x + (-1) .* x4x) .^ 2 + (x2y + (-1) .* x4y) .^ 2 + ...
   (x2z + (-1) .* x4z) .^ 2) .^ (-3 / 2) + (-2) .* (x2y + (-1) .*  ...
  x4y) .* (((x1x + (-1) .* x3x) .^ 2 + (x1y + (-1) .* x3y) .^ 2 + ( ...
  x1z + (-1) .* x3z) .^ 2) .^ (-1 / 2) .* (x1z + (-1) .* x3z) + (( ...
  x2x + (-1) .* x4x) .^ 2 + (x2y + (-1) .* x4y) .^ 2 + (x2z + (-1)  ...
  .* x4z) .^ 2) .^ (-1 / 2) .* (x2z + (-1) .* x4z)) .* ((x2x + (-1)  ...
  .* x4x) .^ 2 + (x2y + (-1) .* x4y) .^ 2 + (x2z + (-1) .* x4z) .^  ...
  2) .^ (-3 / 2) .* (x2z + (-1) .* x4z)) + (-1) .* ((-1) .* x1z +  ...
  x3z) .* ((((-1) .* x1y + x3y) .* (x2x + (-1) .* x4x) + (x1x + (-1) ...
   .* x3x) .* (x2y + (-1) .* x4y)) .^ 2 + ((x1z + (-1) .* x3z) .* ( ...
  x2x + (-1) .* x4x) + (-1) .* (x1x + (-1) .* x3x) .* (x2z + (-1) .* ...
   x4z)) .^ 2 + (((-1) .* x1z + x3z) .* (x2y + (-1) .* x4y) + (x1y + ...
   (-1) .* x3y) .* (x2z + (-1) .* x4z)) .^ 2) .^ (-1 / 2) .* (((x1x  ...
  + (-1) .* x3x) .* ((x1x + (-1) .* x3x) .^ 2 + (x1y + (-1) .* x3y)  ...
  .^ 2 + (x1z + (-1) .* x3z) .^ 2) .^ (-1 / 2) + (x2x + (-1) .* x4x) ...
   .* ((x2x + (-1) .* x4x) .^ 2 + (x2y + (-1) .* x4y) .^ 2 + (x2z +  ...
  (-1) .* x4z) .^ 2) .^ (-1 / 2)) .^ 2 + ((x1y + (-1) .* x3y) .* (( ...
  x1x + (-1) .* x3x) .^ 2 + (x1y + (-1) .* x3y) .^ 2 + (x1z + (-1)  ...
  .* x3z) .^ 2) .^ (-1 / 2) + (x2y + (-1) .* x4y) .* ((x2x + (-1) .* ...
   x4x) .^ 2 + (x2y + (-1) .* x4y) .^ 2 + (x2z + (-1) .* x4z) .^ 2)  ...
  .^ (-1 / 2)) .^ 2 + (((x1x + (-1) .* x3x) .^ 2 + (x1y + (-1) .*  ...
  x3y) .^ 2 + (x1z + (-1) .* x3z) .^ 2) .^ (-1 / 2) .* (x1z + (-1)  ...
  .* x3z) + ((x2x + (-1) .* x4x) .^ 2 + (x2y + (-1) .* x4y) .^ 2 + ( ...
  x2z + (-1) .* x4z) .^ 2) .^ (-1 / 2) .* (x2z + (-1) .* x4z)) .^ 2) ...
   .^ (-1 / 2) .* (((x1x + (-1) .* x3x) .^ 2 + (x1y + (-1) .* x3y)  ...
  .^ 2 + (x1z + (-1) .* x3z) .^ 2) .^ (-1 / 2) .* (x1z + (-1) .*  ...
  x3z) + ((x2x + (-1) .* x4x) .^ 2 + (x2y + (-1) .* x4y) .^ 2 + ( ...
  x2z + (-1) .* x4z) .^ 2) .^ (-1 / 2) .* (x2z + (-1) .* x4z)) + (1  ...
  / 2) .* (2 .* (x1x + (-1) .* x3x) .* (((-1) .* x1y + x3y) .* (x2x  ...
  + (-1) .* x4x) + (x1x + (-1) .* x3x) .* (x2y + (-1) .* x4y)) + 2  ...
  .* ((-1) .* x1z + x3z) .* (((-1) .* x1z + x3z) .* (x2y + (-1) .*  ...
  x4y) + (x1y + (-1) .* x3y) .* (x2z + (-1) .* x4z))) .* ((((-1) .*  ...
  x1y + x3y) .* (x2x + (-1) .* x4x) + (x1x + (-1) .* x3x) .* (x2y +  ...
  (-1) .* x4y)) .^ 2 + ((x1z + (-1) .* x3z) .* (x2x + (-1) .* x4x) + ...
   (-1) .* (x1x + (-1) .* x3x) .* (x2z + (-1) .* x4z)) .^ 2 + (((-1) ...
   .* x1z + x3z) .* (x2y + (-1) .* x4y) + (x1y + (-1) .* x3y) .* ( ...
  x2z + (-1) .* x4z)) .^ 2) .^ (-3 / 2) .* (((x1x + (-1) .* x3x) .*  ...
  ((x1x + (-1) .* x3x) .^ 2 + (x1y + (-1) .* x3y) .^ 2 + (x1z + (-1) ...
   .* x3z) .^ 2) .^ (-1 / 2) + (x2x + (-1) .* x4x) .* ((x2x + (-1)  ...
  .* x4x) .^ 2 + (x2y + (-1) .* x4y) .^ 2 + (x2z + (-1) .* x4z) .^  ...
  2) .^ (-1 / 2)) .^ 2 + ((x1y + (-1) .* x3y) .* ((x1x + (-1) .*  ...
  x3x) .^ 2 + (x1y + (-1) .* x3y) .^ 2 + (x1z + (-1) .* x3z) .^ 2)  ...
  .^ (-1 / 2) + (x2y + (-1) .* x4y) .* ((x2x + (-1) .* x4x) .^ 2 + ( ...
  x2y + (-1) .* x4y) .^ 2 + (x2z + (-1) .* x4z) .^ 2) .^ (-1 / 2))  ...
  .^ 2 + (((x1x + (-1) .* x3x) .^ 2 + (x1y + (-1) .* x3y) .^ 2 + ( ...
  x1z + (-1) .* x3z) .^ 2) .^ (-1 / 2) .* (x1z + (-1) .* x3z) + (( ...
  x2x + (-1) .* x4x) .^ 2 + (x2y + (-1) .* x4y) .^ 2 + (x2z + (-1)  ...
  .* x4z) .^ 2) .^ (-1 / 2) .* (x2z + (-1) .* x4z)) .^ 2) .^ (-1 /  ...
  2) .* (((-1) .* x1z + x3z) .* (x2y + (-1) .* x4y) + (x1y + (-1) .* ...
   x3y) .* (x2z + (-1) .* x4z)) .* (((x1x + (-1) .* x3x) .^ 2 + ( ...
  x1y + (-1) .* x3y) .^ 2 + (x1z + (-1) .* x3z) .^ 2) .^ (-1 / 2) .* ...
   (x1z + (-1) .* x3z) + ((x2x + (-1) .* x4x) .^ 2 + (x2y + (-1) .*  ...
  x4y) .^ 2 + (x2z + (-1) .* x4z) .^ 2) .^ (-1 / 2) .* (x2z + (-1)  ...
  .* x4z)) + (1 / 2) .* ((((-1) .* x1y + x3y) .* (x2x + (-1) .* x4x) ...
   + (x1x + (-1) .* x3x) .* (x2y + (-1) .* x4y)) .^ 2 + ((x1z + (-1) ...
   .* x3z) .* (x2x + (-1) .* x4x) + (-1) .* (x1x + (-1) .* x3x) .* ( ...
  x2z + (-1) .* x4z)) .^ 2 + (((-1) .* x1z + x3z) .* (x2y + (-1) .*  ...
  x4y) + (x1y + (-1) .* x3y) .* (x2z + (-1) .* x4z)) .^ 2) .^ (-1 /  ...
  2) .* (((x1x + (-1) .* x3x) .* ((x1x + (-1) .* x3x) .^ 2 + (x1y +  ...
  (-1) .* x3y) .^ 2 + (x1z + (-1) .* x3z) .^ 2) .^ (-1 / 2) + (x2x + ...
   (-1) .* x4x) .* ((x2x + (-1) .* x4x) .^ 2 + (x2y + (-1) .* x4y)  ...
  .^ 2 + (x2z + (-1) .* x4z) .^ 2) .^ (-1 / 2)) .^ 2 + ((x1y + (-1)  ...
  .* x3y) .* ((x1x + (-1) .* x3x) .^ 2 + (x1y + (-1) .* x3y) .^ 2 +  ...
  (x1z + (-1) .* x3z) .^ 2) .^ (-1 / 2) + (x2y + (-1) .* x4y) .* (( ...
  x2x + (-1) .* x4x) .^ 2 + (x2y + (-1) .* x4y) .^ 2 + (x2z + (-1)  ...
  .* x4z) .^ 2) .^ (-1 / 2)) .^ 2 + (((x1x + (-1) .* x3x) .^ 2 + ( ...
  x1y + (-1) .* x3y) .^ 2 + (x1z + (-1) .* x3z) .^ 2) .^ (-1 / 2) .* ...
   (x1z + (-1) .* x3z) + ((x2x + (-1) .* x4x) .^ 2 + (x2y + (-1) .*  ...
  x4y) .^ 2 + (x2z + (-1) .* x4z) .^ 2) .^ (-1 / 2) .* (x2z + (-1)  ...
  .* x4z)) .^ 2) .^ (-3 / 2) .* (((-1) .* x1z + x3z) .* (x2y + (-1)  ...
  .* x4y) + (x1y + (-1) .* x3y) .* (x2z + (-1) .* x4z)) .* (2 .* (( ...
  -1) .* (x2y + (-1) .* x4y) .^ 2 .* ((x2x + (-1) .* x4x) .^ 2 + ( ...
  x2y + (-1) .* x4y) .^ 2 + (x2z + (-1) .* x4z) .^ 2) .^ (-3 / 2) +  ...
  ((x2x + (-1) .* x4x) .^ 2 + (x2y + (-1) .* x4y) .^ 2 + (x2z + (-1) ...
   .* x4z) .^ 2) .^ (-1 / 2)) .* ((x1y + (-1) .* x3y) .* ((x1x + ( ...
  -1) .* x3x) .^ 2 + (x1y + (-1) .* x3y) .^ 2 + (x1z + (-1) .* x3z)  ...
  .^ 2) .^ (-1 / 2) + (x2y + (-1) .* x4y) .* ((x2x + (-1) .* x4x)  ...
  .^ 2 + (x2y + (-1) .* x4y) .^ 2 + (x2z + (-1) .* x4z) .^ 2) .^ ( ...
  -1 / 2)) + (-2) .* (x2x + (-1) .* x4x) .* (x2y + (-1) .* x4y) .* ( ...
  (x1x + (-1) .* x3x) .* ((x1x + (-1) .* x3x) .^ 2 + (x1y + (-1) .*  ...
  x3y) .^ 2 + (x1z + (-1) .* x3z) .^ 2) .^ (-1 / 2) + (x2x + (-1) .* ...
   x4x) .* ((x2x + (-1) .* x4x) .^ 2 + (x2y + (-1) .* x4y) .^ 2 + ( ...
  x2z + (-1) .* x4z) .^ 2) .^ (-1 / 2)) .* ((x2x + (-1) .* x4x) .^  ...
  2 + (x2y + (-1) .* x4y) .^ 2 + (x2z + (-1) .* x4z) .^ 2) .^ (-3 /  ...
  2) + (-2) .* (x2y + (-1) .* x4y) .* (((x1x + (-1) .* x3x) .^ 2 + ( ...
  x1y + (-1) .* x3y) .^ 2 + (x1z + (-1) .* x3z) .^ 2) .^ (-1 / 2) .* ...
   (x1z + (-1) .* x3z) + ((x2x + (-1) .* x4x) .^ 2 + (x2y + (-1) .*  ...
  x4y) .^ 2 + (x2z + (-1) .* x4z) .^ 2) .^ (-1 / 2) .* (x2z + (-1)  ...
  .* x4z)) .* ((x2x + (-1) .* x4x) .^ 2 + (x2y + (-1) .* x4y) .^ 2 + ...
   (x2z + (-1) .* x4z) .^ 2) .^ (-3 / 2) .* (x2z + (-1) .* x4z)) .*  ...
  (((x1x + (-1) .* x3x) .^ 2 + (x1y + (-1) .* x3y) .^ 2 + (x1z + ( ...
  -1) .* x3z) .^ 2) .^ (-1 / 2) .* (x1z + (-1) .* x3z) + ((x2x + ( ...
  -1) .* x4x) .^ 2 + (x2y + (-1) .* x4y) .^ 2 + (x2z + (-1) .* x4z)  ...
  .^ 2) .^ (-1 / 2) .* (x2z + (-1) .* x4z)) + (-1) .* (x2x + (-1) .* ...
   x4x) .* (((-1) .* x1y + x3y) .* (x2x + (-1) .* x4x) + (x1x + (-1) ...
   .* x3x) .* (x2y + (-1) .* x4y)) .* (x2y + (-1) .* x4y) .* ((((-1) ...
   .* x1y + x3y) .* (x2x + (-1) .* x4x) + (x1x + (-1) .* x3x) .* ( ...
  x2y + (-1) .* x4y)) .^ 2 + ((x1z + (-1) .* x3z) .* (x2x + (-1) .*  ...
  x4x) + (-1) .* (x1x + (-1) .* x3x) .* (x2z + (-1) .* x4z)) .^ 2 +  ...
  (((-1) .* x1z + x3z) .* (x2y + (-1) .* x4y) + (x1y + (-1) .* x3y)  ...
  .* (x2z + (-1) .* x4z)) .^ 2) .^ (-1 / 2) .* (((x1x + (-1) .* x3x) ...
   .* ((x1x + (-1) .* x3x) .^ 2 + (x1y + (-1) .* x3y) .^ 2 + (x1z +  ...
  (-1) .* x3z) .^ 2) .^ (-1 / 2) + (x2x + (-1) .* x4x) .* ((x2x + ( ...
  -1) .* x4x) .^ 2 + (x2y + (-1) .* x4y) .^ 2 + (x2z + (-1) .* x4z)  ...
  .^ 2) .^ (-1 / 2)) .^ 2 + ((x1y + (-1) .* x3y) .* ((x1x + (-1) .*  ...
  x3x) .^ 2 + (x1y + (-1) .* x3y) .^ 2 + (x1z + (-1) .* x3z) .^ 2)  ...
  .^ (-1 / 2) + (x2y + (-1) .* x4y) .* ((x2x + (-1) .* x4x) .^ 2 + ( ...
  x2y + (-1) .* x4y) .^ 2 + (x2z + (-1) .* x4z) .^ 2) .^ (-1 / 2))  ...
  .^ 2 + (((x1x + (-1) .* x3x) .^ 2 + (x1y + (-1) .* x3y) .^ 2 + ( ...
  x1z + (-1) .* x3z) .^ 2) .^ (-1 / 2) .* (x1z + (-1) .* x3z) + (( ...
  x2x + (-1) .* x4x) .^ 2 + (x2y + (-1) .* x4y) .^ 2 + (x2z + (-1)  ...
  .* x4z) .^ 2) .^ (-1 / 2) .* (x2z + (-1) .* x4z)) .^ 2) .^ (-1 /  ...
  2) .* ((x2x + (-1) .* x4x) .^ 2 + (x2y + (-1) .* x4y) .^ 2 + (x2z  ...
  + (-1) .* x4z) .^ 2) .^ (-3 / 2) + (x2y + (-1) .* x4y) .* ((((-1)  ...
  .* x1y + x3y) .* (x2x + (-1) .* x4x) + (x1x + (-1) .* x3x) .* ( ...
  x2y + (-1) .* x4y)) .^ 2 + ((x1z + (-1) .* x3z) .* (x2x + (-1) .*  ...
  x4x) + (-1) .* (x1x + (-1) .* x3x) .* (x2z + (-1) .* x4z)) .^ 2 +  ...
  (((-1) .* x1z + x3z) .* (x2y + (-1) .* x4y) + (x1y + (-1) .* x3y)  ...
  .* (x2z + (-1) .* x4z)) .^ 2) .^ (-1 / 2) .* (((x1x + (-1) .* x3x) ...
   .* ((x1x + (-1) .* x3x) .^ 2 + (x1y + (-1) .* x3y) .^ 2 + (x1z +  ...
  (-1) .* x3z) .^ 2) .^ (-1 / 2) + (x2x + (-1) .* x4x) .* ((x2x + ( ...
  -1) .* x4x) .^ 2 + (x2y + (-1) .* x4y) .^ 2 + (x2z + (-1) .* x4z)  ...
  .^ 2) .^ (-1 / 2)) .^ 2 + ((x1y + (-1) .* x3y) .* ((x1x + (-1) .*  ...
  x3x) .^ 2 + (x1y + (-1) .* x3y) .^ 2 + (x1z + (-1) .* x3z) .^ 2)  ...
  .^ (-1 / 2) + (x2y + (-1) .* x4y) .* ((x2x + (-1) .* x4x) .^ 2 + ( ...
  x2y + (-1) .* x4y) .^ 2 + (x2z + (-1) .* x4z) .^ 2) .^ (-1 / 2))  ...
  .^ 2 + (((x1x + (-1) .* x3x) .^ 2 + (x1y + (-1) .* x3y) .^ 2 + ( ...
  x1z + (-1) .* x3z) .^ 2) .^ (-1 / 2) .* (x1z + (-1) .* x3z) + (( ...
  x2x + (-1) .* x4x) .^ 2 + (x2y + (-1) .* x4y) .^ 2 + (x2z + (-1)  ...
  .* x4z) .^ 2) .^ (-1 / 2) .* (x2z + (-1) .* x4z)) .^ 2) .^ (-1 /  ...
  2) .* (((-1) .* x1z + x3z) .* (x2y + (-1) .* x4y) + (x1y + (-1) .* ...
   x3y) .* (x2z + (-1) .* x4z)) .* ((x2x + (-1) .* x4x) .^ 2 + (x2y  ...
  + (-1) .* x4y) .^ 2 + (x2z + (-1) .* x4z) .^ 2) .^ (-3 / 2) .* ( ...
  x2z + (-1) .* x4z),(-1 / 2) .* (((-1) .* x1y + x3y) .* (x2x + (-1) ...
   .* x4x) + (x1x + (-1) .* x3x) .* (x2y + (-1) .* x4y)) .* (2 .* (( ...
  -1) .* x1x + x3x) .* ((x1z + (-1) .* x3z) .* (x2x + (-1) .* x4x) + ...
   (-1) .* (x1x + (-1) .* x3x) .* (x2z + (-1) .* x4z)) + 2 .* (x1y + ...
   (-1) .* x3y) .* (((-1) .* x1z + x3z) .* (x2y + (-1) .* x4y) + ( ...
  x1y + (-1) .* x3y) .* (x2z + (-1) .* x4z))) .* ((((-1) .* x1y +  ...
  x3y) .* (x2x + (-1) .* x4x) + (x1x + (-1) .* x3x) .* (x2y + (-1)  ...
  .* x4y)) .^ 2 + ((x1z + (-1) .* x3z) .* (x2x + (-1) .* x4x) + (-1) ...
   .* (x1x + (-1) .* x3x) .* (x2z + (-1) .* x4z)) .^ 2 + (((-1) .*  ...
  x1z + x3z) .* (x2y + (-1) .* x4y) + (x1y + (-1) .* x3y) .* (x2z +  ...
  (-1) .* x4z)) .^ 2) .^ (-3 / 2) .* (((x1x + (-1) .* x3x) .* ((x1x  ...
  + (-1) .* x3x) .^ 2 + (x1y + (-1) .* x3y) .^ 2 + (x1z + (-1) .*  ...
  x3z) .^ 2) .^ (-1 / 2) + (x2x + (-1) .* x4x) .* ((x2x + (-1) .*  ...
  x4x) .^ 2 + (x2y + (-1) .* x4y) .^ 2 + (x2z + (-1) .* x4z) .^ 2)  ...
  .^ (-1 / 2)) .^ 2 + ((x1y + (-1) .* x3y) .* ((x1x + (-1) .* x3x)  ...
  .^ 2 + (x1y + (-1) .* x3y) .^ 2 + (x1z + (-1) .* x3z) .^ 2) .^ ( ...
  -1 / 2) + (x2y + (-1) .* x4y) .* ((x2x + (-1) .* x4x) .^ 2 + (x2y  ...
  + (-1) .* x4y) .^ 2 + (x2z + (-1) .* x4z) .^ 2) .^ (-1 / 2)) .^ 2  ...
  + (((x1x + (-1) .* x3x) .^ 2 + (x1y + (-1) .* x3y) .^ 2 + (x1z + ( ...
  -1) .* x3z) .^ 2) .^ (-1 / 2) .* (x1z + (-1) .* x3z) + ((x2x + ( ...
  -1) .* x4x) .^ 2 + (x2y + (-1) .* x4y) .^ 2 + (x2z + (-1) .* x4z)  ...
  .^ 2) .^ (-1 / 2) .* (x2z + (-1) .* x4z)) .^ 2) .^ (-1 / 2) .* (( ...
  x1x + (-1) .* x3x) .* ((x1x + (-1) .* x3x) .^ 2 + (x1y + (-1) .*  ...
  x3y) .^ 2 + (x1z + (-1) .* x3z) .^ 2) .^ (-1 / 2) + (x2x + (-1) .* ...
   x4x) .* ((x2x + (-1) .* x4x) .^ 2 + (x2y + (-1) .* x4y) .^ 2 + ( ...
  x2z + (-1) .* x4z) .^ 2) .^ (-1 / 2)) + (-1 / 2) .* (((-1) .* x1y  ...
  + x3y) .* (x2x + (-1) .* x4x) + (x1x + (-1) .* x3x) .* (x2y + (-1) ...
   .* x4y)) .* ((((-1) .* x1y + x3y) .* (x2x + (-1) .* x4x) + (x1x + ...
   (-1) .* x3x) .* (x2y + (-1) .* x4y)) .^ 2 + ((x1z + (-1) .* x3z)  ...
  .* (x2x + (-1) .* x4x) + (-1) .* (x1x + (-1) .* x3x) .* (x2z + ( ...
  -1) .* x4z)) .^ 2 + (((-1) .* x1z + x3z) .* (x2y + (-1) .* x4y) +  ...
  (x1y + (-1) .* x3y) .* (x2z + (-1) .* x4z)) .^ 2) .^ (-1 / 2) .* ( ...
  ((x1x + (-1) .* x3x) .* ((x1x + (-1) .* x3x) .^ 2 + (x1y + (-1) .* ...
   x3y) .^ 2 + (x1z + (-1) .* x3z) .^ 2) .^ (-1 / 2) + (x2x + (-1)  ...
  .* x4x) .* ((x2x + (-1) .* x4x) .^ 2 + (x2y + (-1) .* x4y) .^ 2 +  ...
  (x2z + (-1) .* x4z) .^ 2) .^ (-1 / 2)) .^ 2 + ((x1y + (-1) .* x3y) ...
   .* ((x1x + (-1) .* x3x) .^ 2 + (x1y + (-1) .* x3y) .^ 2 + (x1z +  ...
  (-1) .* x3z) .^ 2) .^ (-1 / 2) + (x2y + (-1) .* x4y) .* ((x2x + ( ...
  -1) .* x4x) .^ 2 + (x2y + (-1) .* x4y) .^ 2 + (x2z + (-1) .* x4z)  ...
  .^ 2) .^ (-1 / 2)) .^ 2 + (((x1x + (-1) .* x3x) .^ 2 + (x1y + (-1) ...
   .* x3y) .^ 2 + (x1z + (-1) .* x3z) .^ 2) .^ (-1 / 2) .* (x1z + ( ...
  -1) .* x3z) + ((x2x + (-1) .* x4x) .^ 2 + (x2y + (-1) .* x4y) .^  ...
  2 + (x2z + (-1) .* x4z) .^ 2) .^ (-1 / 2) .* (x2z + (-1) .* x4z))  ...
  .^ 2) .^ (-3 / 2) .* ((x1x + (-1) .* x3x) .* ((x1x + (-1) .* x3x)  ...
  .^ 2 + (x1y + (-1) .* x3y) .^ 2 + (x1z + (-1) .* x3z) .^ 2) .^ ( ...
  -1 / 2) + (x2x + (-1) .* x4x) .* ((x2x + (-1) .* x4x) .^ 2 + (x2y  ...
  + (-1) .* x4y) .^ 2 + (x2z + (-1) .* x4z) .^ 2) .^ (-1 / 2)) .* ( ...
  2 .* (((x1x + (-1) .* x3x) .^ 2 + (x1y + (-1) .* x3y) .^ 2 + (x1z  ...
  + (-1) .* x3z) .^ 2) .^ (-1 / 2) .* (x1z + (-1) .* x3z) + ((x2x +  ...
  (-1) .* x4x) .^ 2 + (x2y + (-1) .* x4y) .^ 2 + (x2z + (-1) .* x4z) ...
   .^ 2) .^ (-1 / 2) .* (x2z + (-1) .* x4z)) .* (((x2x + (-1) .*  ...
  x4x) .^ 2 + (x2y + (-1) .* x4y) .^ 2 + (x2z + (-1) .* x4z) .^ 2)  ...
  .^ (-1 / 2) + (-1) .* ((x2x + (-1) .* x4x) .^ 2 + (x2y + (-1) .*  ...
  x4y) .^ 2 + (x2z + (-1) .* x4z) .^ 2) .^ (-3 / 2) .* (x2z + (-1)  ...
  .* x4z) .^ 2) + (-2) .* (x2x + (-1) .* x4x) .* ((x1x + (-1) .*  ...
  x3x) .* ((x1x + (-1) .* x3x) .^ 2 + (x1y + (-1) .* x3y) .^ 2 + ( ...
  x1z + (-1) .* x3z) .^ 2) .^ (-1 / 2) + (x2x + (-1) .* x4x) .* (( ...
  x2x + (-1) .* x4x) .^ 2 + (x2y + (-1) .* x4y) .^ 2 + (x2z + (-1)  ...
  .* x4z) .^ 2) .^ (-1 / 2)) .* ((x2x + (-1) .* x4x) .^ 2 + (x2y + ( ...
  -1) .* x4y) .^ 2 + (x2z + (-1) .* x4z) .^ 2) .^ (-3 / 2) .* (x2z + ...
   (-1) .* x4z) + (-2) .* (x2y + (-1) .* x4y) .* ((x1y + (-1) .*  ...
  x3y) .* ((x1x + (-1) .* x3x) .^ 2 + (x1y + (-1) .* x3y) .^ 2 + ( ...
  x1z + (-1) .* x3z) .^ 2) .^ (-1 / 2) + (x2y + (-1) .* x4y) .* (( ...
  x2x + (-1) .* x4x) .^ 2 + (x2y + (-1) .* x4y) .^ 2 + (x2z + (-1)  ...
  .* x4z) .^ 2) .^ (-1 / 2)) .* ((x2x + (-1) .* x4x) .^ 2 + (x2y + ( ...
  -1) .* x4y) .^ 2 + (x2z + (-1) .* x4z) .^ 2) .^ (-3 / 2) .* (x2z + ...
   (-1) .* x4z)) + (-1) .* (x1y + (-1) .* x3y) .* ((((-1) .* x1y +  ...
  x3y) .* (x2x + (-1) .* x4x) + (x1x + (-1) .* x3x) .* (x2y + (-1)  ...
  .* x4y)) .^ 2 + ((x1z + (-1) .* x3z) .* (x2x + (-1) .* x4x) + (-1) ...
   .* (x1x + (-1) .* x3x) .* (x2z + (-1) .* x4z)) .^ 2 + (((-1) .*  ...
  x1z + x3z) .* (x2y + (-1) .* x4y) + (x1y + (-1) .* x3y) .* (x2z +  ...
  (-1) .* x4z)) .^ 2) .^ (-1 / 2) .* (((x1x + (-1) .* x3x) .* ((x1x  ...
  + (-1) .* x3x) .^ 2 + (x1y + (-1) .* x3y) .^ 2 + (x1z + (-1) .*  ...
  x3z) .^ 2) .^ (-1 / 2) + (x2x + (-1) .* x4x) .* ((x2x + (-1) .*  ...
  x4x) .^ 2 + (x2y + (-1) .* x4y) .^ 2 + (x2z + (-1) .* x4z) .^ 2)  ...
  .^ (-1 / 2)) .^ 2 + ((x1y + (-1) .* x3y) .* ((x1x + (-1) .* x3x)  ...
  .^ 2 + (x1y + (-1) .* x3y) .^ 2 + (x1z + (-1) .* x3z) .^ 2) .^ ( ...
  -1 / 2) + (x2y + (-1) .* x4y) .* ((x2x + (-1) .* x4x) .^ 2 + (x2y  ...
  + (-1) .* x4y) .^ 2 + (x2z + (-1) .* x4z) .^ 2) .^ (-1 / 2)) .^ 2  ...
  + (((x1x + (-1) .* x3x) .^ 2 + (x1y + (-1) .* x3y) .^ 2 + (x1z + ( ...
  -1) .* x3z) .^ 2) .^ (-1 / 2) .* (x1z + (-1) .* x3z) + ((x2x + ( ...
  -1) .* x4x) .^ 2 + (x2y + (-1) .* x4y) .^ 2 + (x2z + (-1) .* x4z)  ...
  .^ 2) .^ (-1 / 2) .* (x2z + (-1) .* x4z)) .^ 2) .^ (-1 / 2) .* ((( ...
  x1x + (-1) .* x3x) .^ 2 + (x1y + (-1) .* x3y) .^ 2 + (x1z + (-1)  ...
  .* x3z) .^ 2) .^ (-1 / 2) .* (x1z + (-1) .* x3z) + ((x2x + (-1) .* ...
   x4x) .^ 2 + (x2y + (-1) .* x4y) .^ 2 + (x2z + (-1) .* x4z) .^ 2)  ...
  .^ (-1 / 2) .* (x2z + (-1) .* x4z)) + (1 / 2) .* (2 .* ((-1) .*  ...
  x1x + x3x) .* ((x1z + (-1) .* x3z) .* (x2x + (-1) .* x4x) + (-1)  ...
  .* (x1x + (-1) .* x3x) .* (x2z + (-1) .* x4z)) + 2 .* (x1y + (-1)  ...
  .* x3y) .* (((-1) .* x1z + x3z) .* (x2y + (-1) .* x4y) + (x1y + ( ...
  -1) .* x3y) .* (x2z + (-1) .* x4z))) .* ((((-1) .* x1y + x3y) .* ( ...
  x2x + (-1) .* x4x) + (x1x + (-1) .* x3x) .* (x2y + (-1) .* x4y))  ...
  .^ 2 + ((x1z + (-1) .* x3z) .* (x2x + (-1) .* x4x) + (-1) .* (x1x  ...
  + (-1) .* x3x) .* (x2z + (-1) .* x4z)) .^ 2 + (((-1) .* x1z + x3z) ...
   .* (x2y + (-1) .* x4y) + (x1y + (-1) .* x3y) .* (x2z + (-1) .*  ...
  x4z)) .^ 2) .^ (-3 / 2) .* (((x1x + (-1) .* x3x) .* ((x1x + (-1)  ...
  .* x3x) .^ 2 + (x1y + (-1) .* x3y) .^ 2 + (x1z + (-1) .* x3z) .^  ...
  2) .^ (-1 / 2) + (x2x + (-1) .* x4x) .* ((x2x + (-1) .* x4x) .^ 2  ...
  + (x2y + (-1) .* x4y) .^ 2 + (x2z + (-1) .* x4z) .^ 2) .^ (-1 / 2) ...
  ) .^ 2 + ((x1y + (-1) .* x3y) .* ((x1x + (-1) .* x3x) .^ 2 + (x1y  ...
  + (-1) .* x3y) .^ 2 + (x1z + (-1) .* x3z) .^ 2) .^ (-1 / 2) + ( ...
  x2y + (-1) .* x4y) .* ((x2x + (-1) .* x4x) .^ 2 + (x2y + (-1) .*  ...
  x4y) .^ 2 + (x2z + (-1) .* x4z) .^ 2) .^ (-1 / 2)) .^ 2 + (((x1x + ...
   (-1) .* x3x) .^ 2 + (x1y + (-1) .* x3y) .^ 2 + (x1z + (-1) .*  ...
  x3z) .^ 2) .^ (-1 / 2) .* (x1z + (-1) .* x3z) + ((x2x + (-1) .*  ...
  x4x) .^ 2 + (x2y + (-1) .* x4y) .^ 2 + (x2z + (-1) .* x4z) .^ 2)  ...
  .^ (-1 / 2) .* (x2z + (-1) .* x4z)) .^ 2) .^ (-1 / 2) .* (((-1) .* ...
   x1z + x3z) .* (x2y + (-1) .* x4y) + (x1y + (-1) .* x3y) .* (x2z + ...
   (-1) .* x4z)) .* (((x1x + (-1) .* x3x) .^ 2 + (x1y + (-1) .* x3y) ...
   .^ 2 + (x1z + (-1) .* x3z) .^ 2) .^ (-1 / 2) .* (x1z + (-1) .*  ...
  x3z) + ((x2x + (-1) .* x4x) .^ 2 + (x2y + (-1) .* x4y) .^ 2 + ( ...
  x2z + (-1) .* x4z) .^ 2) .^ (-1 / 2) .* (x2z + (-1) .* x4z)) + (1  ...
  / 2) .* ((((-1) .* x1y + x3y) .* (x2x + (-1) .* x4x) + (x1x + (-1) ...
   .* x3x) .* (x2y + (-1) .* x4y)) .^ 2 + ((x1z + (-1) .* x3z) .* ( ...
  x2x + (-1) .* x4x) + (-1) .* (x1x + (-1) .* x3x) .* (x2z + (-1) .* ...
   x4z)) .^ 2 + (((-1) .* x1z + x3z) .* (x2y + (-1) .* x4y) + (x1y + ...
   (-1) .* x3y) .* (x2z + (-1) .* x4z)) .^ 2) .^ (-1 / 2) .* (((x1x  ...
  + (-1) .* x3x) .* ((x1x + (-1) .* x3x) .^ 2 + (x1y + (-1) .* x3y)  ...
  .^ 2 + (x1z + (-1) .* x3z) .^ 2) .^ (-1 / 2) + (x2x + (-1) .* x4x) ...
   .* ((x2x + (-1) .* x4x) .^ 2 + (x2y + (-1) .* x4y) .^ 2 + (x2z +  ...
  (-1) .* x4z) .^ 2) .^ (-1 / 2)) .^ 2 + ((x1y + (-1) .* x3y) .* (( ...
  x1x + (-1) .* x3x) .^ 2 + (x1y + (-1) .* x3y) .^ 2 + (x1z + (-1)  ...
  .* x3z) .^ 2) .^ (-1 / 2) + (x2y + (-1) .* x4y) .* ((x2x + (-1) .* ...
   x4x) .^ 2 + (x2y + (-1) .* x4y) .^ 2 + (x2z + (-1) .* x4z) .^ 2)  ...
  .^ (-1 / 2)) .^ 2 + (((x1x + (-1) .* x3x) .^ 2 + (x1y + (-1) .*  ...
  x3y) .^ 2 + (x1z + (-1) .* x3z) .^ 2) .^ (-1 / 2) .* (x1z + (-1)  ...
  .* x3z) + ((x2x + (-1) .* x4x) .^ 2 + (x2y + (-1) .* x4y) .^ 2 + ( ...
  x2z + (-1) .* x4z) .^ 2) .^ (-1 / 2) .* (x2z + (-1) .* x4z)) .^ 2) ...
   .^ (-3 / 2) .* (((-1) .* x1z + x3z) .* (x2y + (-1) .* x4y) + ( ...
  x1y + (-1) .* x3y) .* (x2z + (-1) .* x4z)) .* (2 .* (((x1x + (-1)  ...
  .* x3x) .^ 2 + (x1y + (-1) .* x3y) .^ 2 + (x1z + (-1) .* x3z) .^  ...
  2) .^ (-1 / 2) .* (x1z + (-1) .* x3z) + ((x2x + (-1) .* x4x) .^ 2  ...
  + (x2y + (-1) .* x4y) .^ 2 + (x2z + (-1) .* x4z) .^ 2) .^ (-1 / 2) ...
   .* (x2z + (-1) .* x4z)) .* (((x2x + (-1) .* x4x) .^ 2 + (x2y + ( ...
  -1) .* x4y) .^ 2 + (x2z + (-1) .* x4z) .^ 2) .^ (-1 / 2) + (-1) .* ...
   ((x2x + (-1) .* x4x) .^ 2 + (x2y + (-1) .* x4y) .^ 2 + (x2z + ( ...
  -1) .* x4z) .^ 2) .^ (-3 / 2) .* (x2z + (-1) .* x4z) .^ 2) + (-2)  ...
  .* (x2x + (-1) .* x4x) .* ((x1x + (-1) .* x3x) .* ((x1x + (-1) .*  ...
  x3x) .^ 2 + (x1y + (-1) .* x3y) .^ 2 + (x1z + (-1) .* x3z) .^ 2)  ...
  .^ (-1 / 2) + (x2x + (-1) .* x4x) .* ((x2x + (-1) .* x4x) .^ 2 + ( ...
  x2y + (-1) .* x4y) .^ 2 + (x2z + (-1) .* x4z) .^ 2) .^ (-1 / 2))  ...
  .* ((x2x + (-1) .* x4x) .^ 2 + (x2y + (-1) .* x4y) .^ 2 + (x2z + ( ...
  -1) .* x4z) .^ 2) .^ (-3 / 2) .* (x2z + (-1) .* x4z) + (-2) .* ( ...
  x2y + (-1) .* x4y) .* ((x1y + (-1) .* x3y) .* ((x1x + (-1) .* x3x) ...
   .^ 2 + (x1y + (-1) .* x3y) .^ 2 + (x1z + (-1) .* x3z) .^ 2) .^ ( ...
  -1 / 2) + (x2y + (-1) .* x4y) .* ((x2x + (-1) .* x4x) .^ 2 + (x2y  ...
  + (-1) .* x4y) .^ 2 + (x2z + (-1) .* x4z) .^ 2) .^ (-1 / 2)) .* (( ...
  x2x + (-1) .* x4x) .^ 2 + (x2y + (-1) .* x4y) .^ 2 + (x2z + (-1)  ...
  .* x4z) .^ 2) .^ (-3 / 2) .* (x2z + (-1) .* x4z)) .* (((x1x + (-1) ...
   .* x3x) .^ 2 + (x1y + (-1) .* x3y) .^ 2 + (x1z + (-1) .* x3z) .^  ...
  2) .^ (-1 / 2) .* (x1z + (-1) .* x3z) + ((x2x + (-1) .* x4x) .^ 2  ...
  + (x2y + (-1) .* x4y) .^ 2 + (x2z + (-1) .* x4z) .^ 2) .^ (-1 / 2) ...
   .* (x2z + (-1) .* x4z)) + (-1) .* ((((-1) .* x1y + x3y) .* (x2x + ...
   (-1) .* x4x) + (x1x + (-1) .* x3x) .* (x2y + (-1) .* x4y)) .^ 2 + ...
   ((x1z + (-1) .* x3z) .* (x2x + (-1) .* x4x) + (-1) .* (x1x + (-1) ...
   .* x3x) .* (x2z + (-1) .* x4z)) .^ 2 + (((-1) .* x1z + x3z) .* ( ...
  x2y + (-1) .* x4y) + (x1y + (-1) .* x3y) .* (x2z + (-1) .* x4z))  ...
  .^ 2) .^ (-1 / 2) .* (((x1x + (-1) .* x3x) .* ((x1x + (-1) .* x3x) ...
   .^ 2 + (x1y + (-1) .* x3y) .^ 2 + (x1z + (-1) .* x3z) .^ 2) .^ ( ...
  -1 / 2) + (x2x + (-1) .* x4x) .* ((x2x + (-1) .* x4x) .^ 2 + (x2y  ...
  + (-1) .* x4y) .^ 2 + (x2z + (-1) .* x4z) .^ 2) .^ (-1 / 2)) .^ 2  ...
  + ((x1y + (-1) .* x3y) .* ((x1x + (-1) .* x3x) .^ 2 + (x1y + (-1)  ...
  .* x3y) .^ 2 + (x1z + (-1) .* x3z) .^ 2) .^ (-1 / 2) + (x2y + (-1) ...
   .* x4y) .* ((x2x + (-1) .* x4x) .^ 2 + (x2y + (-1) .* x4y) .^ 2 + ...
   (x2z + (-1) .* x4z) .^ 2) .^ (-1 / 2)) .^ 2 + (((x1x + (-1) .*  ...
  x3x) .^ 2 + (x1y + (-1) .* x3y) .^ 2 + (x1z + (-1) .* x3z) .^ 2)  ...
  .^ (-1 / 2) .* (x1z + (-1) .* x3z) + ((x2x + (-1) .* x4x) .^ 2 + ( ...
  x2y + (-1) .* x4y) .^ 2 + (x2z + (-1) .* x4z) .^ 2) .^ (-1 / 2) .* ...
   (x2z + (-1) .* x4z)) .^ 2) .^ (-1 / 2) .* (((-1) .* x1z + x3z) .* ...
   (x2y + (-1) .* x4y) + (x1y + (-1) .* x3y) .* (x2z + (-1) .* x4z)) ...
   .* (((x2x + (-1) .* x4x) .^ 2 + (x2y + (-1) .* x4y) .^ 2 + (x2z + ...
   (-1) .* x4z) .^ 2) .^ (-1 / 2) + (-1) .* ((x2x + (-1) .* x4x) .^  ...
  2 + (x2y + (-1) .* x4y) .^ 2 + (x2z + (-1) .* x4z) .^ 2) .^ (-3 /  ...
  2) .* (x2z + (-1) .* x4z) .^ 2) + (-1) .* (x2x + (-1) .* x4x) .* ( ...
  ((-1) .* x1y + x3y) .* (x2x + (-1) .* x4x) + (x1x + (-1) .* x3x)  ...
  .* (x2y + (-1) .* x4y)) .* ((((-1) .* x1y + x3y) .* (x2x + (-1) .* ...
   x4x) + (x1x + (-1) .* x3x) .* (x2y + (-1) .* x4y)) .^ 2 + ((x1z + ...
   (-1) .* x3z) .* (x2x + (-1) .* x4x) + (-1) .* (x1x + (-1) .* x3x) ...
   .* (x2z + (-1) .* x4z)) .^ 2 + (((-1) .* x1z + x3z) .* (x2y + ( ...
  -1) .* x4y) + (x1y + (-1) .* x3y) .* (x2z + (-1) .* x4z)) .^ 2)  ...
  .^ (-1 / 2) .* (((x1x + (-1) .* x3x) .* ((x1x + (-1) .* x3x) .^ 2  ...
  + (x1y + (-1) .* x3y) .^ 2 + (x1z + (-1) .* x3z) .^ 2) .^ (-1 / 2) ...
   + (x2x + (-1) .* x4x) .* ((x2x + (-1) .* x4x) .^ 2 + (x2y + (-1)  ...
  .* x4y) .^ 2 + (x2z + (-1) .* x4z) .^ 2) .^ (-1 / 2)) .^ 2 + (( ...
  x1y + (-1) .* x3y) .* ((x1x + (-1) .* x3x) .^ 2 + (x1y + (-1) .*  ...
  x3y) .^ 2 + (x1z + (-1) .* x3z) .^ 2) .^ (-1 / 2) + (x2y + (-1) .* ...
   x4y) .* ((x2x + (-1) .* x4x) .^ 2 + (x2y + (-1) .* x4y) .^ 2 + ( ...
  x2z + (-1) .* x4z) .^ 2) .^ (-1 / 2)) .^ 2 + (((x1x + (-1) .* x3x) ...
   .^ 2 + (x1y + (-1) .* x3y) .^ 2 + (x1z + (-1) .* x3z) .^ 2) .^ ( ...
  -1 / 2) .* (x1z + (-1) .* x3z) + ((x2x + (-1) .* x4x) .^ 2 + (x2y  ...
  + (-1) .* x4y) .^ 2 + (x2z + (-1) .* x4z) .^ 2) .^ (-1 / 2) .* ( ...
  x2z + (-1) .* x4z)) .^ 2) .^ (-1 / 2) .* ((x2x + (-1) .* x4x) .^  ...
  2 + (x2y + (-1) .* x4y) .^ 2 + (x2z + (-1) .* x4z) .^ 2) .^ (-3 /  ...
  2) .* (x2z + (-1) .* x4z),((x1x + (-1) .* x3x) .^ 2 .* ((x1x + ( ...
  -1) .* x3x) .^ 2 + (x1y + (-1) .* x3y) .^ 2 + (x1z + (-1) .* x3z)  ...
  .^ 2) .^ (-3 / 2) + (-1) .* ((x1x + (-1) .* x3x) .^ 2 + (x1y + ( ...
  -1) .* x3y) .^ 2 + (x1z + (-1) .* x3z) .^ 2) .^ (-1 / 2)) .* ((( ...
  -1) .* x1y + x3y) .* (x2x + (-1) .* x4x) + (x1x + (-1) .* x3x) .*  ...
  (x2y + (-1) .* x4y)) .* ((((-1) .* x1y + x3y) .* (x2x + (-1) .*  ...
  x4x) + (x1x + (-1) .* x3x) .* (x2y + (-1) .* x4y)) .^ 2 + ((x1z +  ...
  (-1) .* x3z) .* (x2x + (-1) .* x4x) + (-1) .* (x1x + (-1) .* x3x)  ...
  .* (x2z + (-1) .* x4z)) .^ 2 + (((-1) .* x1z + x3z) .* (x2y + (-1) ...
   .* x4y) + (x1y + (-1) .* x3y) .* (x2z + (-1) .* x4z)) .^ 2) .^ ( ...
  -1 / 2) .* (((x1x + (-1) .* x3x) .* ((x1x + (-1) .* x3x) .^ 2 + ( ...
  x1y + (-1) .* x3y) .^ 2 + (x1z + (-1) .* x3z) .^ 2) .^ (-1 / 2) +  ...
  (x2x + (-1) .* x4x) .* ((x2x + (-1) .* x4x) .^ 2 + (x2y + (-1) .*  ...
  x4y) .^ 2 + (x2z + (-1) .* x4z) .^ 2) .^ (-1 / 2)) .^ 2 + ((x1y +  ...
  (-1) .* x3y) .* ((x1x + (-1) .* x3x) .^ 2 + (x1y + (-1) .* x3y)  ...
  .^ 2 + (x1z + (-1) .* x3z) .^ 2) .^ (-1 / 2) + (x2y + (-1) .* x4y) ...
   .* ((x2x + (-1) .* x4x) .^ 2 + (x2y + (-1) .* x4y) .^ 2 + (x2z +  ...
  (-1) .* x4z) .^ 2) .^ (-1 / 2)) .^ 2 + (((x1x + (-1) .* x3x) .^ 2  ...
  + (x1y + (-1) .* x3y) .^ 2 + (x1z + (-1) .* x3z) .^ 2) .^ (-1 / 2) ...
   .* (x1z + (-1) .* x3z) + ((x2x + (-1) .* x4x) .^ 2 + (x2y + (-1)  ...
  .* x4y) .^ 2 + (x2z + (-1) .* x4z) .^ 2) .^ (-1 / 2) .* (x2z + ( ...
  -1) .* x4z)) .^ 2) .^ (-1 / 2) + (-1 / 2) .* (((-1) .* x1y + x3y)  ...
  .* (x2x + (-1) .* x4x) + (x1x + (-1) .* x3x) .* (x2y + (-1) .*  ...
  x4y)) .* ((((-1) .* x1y + x3y) .* (x2x + (-1) .* x4x) + (x1x + ( ...
  -1) .* x3x) .* (x2y + (-1) .* x4y)) .^ 2 + ((x1z + (-1) .* x3z) .* ...
   (x2x + (-1) .* x4x) + (-1) .* (x1x + (-1) .* x3x) .* (x2z + (-1)  ...
  .* x4z)) .^ 2 + (((-1) .* x1z + x3z) .* (x2y + (-1) .* x4y) + ( ...
  x1y + (-1) .* x3y) .* (x2z + (-1) .* x4z)) .^ 2) .^ (-1 / 2) .* ( ...
  2 .* ((x1x + (-1) .* x3x) .^ 2 .* ((x1x + (-1) .* x3x) .^ 2 + ( ...
  x1y + (-1) .* x3y) .^ 2 + (x1z + (-1) .* x3z) .^ 2) .^ (-3 / 2) +  ...
  (-1) .* ((x1x + (-1) .* x3x) .^ 2 + (x1y + (-1) .* x3y) .^ 2 + ( ...
  x1z + (-1) .* x3z) .^ 2) .^ (-1 / 2)) .* ((x1x + (-1) .* x3x) .* ( ...
  (x1x + (-1) .* x3x) .^ 2 + (x1y + (-1) .* x3y) .^ 2 + (x1z + (-1)  ...
  .* x3z) .^ 2) .^ (-1 / 2) + (x2x + (-1) .* x4x) .* ((x2x + (-1) .* ...
   x4x) .^ 2 + (x2y + (-1) .* x4y) .^ 2 + (x2z + (-1) .* x4z) .^ 2)  ...
  .^ (-1 / 2)) + 2 .* (x1x + (-1) .* x3x) .* (x1y + (-1) .* x3y) .*  ...
  ((x1x + (-1) .* x3x) .^ 2 + (x1y + (-1) .* x3y) .^ 2 + (x1z + (-1) ...
   .* x3z) .^ 2) .^ (-3 / 2) .* ((x1y + (-1) .* x3y) .* ((x1x + (-1) ...
   .* x3x) .^ 2 + (x1y + (-1) .* x3y) .^ 2 + (x1z + (-1) .* x3z) .^  ...
  2) .^ (-1 / 2) + (x2y + (-1) .* x4y) .* ((x2x + (-1) .* x4x) .^ 2  ...
  + (x2y + (-1) .* x4y) .^ 2 + (x2z + (-1) .* x4z) .^ 2) .^ (-1 / 2) ...
  ) + 2 .* (x1x + (-1) .* x3x) .* ((x1x + (-1) .* x3x) .^ 2 + (x1y + ...
   (-1) .* x3y) .^ 2 + (x1z + (-1) .* x3z) .^ 2) .^ (-3 / 2) .* ( ...
  x1z + (-1) .* x3z) .* (((x1x + (-1) .* x3x) .^ 2 + (x1y + (-1) .*  ...
  x3y) .^ 2 + (x1z + (-1) .* x3z) .^ 2) .^ (-1 / 2) .* (x1z + (-1)  ...
  .* x3z) + ((x2x + (-1) .* x4x) .^ 2 + (x2y + (-1) .* x4y) .^ 2 + ( ...
  x2z + (-1) .* x4z) .^ 2) .^ (-1 / 2) .* (x2z + (-1) .* x4z))) .* ( ...
  ((x1x + (-1) .* x3x) .* ((x1x + (-1) .* x3x) .^ 2 + (x1y + (-1) .* ...
   x3y) .^ 2 + (x1z + (-1) .* x3z) .^ 2) .^ (-1 / 2) + (x2x + (-1)  ...
  .* x4x) .* ((x2x + (-1) .* x4x) .^ 2 + (x2y + (-1) .* x4y) .^ 2 +  ...
  (x2z + (-1) .* x4z) .^ 2) .^ (-1 / 2)) .^ 2 + ((x1y + (-1) .* x3y) ...
   .* ((x1x + (-1) .* x3x) .^ 2 + (x1y + (-1) .* x3y) .^ 2 + (x1z +  ...
  (-1) .* x3z) .^ 2) .^ (-1 / 2) + (x2y + (-1) .* x4y) .* ((x2x + ( ...
  -1) .* x4x) .^ 2 + (x2y + (-1) .* x4y) .^ 2 + (x2z + (-1) .* x4z)  ...
  .^ 2) .^ (-1 / 2)) .^ 2 + (((x1x + (-1) .* x3x) .^ 2 + (x1y + (-1) ...
   .* x3y) .^ 2 + (x1z + (-1) .* x3z) .^ 2) .^ (-1 / 2) .* (x1z + ( ...
  -1) .* x3z) + ((x2x + (-1) .* x4x) .^ 2 + (x2y + (-1) .* x4y) .^  ...
  2 + (x2z + (-1) .* x4z) .^ 2) .^ (-1 / 2) .* (x2z + (-1) .* x4z))  ...
  .^ 2) .^ (-3 / 2) .* ((x1x + (-1) .* x3x) .* ((x1x + (-1) .* x3x)  ...
  .^ 2 + (x1y + (-1) .* x3y) .^ 2 + (x1z + (-1) .* x3z) .^ 2) .^ ( ...
  -1 / 2) + (x2x + (-1) .* x4x) .* ((x2x + (-1) .* x4x) .^ 2 + (x2y  ...
  + (-1) .* x4y) .^ 2 + (x2z + (-1) .* x4z) .^ 2) .^ (-1 / 2)) + (( ...
  -1) .* x2y + x4y) .* ((((-1) .* x1y + x3y) .* (x2x + (-1) .* x4x)  ...
  + (x1x + (-1) .* x3x) .* (x2y + (-1) .* x4y)) .^ 2 + ((x1z + (-1)  ...
  .* x3z) .* (x2x + (-1) .* x4x) + (-1) .* (x1x + (-1) .* x3x) .* ( ...
  x2z + (-1) .* x4z)) .^ 2 + (((-1) .* x1z + x3z) .* (x2y + (-1) .*  ...
  x4y) + (x1y + (-1) .* x3y) .* (x2z + (-1) .* x4z)) .^ 2) .^ (-1 /  ...
  2) .* (((x1x + (-1) .* x3x) .* ((x1x + (-1) .* x3x) .^ 2 + (x1y +  ...
  (-1) .* x3y) .^ 2 + (x1z + (-1) .* x3z) .^ 2) .^ (-1 / 2) + (x2x + ...
   (-1) .* x4x) .* ((x2x + (-1) .* x4x) .^ 2 + (x2y + (-1) .* x4y)  ...
  .^ 2 + (x2z + (-1) .* x4z) .^ 2) .^ (-1 / 2)) .^ 2 + ((x1y + (-1)  ...
  .* x3y) .* ((x1x + (-1) .* x3x) .^ 2 + (x1y + (-1) .* x3y) .^ 2 +  ...
  (x1z + (-1) .* x3z) .^ 2) .^ (-1 / 2) + (x2y + (-1) .* x4y) .* (( ...
  x2x + (-1) .* x4x) .^ 2 + (x2y + (-1) .* x4y) .^ 2 + (x2z + (-1)  ...
  .* x4z) .^ 2) .^ (-1 / 2)) .^ 2 + (((x1x + (-1) .* x3x) .^ 2 + ( ...
  x1y + (-1) .* x3y) .^ 2 + (x1z + (-1) .* x3z) .^ 2) .^ (-1 / 2) .* ...
   (x1z + (-1) .* x3z) + ((x2x + (-1) .* x4x) .^ 2 + (x2y + (-1) .*  ...
  x4y) .^ 2 + (x2z + (-1) .* x4z) .^ 2) .^ (-1 / 2) .* (x2z + (-1)  ...
  .* x4z)) .^ 2) .^ (-1 / 2) .* ((x1x + (-1) .* x3x) .* ((x1x + (-1) ...
   .* x3x) .^ 2 + (x1y + (-1) .* x3y) .^ 2 + (x1z + (-1) .* x3z) .^  ...
  2) .^ (-1 / 2) + (x2x + (-1) .* x4x) .* ((x2x + (-1) .* x4x) .^ 2  ...
  + (x2y + (-1) .* x4y) .^ 2 + (x2z + (-1) .* x4z) .^ 2) .^ (-1 / 2) ...
  ) + (-1) .* (x1x + (-1) .* x3x) .* ((x1x + (-1) .* x3x) .^ 2 + ( ...
  x1y + (-1) .* x3y) .^ 2 + (x1z + (-1) .* x3z) .^ 2) .^ (-3 / 2) .* ...
   (x1z + (-1) .* x3z) .* ((((-1) .* x1y + x3y) .* (x2x + (-1) .*  ...
  x4x) + (x1x + (-1) .* x3x) .* (x2y + (-1) .* x4y)) .^ 2 + ((x1z +  ...
  (-1) .* x3z) .* (x2x + (-1) .* x4x) + (-1) .* (x1x + (-1) .* x3x)  ...
  .* (x2z + (-1) .* x4z)) .^ 2 + (((-1) .* x1z + x3z) .* (x2y + (-1) ...
   .* x4y) + (x1y + (-1) .* x3y) .* (x2z + (-1) .* x4z)) .^ 2) .^ ( ...
  -1 / 2) .* (((x1x + (-1) .* x3x) .* ((x1x + (-1) .* x3x) .^ 2 + ( ...
  x1y + (-1) .* x3y) .^ 2 + (x1z + (-1) .* x3z) .^ 2) .^ (-1 / 2) +  ...
  (x2x + (-1) .* x4x) .* ((x2x + (-1) .* x4x) .^ 2 + (x2y + (-1) .*  ...
  x4y) .^ 2 + (x2z + (-1) .* x4z) .^ 2) .^ (-1 / 2)) .^ 2 + ((x1y +  ...
  (-1) .* x3y) .* ((x1x + (-1) .* x3x) .^ 2 + (x1y + (-1) .* x3y)  ...
  .^ 2 + (x1z + (-1) .* x3z) .^ 2) .^ (-1 / 2) + (x2y + (-1) .* x4y) ...
   .* ((x2x + (-1) .* x4x) .^ 2 + (x2y + (-1) .* x4y) .^ 2 + (x2z +  ...
  (-1) .* x4z) .^ 2) .^ (-1 / 2)) .^ 2 + (((x1x + (-1) .* x3x) .^ 2  ...
  + (x1y + (-1) .* x3y) .^ 2 + (x1z + (-1) .* x3z) .^ 2) .^ (-1 / 2) ...
   .* (x1z + (-1) .* x3z) + ((x2x + (-1) .* x4x) .^ 2 + (x2y + (-1)  ...
  .* x4y) .^ 2 + (x2z + (-1) .* x4z) .^ 2) .^ (-1 / 2) .* (x2z + ( ...
  -1) .* x4z)) .^ 2) .^ (-1 / 2) .* (((-1) .* x1z + x3z) .* (x2y + ( ...
  -1) .* x4y) + (x1y + (-1) .* x3y) .* (x2z + (-1) .* x4z)) + (-1 /  ...
  2) .* (((-1) .* x1y + x3y) .* (x2x + (-1) .* x4x) + (x1x + (-1) .* ...
   x3x) .* (x2y + (-1) .* x4y)) .* ((((-1) .* x1y + x3y) .* (x2x + ( ...
  -1) .* x4x) + (x1x + (-1) .* x3x) .* (x2y + (-1) .* x4y)) .^ 2 + ( ...
  (x1z + (-1) .* x3z) .* (x2x + (-1) .* x4x) + (-1) .* (x1x + (-1)  ...
  .* x3x) .* (x2z + (-1) .* x4z)) .^ 2 + (((-1) .* x1z + x3z) .* ( ...
  x2y + (-1) .* x4y) + (x1y + (-1) .* x3y) .* (x2z + (-1) .* x4z))  ...
  .^ 2) .^ (-3 / 2) .* (((x1x + (-1) .* x3x) .* ((x1x + (-1) .* x3x) ...
   .^ 2 + (x1y + (-1) .* x3y) .^ 2 + (x1z + (-1) .* x3z) .^ 2) .^ ( ...
  -1 / 2) + (x2x + (-1) .* x4x) .* ((x2x + (-1) .* x4x) .^ 2 + (x2y  ...
  + (-1) .* x4y) .^ 2 + (x2z + (-1) .* x4z) .^ 2) .^ (-1 / 2)) .^ 2  ...
  + ((x1y + (-1) .* x3y) .* ((x1x + (-1) .* x3x) .^ 2 + (x1y + (-1)  ...
  .* x3y) .^ 2 + (x1z + (-1) .* x3z) .^ 2) .^ (-1 / 2) + (x2y + (-1) ...
   .* x4y) .* ((x2x + (-1) .* x4x) .^ 2 + (x2y + (-1) .* x4y) .^ 2 + ...
   (x2z + (-1) .* x4z) .^ 2) .^ (-1 / 2)) .^ 2 + (((x1x + (-1) .*  ...
  x3x) .^ 2 + (x1y + (-1) .* x3y) .^ 2 + (x1z + (-1) .* x3z) .^ 2)  ...
  .^ (-1 / 2) .* (x1z + (-1) .* x3z) + ((x2x + (-1) .* x4x) .^ 2 + ( ...
  x2y + (-1) .* x4y) .^ 2 + (x2z + (-1) .* x4z) .^ 2) .^ (-1 / 2) .* ...
   (x2z + (-1) .* x4z)) .^ 2) .^ (-1 / 2) .* ((x1x + (-1) .* x3x) .* ...
   ((x1x + (-1) .* x3x) .^ 2 + (x1y + (-1) .* x3y) .^ 2 + (x1z + ( ...
  -1) .* x3z) .^ 2) .^ (-1 / 2) + (x2x + (-1) .* x4x) .* ((x2x + ( ...
  -1) .* x4x) .^ 2 + (x2y + (-1) .* x4y) .^ 2 + (x2z + (-1) .* x4z)  ...
  .^ 2) .^ (-1 / 2)) .* (2 .* (((-1) .* x1y + x3y) .* (x2x + (-1) .* ...
   x4x) + (x1x + (-1) .* x3x) .* (x2y + (-1) .* x4y)) .* ((-1) .*  ...
  x2y + x4y) + 2 .* ((x1z + (-1) .* x3z) .* (x2x + (-1) .* x4x) + ( ...
  -1) .* (x1x + (-1) .* x3x) .* (x2z + (-1) .* x4z)) .* (x2z + (-1)  ...
  .* x4z)) + (1 / 2) .* ((((-1) .* x1y + x3y) .* (x2x + (-1) .* x4x) ...
   + (x1x + (-1) .* x3x) .* (x2y + (-1) .* x4y)) .^ 2 + ((x1z + (-1) ...
   .* x3z) .* (x2x + (-1) .* x4x) + (-1) .* (x1x + (-1) .* x3x) .* ( ...
  x2z + (-1) .* x4z)) .^ 2 + (((-1) .* x1z + x3z) .* (x2y + (-1) .*  ...
  x4y) + (x1y + (-1) .* x3y) .* (x2z + (-1) .* x4z)) .^ 2) .^ (-1 /  ...
  2) .* (2 .* ((x1x + (-1) .* x3x) .^ 2 .* ((x1x + (-1) .* x3x) .^  ...
  2 + (x1y + (-1) .* x3y) .^ 2 + (x1z + (-1) .* x3z) .^ 2) .^ (-3 /  ...
  2) + (-1) .* ((x1x + (-1) .* x3x) .^ 2 + (x1y + (-1) .* x3y) .^ 2  ...
  + (x1z + (-1) .* x3z) .^ 2) .^ (-1 / 2)) .* ((x1x + (-1) .* x3x)  ...
  .* ((x1x + (-1) .* x3x) .^ 2 + (x1y + (-1) .* x3y) .^ 2 + (x1z + ( ...
  -1) .* x3z) .^ 2) .^ (-1 / 2) + (x2x + (-1) .* x4x) .* ((x2x + ( ...
  -1) .* x4x) .^ 2 + (x2y + (-1) .* x4y) .^ 2 + (x2z + (-1) .* x4z)  ...
  .^ 2) .^ (-1 / 2)) + 2 .* (x1x + (-1) .* x3x) .* (x1y + (-1) .*  ...
  x3y) .* ((x1x + (-1) .* x3x) .^ 2 + (x1y + (-1) .* x3y) .^ 2 + ( ...
  x1z + (-1) .* x3z) .^ 2) .^ (-3 / 2) .* ((x1y + (-1) .* x3y) .* (( ...
  x1x + (-1) .* x3x) .^ 2 + (x1y + (-1) .* x3y) .^ 2 + (x1z + (-1)  ...
  .* x3z) .^ 2) .^ (-1 / 2) + (x2y + (-1) .* x4y) .* ((x2x + (-1) .* ...
   x4x) .^ 2 + (x2y + (-1) .* x4y) .^ 2 + (x2z + (-1) .* x4z) .^ 2)  ...
  .^ (-1 / 2)) + 2 .* (x1x + (-1) .* x3x) .* ((x1x + (-1) .* x3x)  ...
  .^ 2 + (x1y + (-1) .* x3y) .^ 2 + (x1z + (-1) .* x3z) .^ 2) .^ ( ...
  -3 / 2) .* (x1z + (-1) .* x3z) .* (((x1x + (-1) .* x3x) .^ 2 + ( ...
  x1y + (-1) .* x3y) .^ 2 + (x1z + (-1) .* x3z) .^ 2) .^ (-1 / 2) .* ...
   (x1z + (-1) .* x3z) + ((x2x + (-1) .* x4x) .^ 2 + (x2y + (-1) .*  ...
  x4y) .^ 2 + (x2z + (-1) .* x4z) .^ 2) .^ (-1 / 2) .* (x2z + (-1)  ...
  .* x4z))) .* (((x1x + (-1) .* x3x) .* ((x1x + (-1) .* x3x) .^ 2 +  ...
  (x1y + (-1) .* x3y) .^ 2 + (x1z + (-1) .* x3z) .^ 2) .^ (-1 / 2) + ...
   (x2x + (-1) .* x4x) .* ((x2x + (-1) .* x4x) .^ 2 + (x2y + (-1) .* ...
   x4y) .^ 2 + (x2z + (-1) .* x4z) .^ 2) .^ (-1 / 2)) .^ 2 + ((x1y + ...
   (-1) .* x3y) .* ((x1x + (-1) .* x3x) .^ 2 + (x1y + (-1) .* x3y)  ...
  .^ 2 + (x1z + (-1) .* x3z) .^ 2) .^ (-1 / 2) + (x2y + (-1) .* x4y) ...
   .* ((x2x + (-1) .* x4x) .^ 2 + (x2y + (-1) .* x4y) .^ 2 + (x2z +  ...
  (-1) .* x4z) .^ 2) .^ (-1 / 2)) .^ 2 + (((x1x + (-1) .* x3x) .^ 2  ...
  + (x1y + (-1) .* x3y) .^ 2 + (x1z + (-1) .* x3z) .^ 2) .^ (-1 / 2) ...
   .* (x1z + (-1) .* x3z) + ((x2x + (-1) .* x4x) .^ 2 + (x2y + (-1)  ...
  .* x4y) .^ 2 + (x2z + (-1) .* x4z) .^ 2) .^ (-1 / 2) .* (x2z + ( ...
  -1) .* x4z)) .^ 2) .^ (-3 / 2) .* (((-1) .* x1z + x3z) .* (x2y + ( ...
  -1) .* x4y) + (x1y + (-1) .* x3y) .* (x2z + (-1) .* x4z)) .* ((( ...
  x1x + (-1) .* x3x) .^ 2 + (x1y + (-1) .* x3y) .^ 2 + (x1z + (-1)  ...
  .* x3z) .^ 2) .^ (-1 / 2) .* (x1z + (-1) .* x3z) + ((x2x + (-1) .* ...
   x4x) .^ 2 + (x2y + (-1) .* x4y) .^ 2 + (x2z + (-1) .* x4z) .^ 2)  ...
  .^ (-1 / 2) .* (x2z + (-1) .* x4z)) + (1 / 2) .* ((((-1) .* x1y +  ...
  x3y) .* (x2x + (-1) .* x4x) + (x1x + (-1) .* x3x) .* (x2y + (-1)  ...
  .* x4y)) .^ 2 + ((x1z + (-1) .* x3z) .* (x2x + (-1) .* x4x) + (-1) ...
   .* (x1x + (-1) .* x3x) .* (x2z + (-1) .* x4z)) .^ 2 + (((-1) .*  ...
  x1z + x3z) .* (x2y + (-1) .* x4y) + (x1y + (-1) .* x3y) .* (x2z +  ...
  (-1) .* x4z)) .^ 2) .^ (-3 / 2) .* (((x1x + (-1) .* x3x) .* ((x1x  ...
  + (-1) .* x3x) .^ 2 + (x1y + (-1) .* x3y) .^ 2 + (x1z + (-1) .*  ...
  x3z) .^ 2) .^ (-1 / 2) + (x2x + (-1) .* x4x) .* ((x2x + (-1) .*  ...
  x4x) .^ 2 + (x2y + (-1) .* x4y) .^ 2 + (x2z + (-1) .* x4z) .^ 2)  ...
  .^ (-1 / 2)) .^ 2 + ((x1y + (-1) .* x3y) .* ((x1x + (-1) .* x3x)  ...
  .^ 2 + (x1y + (-1) .* x3y) .^ 2 + (x1z + (-1) .* x3z) .^ 2) .^ ( ...
  -1 / 2) + (x2y + (-1) .* x4y) .* ((x2x + (-1) .* x4x) .^ 2 + (x2y  ...
  + (-1) .* x4y) .^ 2 + (x2z + (-1) .* x4z) .^ 2) .^ (-1 / 2)) .^ 2  ...
  + (((x1x + (-1) .* x3x) .^ 2 + (x1y + (-1) .* x3y) .^ 2 + (x1z + ( ...
  -1) .* x3z) .^ 2) .^ (-1 / 2) .* (x1z + (-1) .* x3z) + ((x2x + ( ...
  -1) .* x4x) .^ 2 + (x2y + (-1) .* x4y) .^ 2 + (x2z + (-1) .* x4z)  ...
  .^ 2) .^ (-1 / 2) .* (x2z + (-1) .* x4z)) .^ 2) .^ (-1 / 2) .* ((( ...
  -1) .* x1z + x3z) .* (x2y + (-1) .* x4y) + (x1y + (-1) .* x3y) .*  ...
  (x2z + (-1) .* x4z)) .* (2 .* (((-1) .* x1y + x3y) .* (x2x + (-1)  ...
  .* x4x) + (x1x + (-1) .* x3x) .* (x2y + (-1) .* x4y)) .* ((-1) .*  ...
  x2y + x4y) + 2 .* ((x1z + (-1) .* x3z) .* (x2x + (-1) .* x4x) + ( ...
  -1) .* (x1x + (-1) .* x3x) .* (x2z + (-1) .* x4z)) .* (x2z + (-1)  ...
  .* x4z)) .* (((x1x + (-1) .* x3x) .^ 2 + (x1y + (-1) .* x3y) .^ 2  ...
  + (x1z + (-1) .* x3z) .^ 2) .^ (-1 / 2) .* (x1z + (-1) .* x3z) + ( ...
  (x2x + (-1) .* x4x) .^ 2 + (x2y + (-1) .* x4y) .^ 2 + (x2z + (-1)  ...
  .* x4z) .^ 2) .^ (-1 / 2) .* (x2z + (-1) .* x4z)),(x1x + (-1) .*  ...
  x3x) .* (x1y + (-1) .* x3y) .* ((x1x + (-1) .* x3x) .^ 2 + (x1y +  ...
  (-1) .* x3y) .^ 2 + (x1z + (-1) .* x3z) .^ 2) .^ (-3 / 2) .* ((( ...
  -1) .* x1y + x3y) .* (x2x + (-1) .* x4x) + (x1x + (-1) .* x3x) .*  ...
  (x2y + (-1) .* x4y)) .* ((((-1) .* x1y + x3y) .* (x2x + (-1) .*  ...
  x4x) + (x1x + (-1) .* x3x) .* (x2y + (-1) .* x4y)) .^ 2 + ((x1z +  ...
  (-1) .* x3z) .* (x2x + (-1) .* x4x) + (-1) .* (x1x + (-1) .* x3x)  ...
  .* (x2z + (-1) .* x4z)) .^ 2 + (((-1) .* x1z + x3z) .* (x2y + (-1) ...
   .* x4y) + (x1y + (-1) .* x3y) .* (x2z + (-1) .* x4z)) .^ 2) .^ ( ...
  -1 / 2) .* (((x1x + (-1) .* x3x) .* ((x1x + (-1) .* x3x) .^ 2 + ( ...
  x1y + (-1) .* x3y) .^ 2 + (x1z + (-1) .* x3z) .^ 2) .^ (-1 / 2) +  ...
  (x2x + (-1) .* x4x) .* ((x2x + (-1) .* x4x) .^ 2 + (x2y + (-1) .*  ...
  x4y) .^ 2 + (x2z + (-1) .* x4z) .^ 2) .^ (-1 / 2)) .^ 2 + ((x1y +  ...
  (-1) .* x3y) .* ((x1x + (-1) .* x3x) .^ 2 + (x1y + (-1) .* x3y)  ...
  .^ 2 + (x1z + (-1) .* x3z) .^ 2) .^ (-1 / 2) + (x2y + (-1) .* x4y) ...
   .* ((x2x + (-1) .* x4x) .^ 2 + (x2y + (-1) .* x4y) .^ 2 + (x2z +  ...
  (-1) .* x4z) .^ 2) .^ (-1 / 2)) .^ 2 + (((x1x + (-1) .* x3x) .^ 2  ...
  + (x1y + (-1) .* x3y) .^ 2 + (x1z + (-1) .* x3z) .^ 2) .^ (-1 / 2) ...
   .* (x1z + (-1) .* x3z) + ((x2x + (-1) .* x4x) .^ 2 + (x2y + (-1)  ...
  .* x4y) .^ 2 + (x2z + (-1) .* x4z) .^ 2) .^ (-1 / 2) .* (x2z + ( ...
  -1) .* x4z)) .^ 2) .^ (-1 / 2) + (-1 / 2) .* (((-1) .* x1y + x3y)  ...
  .* (x2x + (-1) .* x4x) + (x1x + (-1) .* x3x) .* (x2y + (-1) .*  ...
  x4y)) .* ((((-1) .* x1y + x3y) .* (x2x + (-1) .* x4x) + (x1x + ( ...
  -1) .* x3x) .* (x2y + (-1) .* x4y)) .^ 2 + ((x1z + (-1) .* x3z) .* ...
   (x2x + (-1) .* x4x) + (-1) .* (x1x + (-1) .* x3x) .* (x2z + (-1)  ...
  .* x4z)) .^ 2 + (((-1) .* x1z + x3z) .* (x2y + (-1) .* x4y) + ( ...
  x1y + (-1) .* x3y) .* (x2z + (-1) .* x4z)) .^ 2) .^ (-1 / 2) .* ( ...
  2 .* (x1x + (-1) .* x3x) .* (x1y + (-1) .* x3y) .* ((x1x + (-1) .* ...
   x3x) .^ 2 + (x1y + (-1) .* x3y) .^ 2 + (x1z + (-1) .* x3z) .^ 2)  ...
  .^ (-3 / 2) .* ((x1x + (-1) .* x3x) .* ((x1x + (-1) .* x3x) .^ 2 + ...
   (x1y + (-1) .* x3y) .^ 2 + (x1z + (-1) .* x3z) .^ 2) .^ (-1 / 2)  ...
  + (x2x + (-1) .* x4x) .* ((x2x + (-1) .* x4x) .^ 2 + (x2y + (-1)  ...
  .* x4y) .^ 2 + (x2z + (-1) .* x4z) .^ 2) .^ (-1 / 2)) + 2 .* (( ...
  x1y + (-1) .* x3y) .^ 2 .* ((x1x + (-1) .* x3x) .^ 2 + (x1y + (-1) ...
   .* x3y) .^ 2 + (x1z + (-1) .* x3z) .^ 2) .^ (-3 / 2) + (-1) .* (( ...
  x1x + (-1) .* x3x) .^ 2 + (x1y + (-1) .* x3y) .^ 2 + (x1z + (-1)  ...
  .* x3z) .^ 2) .^ (-1 / 2)) .* ((x1y + (-1) .* x3y) .* ((x1x + (-1) ...
   .* x3x) .^ 2 + (x1y + (-1) .* x3y) .^ 2 + (x1z + (-1) .* x3z) .^  ...
  2) .^ (-1 / 2) + (x2y + (-1) .* x4y) .* ((x2x + (-1) .* x4x) .^ 2  ...
  + (x2y + (-1) .* x4y) .^ 2 + (x2z + (-1) .* x4z) .^ 2) .^ (-1 / 2) ...
  ) + 2 .* (x1y + (-1) .* x3y) .* ((x1x + (-1) .* x3x) .^ 2 + (x1y + ...
   (-1) .* x3y) .^ 2 + (x1z + (-1) .* x3z) .^ 2) .^ (-3 / 2) .* ( ...
  x1z + (-1) .* x3z) .* (((x1x + (-1) .* x3x) .^ 2 + (x1y + (-1) .*  ...
  x3y) .^ 2 + (x1z + (-1) .* x3z) .^ 2) .^ (-1 / 2) .* (x1z + (-1)  ...
  .* x3z) + ((x2x + (-1) .* x4x) .^ 2 + (x2y + (-1) .* x4y) .^ 2 + ( ...
  x2z + (-1) .* x4z) .^ 2) .^ (-1 / 2) .* (x2z + (-1) .* x4z))) .* ( ...
  ((x1x + (-1) .* x3x) .* ((x1x + (-1) .* x3x) .^ 2 + (x1y + (-1) .* ...
   x3y) .^ 2 + (x1z + (-1) .* x3z) .^ 2) .^ (-1 / 2) + (x2x + (-1)  ...
  .* x4x) .* ((x2x + (-1) .* x4x) .^ 2 + (x2y + (-1) .* x4y) .^ 2 +  ...
  (x2z + (-1) .* x4z) .^ 2) .^ (-1 / 2)) .^ 2 + ((x1y + (-1) .* x3y) ...
   .* ((x1x + (-1) .* x3x) .^ 2 + (x1y + (-1) .* x3y) .^ 2 + (x1z +  ...
  (-1) .* x3z) .^ 2) .^ (-1 / 2) + (x2y + (-1) .* x4y) .* ((x2x + ( ...
  -1) .* x4x) .^ 2 + (x2y + (-1) .* x4y) .^ 2 + (x2z + (-1) .* x4z)  ...
  .^ 2) .^ (-1 / 2)) .^ 2 + (((x1x + (-1) .* x3x) .^ 2 + (x1y + (-1) ...
   .* x3y) .^ 2 + (x1z + (-1) .* x3z) .^ 2) .^ (-1 / 2) .* (x1z + ( ...
  -1) .* x3z) + ((x2x + (-1) .* x4x) .^ 2 + (x2y + (-1) .* x4y) .^  ...
  2 + (x2z + (-1) .* x4z) .^ 2) .^ (-1 / 2) .* (x2z + (-1) .* x4z))  ...
  .^ 2) .^ (-3 / 2) .* ((x1x + (-1) .* x3x) .* ((x1x + (-1) .* x3x)  ...
  .^ 2 + (x1y + (-1) .* x3y) .^ 2 + (x1z + (-1) .* x3z) .^ 2) .^ ( ...
  -1 / 2) + (x2x + (-1) .* x4x) .* ((x2x + (-1) .* x4x) .^ 2 + (x2y  ...
  + (-1) .* x4y) .^ 2 + (x2z + (-1) .* x4z) .^ 2) .^ (-1 / 2)) + ( ...
  x2x + (-1) .* x4x) .* ((((-1) .* x1y + x3y) .* (x2x + (-1) .* x4x) ...
   + (x1x + (-1) .* x3x) .* (x2y + (-1) .* x4y)) .^ 2 + ((x1z + (-1) ...
   .* x3z) .* (x2x + (-1) .* x4x) + (-1) .* (x1x + (-1) .* x3x) .* ( ...
  x2z + (-1) .* x4z)) .^ 2 + (((-1) .* x1z + x3z) .* (x2y + (-1) .*  ...
  x4y) + (x1y + (-1) .* x3y) .* (x2z + (-1) .* x4z)) .^ 2) .^ (-1 /  ...
  2) .* (((x1x + (-1) .* x3x) .* ((x1x + (-1) .* x3x) .^ 2 + (x1y +  ...
  (-1) .* x3y) .^ 2 + (x1z + (-1) .* x3z) .^ 2) .^ (-1 / 2) + (x2x + ...
   (-1) .* x4x) .* ((x2x + (-1) .* x4x) .^ 2 + (x2y + (-1) .* x4y)  ...
  .^ 2 + (x2z + (-1) .* x4z) .^ 2) .^ (-1 / 2)) .^ 2 + ((x1y + (-1)  ...
  .* x3y) .* ((x1x + (-1) .* x3x) .^ 2 + (x1y + (-1) .* x3y) .^ 2 +  ...
  (x1z + (-1) .* x3z) .^ 2) .^ (-1 / 2) + (x2y + (-1) .* x4y) .* (( ...
  x2x + (-1) .* x4x) .^ 2 + (x2y + (-1) .* x4y) .^ 2 + (x2z + (-1)  ...
  .* x4z) .^ 2) .^ (-1 / 2)) .^ 2 + (((x1x + (-1) .* x3x) .^ 2 + ( ...
  x1y + (-1) .* x3y) .^ 2 + (x1z + (-1) .* x3z) .^ 2) .^ (-1 / 2) .* ...
   (x1z + (-1) .* x3z) + ((x2x + (-1) .* x4x) .^ 2 + (x2y + (-1) .*  ...
  x4y) .^ 2 + (x2z + (-1) .* x4z) .^ 2) .^ (-1 / 2) .* (x2z + (-1)  ...
  .* x4z)) .^ 2) .^ (-1 / 2) .* ((x1x + (-1) .* x3x) .* ((x1x + (-1) ...
   .* x3x) .^ 2 + (x1y + (-1) .* x3y) .^ 2 + (x1z + (-1) .* x3z) .^  ...
